simulink model "kinovaMicoSimscapeModel"  (R2021b)
(part 37 of 50)

Y1_20_3=(dq2*dqr1*cos(2*q2)*sin(2*q3))/256 - (3*dq4*dqr1*sin(2*q4)*cos(q5))/64 - (3*dq5*dqr1*sin(2*q4)*cos(q5))/64 - (3*dq5*dqr1*sin(2*q6)*cos(q5))/64 - (3*dq6*dqr1*sin(2*q6)*cos(q5))/64 - (3*dq4*dqr1*sin(2*q4))/256 - (dq2*dqr1*cos(2*q3)*sin(2*q2))/256 - (dq3*dqr1*cos(2*q2)*sin(2*q3))/256 + (dq3*dqr1*cos(2*q3)*sin(2*q2))/256 + (3*dq4*dqr1*cos(2*q4)*sin(2*q5))/64 + (15*dq4*dqr1*cos(2*q5)*sin(2*q4))/256 - (27*dq4*dqr1*cos(2*q6)*sin(2*q4))/256 - (3*dq4*dqr1*cos(2*q4)*sin(2*q6)*cos(q5))/16 - (3*dq4*dqr1*cos(2*q6)*sin(2*q4)*cos(q5))/64 - (3*dq5*dqr1*cos(2*q4)*sin(2*q6)*cos(q5))/64 - (3*dq5*dqr1*cos(2*q6)*sin(2*q4)*cos(q5))/64 - (3*dq6*dqr1*cos(2*q4)*sin(2*q6)*cos(q5))/64 - (3*dq6*dqr1*cos(2*q6)*sin(2*q4)*cos(q5))/16 - (3*dq2*dqr1*cos(2*q2)*cos(2*q4)*sin(2*q3))/256 + (3*dq2*dqr1*cos(2*q3)*cos(2*q4)*sin(2*q2))/256 + (27*dq2*dqr1*cos(2*q2)*cos(2*q5)*sin(2*q3))/256 - (27*dq2*dqr1*cos(2*q3)*cos(2*q5)*sin(2*q2))/256 + (3*dq3*dqr1*cos(2*q2)*cos(2*q4)*sin(2*q3))/256 - (3*dq3*dqr1*cos(2*q3)*cos(2*q4)*sin(2*q2))/256 + (9*dq2*dqr1*cos(2*q2)*cos(2*q6)*sin(2*q3))/256 - (9*dq2*dqr1*cos(2*q3)*cos(2*q6)*sin(2*q2))/256 - (27*dq3*dqr1*cos(2*q2)*cos(2*q5)*sin(2*q3))/256 + (27*dq3*dqr1*cos(2*q3)*cos(2*q5)*sin(2*q2))/256 + (3*dq4*dqr1*cos(2*q2)*cos(2*q3)*sin(2*q4))/256 - (9*dq3*dqr1*cos(2*q2)*cos(2*q6)*sin(2*q3))/256 + (9*dq3*dqr1*cos(2*q3)*cos(2*q6)*sin(2*q2))/256 - (5*dq4*dqr1*cos(2*q4)*cos(2*q6)*sin(2*q5))/64 - (25*dq4*dqr1*cos(2*q5)*cos(2*q6)*sin(2*q4))/256 + (3*dq4*dqr1*sin(2*q2)*sin(2*q3)*sin(2*q4))/256 + (5*dq4*dqr1*sin(2*q4)*sin(2*q5)*sin(2*q6))/64 + (15*dq2*dqr1*cos(2*q2)*cos(2*q4)*cos(2*q5)*sin(2*q3))/256 - (15*dq2*dqr1*cos(2*q3)*cos(2*q4)*cos(2*q5)*sin(2*q2))/256 - (27*dq2*dqr1*cos(2*q2)*cos(2*q4)*cos(2*q6)*sin(2*q3))/256 + (27*dq2*dqr1*cos(2*q3)*cos(2*q4)*cos(2*q6)*sin(2*q2))/256 - (15*dq3*dqr1*cos(2*q2)*cos(2*q4)*cos(2*q5)*sin(2*q3))/256 + (15*dq3*dqr1*cos(2*q3)*cos(2*q4)*cos(2*q5)*sin(2*q2))/256 - (45*dq2*dqr1*cos(2*q2)*cos(2*q5)*cos(2*q6)*sin(2*q3))/256 + (45*dq2*dqr1*cos(2*q3)*cos(2*q5)*cos(2*q6)*sin(2*q2))/256 + (27*dq3*dqr1*cos(2*q2)*cos(2*q4)*cos(2*q6)*sin(2*q3))/256 - (27*dq3*dqr1*cos(2*q3)*cos(2*q4)*cos(2*q6)*sin(2*q2))/256 - (3*dq4*dqr1*cos(2*q2)*cos(2*q3)*cos(2*q4)*sin(2*q5))/64 - (15*dq4*dqr1*cos(2*q2)*cos(2*q3)*cos(2*q5)*sin(2*q4))/256 + (45*dq3*dqr1*cos(2*q2)*cos(2*q5)*cos(2*q6)*sin(2*q3))/256 - (45*dq3*dqr1*cos(2*q3)*cos(2*q5)*cos(2*q6)*sin(2*q2))/256 + (27*dq4*dqr1*cos(2*q2)*cos(2*q3)*cos(2*q6)*sin(2*q4))/256 - (3*dq2*dqr1*cos(2*q2)*sin(2*q3)*sin(2*q4)*sin(2*q5))/64 + (3*dq2*dqr1*cos(2*q3)*sin(2*q2)*sin(2*q4)*sin(2*q5))/64 + (3*dq3*dqr1*cos(2*q2)*sin(2*q3)*sin(2*q4)*sin(2*q5))/64 - (3*dq3*dqr1*cos(2*q3)*sin(2*q2)*sin(2*q4)*sin(2*q5))/64 + (9*dq2*dqr1*cos(2*q2)*sin(2*q3)*sin(2*q5)*sin(2*q6))/64 - (9*dq2*dqr1*cos(2*q3)*sin(2*q2)*sin(2*q5)*sin(2*q6))/64 - (3*dq4*dqr1*cos(2*q4)*sin(2*q2)*sin(2*q3)*sin(2*q5))/64 - (15*dq4*dqr1*cos(2*q5)*sin(2*q2)*sin(2*q3)*sin(2*q4))/256 - (9*dq3*dqr1*cos(2*q2)*sin(2*q3)*sin(2*q5)*sin(2*q6))/64 + (9*dq3*dqr1*cos(2*q3)*sin(2*q2)*sin(2*q5)*sin(2*q6))/64 + (27*dq4*dqr1*cos(2*q6)*sin(2*q2)*sin(2*q3)*sin(2*q4))/256 + (3*dq5*dqr1*cos(2*q2)*cos(2*q3)*sin(2*q4)*cos(q5))/64 - (9*dq5*dqr1*cos(2*q2)*cos(2*q3)*sin(2*q6)*cos(q5))/64 - (9*dq6*dqr1*cos(2*q2)*cos(2*q3)*sin(2*q6)*cos(q5))/64 + (3*dq5*dqr1*sin(2*q2)*sin(2*q3)*sin(2*q4)*cos(q5))/64 - (9*dq5*dqr1*sin(2*q2)*sin(2*q3)*sin(2*q6)*cos(q5))/64 - (9*dq6*dqr1*sin(2*q2)*sin(2*q3)*sin(2*q6)*cos(q5))/64 - (25*dq2*dqr1*cos(2*q2)*cos(2*q4)*cos(2*q5)*cos(2*q6)*sin(2*q3))/256 + (25*dq2*dqr1*cos(2*q3)*cos(2*q4)*cos(2*q5)*cos(2*q6)*sin(2*q2))/256 + (25*dq3*dqr1*cos(2*q2)*cos(2*q4)*cos(2*q5)*cos(2*q6)*sin(2*q3))/256 - (25*dq3*dqr1*cos(2*q3)*cos(2*q4)*cos(2*q5)*cos(2*q6)*sin(2*q2))/256 + (dq4*dqr1*cos(2*q2)*cos(2*q3)*cos(2*q4)*cos(2*q5)*sin(2*q6))/16 + (5*dq4*dqr1*cos(2*q2)*cos(2*q3)*cos(2*q4)*cos(2*q6)*sin(2*q5))/64 + (25*dq4*dqr1*cos(2*q2)*cos(2*q3)*cos(2*q5)*cos(2*q6)*sin(2*q4))/256 + (5*dq2*dqr1*cos(2*q2)*cos(2*q4)*sin(2*q3)*sin(2*q5)*sin(2*q6))/64 + (dq2*dqr1*cos(2*q2)*cos(2*q5)*sin(2*q3)*sin(2*q4)*sin(2*q6))/16 + (5*dq2*dqr1*cos(2*q2)*cos(2*q6)*sin(2*q3)*sin(2*q4)*sin(2*q5))/64 - (5*dq2*dqr1*cos(2*q3)*cos(2*q4)*sin(2*q2)*sin(2*q5)*sin(2*q6))/64 - (dq2*dqr1*cos(2*q3)*cos(2*q5)*sin(2*q2)*sin(2*q4)*sin(2*q6))/16 - (5*dq2*dqr1*cos(2*q3)*cos(2*q6)*sin(2*q2)*sin(2*q4)*sin(2*q5))/64 - (5*dq3*dqr1*cos(2*q2)*cos(2*q4)*sin(2*q3)*sin(2*q5)*sin(2*q6))/64 - (dq3*dqr1*cos(2*q2)*cos(2*q5)*sin(2*q3)*sin(2*q4)*sin(2*q6))/16 - (5*dq3*dqr1*cos(2*q2)*cos(2*q6)*sin(2*q3)*sin(2*q4)*sin(2*q5))/64 + (5*dq3*dqr1*cos(2*q3)*cos(2*q4)*sin(2*q2)*sin(2*q5)*sin(2*q6))/64 + (dq3*dqr1*cos(2*q3)*cos(2*q5)*sin(2*q2)*sin(2*q4)*sin(2*q6))/16 + (5*dq3*dqr1*cos(2*q3)*cos(2*q6)*sin(2*q2)*sin(2*q4)*sin(2*q5))/64 - (5*dq4*dqr1*cos(2*q2)*cos(2*q3)*sin(2*q4)*sin(2*q5)*sin(2*q6))/64 + (dq4*dqr1*cos(2*q4)*cos(2*q5)*sin(2*q2)*sin(2*q3)*sin(2*q6))/16 + (5*dq4*dqr1*cos(2*q4)*cos(2*q6)*sin(2*q2)*sin(2*q3)*sin(2*q5))/64 + (25*dq4*dqr1*cos(2*q5)*cos(2*q6)*sin(2*q2)*sin(2*q3)*sin(2*q4))/256 - (5*dq4*dqr1*sin(2*q2)*sin(2*q3)*sin(2*q4)*sin(2*q5)*sin(2*q6))/64 + (3*dq4*dqr1*cos(2*q2)*cos(2*q3)*cos(2*q4)*sin(2*q6)*cos(q5))/16 + (3*dq5*dqr1*cos(2*q2)*cos(2*q3)*cos(2*q4)*sin(2*q6)*cos(q5))/64 + (3*dq5*dqr1*cos(2*q2)*cos(2*q3)*cos(2*q6)*sin(2*q4)*cos(q5))/64 + (3*dq6*dqr1*cos(2*q2)*cos(2*q3)*cos(2*q4)*sin(2*q6)*cos(q5))/64 + (3*dq6*dqr1*cos(2*q2)*cos(2*q3)*cos(2*q6)*sin(2*q4)*cos(q5))/16 + (3*dq5*dqr1*cos(2*q4)*sin(2*q2)*sin(2*q3)*sin(2*q6)*cos(q5))/64 + (3*dq5*dqr1*cos(2*q6)*sin(2*q2)*sin(2*q3)*sin(2*q4)*cos(q5))/64 + (3*dq6*dqr1*cos(2*q4)*sin(2*q2)*sin(2*q3)*sin(2*q6)*cos(q5))/64 + (3*dq6*dqr1*cos(2*q6)*sin(2*q2)*sin(2*q3)*sin(2*q4)*cos(q5))/16;
Y1_20_4=(15*dq5*dqr1*cos(2*q4)*sin(2*q5))/256 - (3*dq6*dqr1*sin(2*q6))/256 - (9*dq5*dqr1*sin(2*q5))/256 + (3*dq5*dqr1*cos(2*q5)*sin(2*q4))/64 + (3*dq5*dqr1*cos(2*q5)*sin(2*q6))/64 + (15*dq5*dqr1*cos(2*q6)*sin(2*q5))/256 - (27*dq6*dqr1*cos(2*q4)*sin(2*q6))/256 + (15*dq6*dqr1*cos(2*q5)*sin(2*q6))/256 + (3*dq6*dqr1*cos(2*q6)*sin(2*q5))/64 - (3*dq2*dqr2*sin(2*q4)*sin(q2)*sin(q3))/128 + (3*dq3*dqr2*sin(2*q4)*sin(q2)*sin(q3))/128 - (27*dq5*dqr1*cos(2*q2)*cos(2*q3)*sin(2*q5))/256 - (9*dq6*dqr1*cos(2*q2)*cos(2*q3)*sin(2*q6))/256 - (dq4*dqr1*cos(2*q4)*cos(2*q5)*sin(2*q6))/16 - (5*dq5*dqr1*cos(2*q4)*cos(2*q5)*sin(2*q6))/64 - (25*dq5*dqr1*cos(2*q4)*cos(2*q6)*sin(2*q5))/256 - (5*dq5*dqr1*cos(2*q5)*cos(2*q6)*sin(2*q4))/64 - (25*dq6*dqr1*cos(2*q4)*cos(2*q5)*sin(2*q6))/256 - (5*dq6*dqr1*cos(2*q4)*cos(2*q6)*sin(2*q5))/64 - (dq6*dqr1*cos(2*q5)*cos(2*q6)*sin(2*q4))/16 - (27*dq5*dqr1*sin(2*q2)*sin(2*q3)*sin(2*q5))/256 - (9*dq6*dqr1*sin(2*q2)*sin(2*q3)*sin(2*q6))/256 + (dq5*dqr1*sin(2*q4)*sin(2*q5)*sin(2*q6))/16 + (5*dq6*dqr1*sin(2*q4)*sin(2*q5)*sin(2*q6))/64 - (15*dq5*dqr1*cos(2*q2)*cos(2*q3)*cos(2*q4)*sin(2*q5))/256 - (3*dq5*dqr1*cos(2*q2)*cos(2*q3)*cos(2*q5)*sin(2*q4))/64 + (9*dq5*dqr1*cos(2*q2)*cos(2*q3)*cos(2*q5)*sin(2*q6))/64 + (45*dq5*dqr1*cos(2*q2)*cos(2*q3)*cos(2*q6)*sin(2*q5))/256 + (27*dq6*dqr1*cos(2*q2)*cos(2*q3)*cos(2*q4)*sin(2*q6))/256 + (45*dq6*dqr1*cos(2*q2)*cos(2*q3)*cos(2*q5)*sin(2*q6))/256 + (9*dq6*dqr1*cos(2*q2)*cos(2*q3)*cos(2*q6)*sin(2*q5))/64 - (3*dq2*dqr2*cos(2*q4)*sin(q2)*sin(q3)*sin(q5))/16 - (3*dq2*dqr2*sin(2*q4)*cos(q5)*sin(q2)*sin(q3))/32 + (3*dq3*dqr2*cos(2*q4)*sin(q2)*sin(q3)*sin(q5))/16 + (3*dq3*dqr2*sin(2*q4)*cos(q5)*sin(q2)*sin(q3))/32 - (15*dq5*dqr1*cos(2*q4)*sin(2*q2)*sin(2*q3)*sin(2*q5))/256 - (3*dq5*dqr1*cos(2*q5)*sin(2*q2)*sin(2*q3)*sin(2*q4))/64 + (9*dq5*dqr1*cos(2*q5)*sin(2*q2)*sin(2*q3)*sin(2*q6))/64 + (45*dq5*dqr1*cos(2*q6)*sin(2*q2)*sin(2*q3)*sin(2*q5))/256 + (27*dq6*dqr1*cos(2*q4)*sin(2*q2)*sin(2*q3)*sin(2*q6))/256 + (45*dq6*dqr1*cos(2*q5)*sin(2*q2)*sin(2*q3)*sin(2*q6))/256 + (9*dq6*dqr1*cos(2*q6)*sin(2*q2)*sin(2*q3)*sin(2*q5))/64 + (5*3^(1/2)*dq5*dqr2*sin(q2)*sin(q3)*sin(q4))/32 + (3^(1/2)*dq6*dqr2*sin(q2)*sin(q3)*sin(q4))/8 + (3*dq2*dqr2*cos(2*q4)*sin(2*q5)*sin(q2)*sin(q3))/32 + (15*dq2*dqr2*cos(2*q5)*sin(2*q4)*sin(q2)*sin(q3))/128 - (27*dq2*dqr2*cos(2*q6)*sin(2*q4)*sin(q2)*sin(q3))/128 - (15*dq3*dqr2*cos(2*q5)*sin(2*q4)*sin(q2)*sin(q3))/128 + (27*dq3*dqr2*cos(2*q6)*sin(2*q4)*sin(q2)*sin(q3))/128 - (3*3^(1/2)*dq5*dqr2*cos(q4)*sin(q2)*sin(q3)*sin(q5))/32 - (3^(1/2)*dq6*dqr2*cos(q4)*sin(q2)*sin(q3)*sin(q5))/4 - (3^(1/2)*dq6*dqr2*cos(q5)*sin(q2)*sin(q3)*sin(q4))/8 + (5*dq5*dqr1*cos(2*q2)*cos(2*q3)*cos(2*q4)*cos(2*q5)*sin(2*q6))/64 + (25*dq5*dqr1*cos(2*q2)*cos(2*q3)*cos(2*q4)*cos(2*q6)*sin(2*q5))/256 + (5*dq5*dqr1*cos(2*q2)*cos(2*q3)*cos(2*q5)*cos(2*q6)*sin(2*q4))/64 + (25*dq6*dqr1*cos(2*q2)*cos(2*q3)*cos(2*q4)*cos(2*q5)*sin(2*q6))/256 + (5*dq6*dqr1*cos(2*q2)*cos(2*q3)*cos(2*q4)*cos(2*q6)*sin(2*q5))/64 + (dq6*dqr1*cos(2*q2)*cos(2*q3)*cos(2*q5)*cos(2*q6)*sin(2*q4))/16 - (3*dq2*dqr2*cos(2*q4)*cos(2*q6)*sin(q2)*sin(q3)*sin(q5))/16 - (3*dq2*dqr2*cos(2*q4)*sin(2*q6)*cos(q5)*sin(q2)*sin(q3))/8 - (3*dq2*dqr2*cos(2*q6)*sin(2*q4)*cos(q5)*sin(q2)*sin(q3))/32 + (3*dq3*dqr2*cos(2*q4)*cos(2*q6)*sin(q2)*sin(q3)*sin(q5))/16 + (3*dq3*dqr2*cos(2*q4)*sin(2*q6)*cos(q5)*sin(q2)*sin(q3))/8 + (3*dq3*dqr2*cos(2*q6)*sin(2*q4)*cos(q5)*sin(q2)*sin(q3))/32 - (dq5*dqr1*cos(2*q2)*cos(2*q3)*sin(2*q4)*sin(2*q5)*sin(2*q6))/16 + (5*dq5*dqr1*cos(2*q4)*cos(2*q5)*sin(2*q2)*sin(2*q3)*sin(2*q6))/64 + (25*dq5*dqr1*cos(2*q4)*cos(2*q6)*sin(2*q2)*sin(2*q3)*sin(2*q5))/256 + (5*dq5*dqr1*cos(2*q5)*cos(2*q6)*sin(2*q2)*sin(2*q3)*sin(2*q4))/64 - (5*dq6*dqr1*cos(2*q2)*cos(2*q3)*sin(2*q4)*sin(2*q5)*sin(2*q6))/64 + (25*dq6*dqr1*cos(2*q4)*cos(2*q5)*sin(2*q2)*sin(2*q3)*sin(2*q6))/256 + (5*dq6*dqr1*cos(2*q4)*cos(2*q6)*sin(2*q2)*sin(2*q3)*sin(2*q5))/64 + (dq6*dqr1*cos(2*q5)*cos(2*q6)*sin(2*q2)*sin(2*q3)*sin(2*q4))/16 + (3*dq2*dqr2*sin(2*q4)*sin(2*q6)*sin(q2)*sin(q3)*sin(q5))/16 - (3*dq3*dqr2*sin(2*q4)*sin(2*q6)*sin(q2)*sin(q3)*sin(q5))/16 + (3*3^(1/2)*dq5*dqr2*cos(2*q5)*sin(q2)*sin(q3)*sin(q4))/32 + (3*3^(1/2)*dq5*dqr2*sin(2*q5)*cos(q4)*sin(q2)*sin(q3))/64 - (3*3^(1/2)*dq5*dqr2*cos(2*q6)*sin(q2)*sin(q3)*sin(q4))/32 + (9*3^(1/2)*dq6*dqr2*sin(2*q6)*cos(q4)*sin(q2)*sin(q3))/64 - (dq5*dqr1*sin(2*q2)*sin(2*q3)*sin(2*q4)*sin(2*q5)*sin(2*q6))/16 - (5*dq6*dqr1*sin(2*q2)*sin(2*q3)*sin(2*q4)*sin(2*q5)*sin(2*q6))/64 - (dq2*dqr2*cos(2*q4)*cos(2*q5)*sin(2*q6)*sin(q2)*sin(q3))/8 - (5*dq2*dqr2*cos(2*q4)*cos(2*q6)*sin(2*q5)*sin(q2)*sin(q3))/32 - (25*dq2*dqr2*cos(2*q5)*cos(2*q6)*sin(2*q4)*sin(q2)*sin(q3))/128 + (25*dq3*dqr2*cos(2*q5)*cos(2*q6)*sin(2*q4)*sin(q2)*sin(q3))/128 + (5*dq2*dqr2*sin(2*q4)*sin(2*q5)*sin(2*q6)*sin(q2)*sin(q3))/32 - (5*dq3*dqr2*sin(2*q4)*sin(2*q5)*sin(2*q6)*sin(q2)*sin(q3))/32 - (3*3^(1/2)*dq5*dqr2*cos(2*q6)*cos(q4)*sin(q2)*sin(q3)*sin(q5))/32 - (3*3^(1/2)*dq5*dqr2*sin(2*q6)*cos(q4)*cos(q5)*sin(q2)*sin(q3))/16 - (3^(1/2)*dq6*dqr2*cos(2*q6)*cos(q4)*sin(q2)*sin(q3)*sin(q5))/8 + (3^(1/2)*dq6*dqr2*cos(2*q6)*cos(q5)*sin(q2)*sin(q3)*sin(q4))/8 - (3^(1/2)*dq6*dqr2*sin(2*q6)*cos(q4)*cos(q5)*sin(q2)*sin(q3))/16 - (3^(1/2)*dq6*dqr2*sin(2*q6)*sin(q2)*sin(q3)*sin(q4)*sin(q5))/16 - (5*3^(1/2)*dq5*dqr2*cos(2*q5)*cos(2*q6)*sin(q2)*sin(q3)*sin(q4))/32 - (3^(1/2)*dq5*dqr2*cos(2*q5)*sin(2*q6)*cos(q4)*sin(q2)*sin(q3))/16 - (5*3^(1/2)*dq5*dqr2*cos(2*q6)*sin(2*q5)*cos(q4)*sin(q2)*sin(q3))/64 - (3^(1/2)*dq6*dqr2*cos(2*q5)*cos(2*q6)*sin(q2)*sin(q3)*sin(q4))/8 - (5*3^(1/2)*dq6*dqr2*cos(2*q5)*sin(2*q6)*cos(q4)*sin(q2)*sin(q3))/64 - (3^(1/2)*dq6*dqr2*cos(2*q6)*sin(2*q5)*cos(q4)*sin(q2)*sin(q3))/16 + (3^(1/2)*dq5*dqr2*sin(2*q5)*sin(2*q6)*sin(q2)*sin(q3)*sin(q4))/8 + (5*3^(1/2)*dq6*dqr2*sin(2*q5)*sin(2*q6)*sin(q2)*sin(q3)*sin(q4))/32;
Y1_20_5=(3*dq5*dqr2*cos(2*q6)*cos(q3)*sin(q2))/32 - (5*dq5*dqr2*cos(q3)*sin(q2))/32 - (dq6*dqr2*cos(q3)*sin(q2))/8 - (3*dq4*dqr2*cos(2*q4)*cos(q3)*sin(q2))/128 - (9*dq4*dqr2*cos(2*q5)*cos(q3)*sin(q2))/128 - (3*dq4*dqr2*cos(2*q6)*cos(q3)*sin(q2))/128 - (43*dq4*dqr2*cos(q3)*sin(q2))/128 - (3*dq4*dqr2*cos(q3)*cos(q5)*sin(q2))/32 - (3*dq5*dqr2*cos(q3)*cos(q5)*sin(q2))/32 - (3*dq6*dqr2*cos(q3)*cos(q5)*sin(q2))/8 - (3*dq4*dqr2*sin(2*q4)*cos(q2)*sin(q3)*sin(q5))/16 + (3*dq4*dqr2*sin(2*q4)*cos(q3)*sin(q2)*sin(q5))/16 + (3*dq5*dqr2*sin(2*q4)*cos(q3)*sin(q2)*sin(q5))/64 - (3*dq4*dqr2*sin(2*q6)*cos(q2)*sin(q3)*sin(q5))/16 + (3*dq4*dqr2*sin(2*q6)*cos(q3)*sin(q2)*sin(q5))/16 + (3*dq5*dqr2*sin(2*q6)*cos(q3)*sin(q2)*sin(q5))/16 + (3^(1/2)*dq2*dqr2*cos(q3)*cos(q4)*sin(q2))/64 - (3^(1/2)*dq3*dqr2*cos(q3)*cos(q4)*sin(q2))/64 + (15*dq4*dqr2*cos(2*q4)*cos(2*q5)*cos(q3)*sin(q2))/128 - (27*dq4*dqr2*cos(2*q4)*cos(2*q6)*cos(q3)*sin(q2))/128 + (3*dq5*dqr2*cos(2*q4)*cos(2*q5)*cos(q3)*sin(q2))/32 + (15*dq4*dqr2*cos(2*q5)*cos(2*q6)*cos(q3)*sin(q2))/128 - (3*dq3*dqr2*cos(2*q4)*sin(2*q5)*sin(q2)*sin(q3))/32 - (3*dq4*dqr2*sin(2*q4)*sin(2*q5)*cos(q3)*sin(q2))/32 - (15*dq5*dqr2*sin(2*q4)*sin(2*q5)*cos(q3)*sin(q2))/128 - (3*dq4*dqr2*sin(2*q5)*sin(2*q6)*cos(q3)*sin(q2))/32 + (27*dq6*dqr2*sin(2*q4)*sin(2*q6)*cos(q3)*sin(q2))/128 - (3*dq4*dqr2*cos(2*q4)*cos(q3)*cos(q5)*sin(q2))/32 - (3*dq5*dqr2*cos(2*q4)*cos(q3)*cos(q5)*sin(q2))/32 - (3*dq4*dqr2*cos(2*q6)*cos(q3)*cos(q5)*sin(q2))/32 - (3*dq5*dqr2*cos(2*q6)*cos(q3)*cos(q5)*sin(q2))/32 + (3^(1/2)*dq2*dqr2*cos(q2)*sin(q3)*sin(q4)*sin(q5))/16 - (3^(1/2)*dq2*dqr2*cos(q3)*sin(q2)*sin(q4)*sin(q5))/16 - (3^(1/2)*dq3*dqr2*cos(q2)*sin(q3)*sin(q4)*sin(q5))/16 + (3^(1/2)*dq3*dqr2*cos(q3)*sin(q2)*sin(q4)*sin(q5))/16 - (3*dq4*dqr2*cos(2*q4)*cos(2*q6)*cos(q3)*cos(q5)*sin(q2))/32 - (3*dq5*dqr2*cos(2*q4)*cos(2*q6)*cos(q3)*cos(q5)*sin(q2))/32 - (3*dq6*dqr2*cos(2*q4)*cos(2*q6)*cos(q3)*cos(q5)*sin(q2))/8 - (3*dq4*dqr2*cos(2*q4)*sin(2*q6)*cos(q2)*sin(q3)*sin(q5))/16 + (3*dq4*dqr2*cos(2*q4)*sin(2*q6)*cos(q3)*sin(q2)*sin(q5))/16 - (3*dq4*dqr2*cos(2*q6)*sin(2*q4)*cos(q2)*sin(q3)*sin(q5))/16 + (3*dq4*dqr2*cos(2*q6)*sin(2*q4)*cos(q3)*sin(q2)*sin(q5))/16 + (3*dq4*dqr2*sin(2*q4)*sin(2*q6)*cos(q3)*cos(q5)*sin(q2))/8 + (3*dq5*dqr2*cos(2*q4)*sin(2*q6)*cos(q3)*sin(q2)*sin(q5))/16 - (3*dq5*dqr2*cos(2*q6)*sin(2*q4)*cos(q2)*sin(q3)*sin(q5))/64 + (3*dq5*dqr2*cos(2*q6)*sin(2*q4)*cos(q3)*sin(q2)*sin(q5))/64 + (3*dq5*dqr2*sin(2*q4)*sin(2*q6)*cos(q3)*cos(q5)*sin(q2))/32 + (3*dq6*dqr2*cos(2*q4)*sin(2*q6)*cos(q3)*sin(q2)*sin(q5))/16 + (3*dq6*dqr2*cos(2*q6)*sin(2*q4)*cos(q3)*sin(q2)*sin(q5))/16 + (3*dq6*dqr2*sin(2*q4)*sin(2*q6)*cos(q3)*cos(q5)*sin(q2))/32 + (3*3^(1/2)*dq2*dqr2*cos(2*q5)*cos(q3)*cos(q4)*sin(q2))/64 + (9*3^(1/2)*dq2*dqr2*cos(2*q6)*cos(q3)*cos(q4)*sin(q2))/64 - (3*3^(1/2)*dq3*dqr2*cos(2*q5)*cos(q3)*cos(q4)*sin(q2))/64 - (9*3^(1/2)*dq3*dqr2*cos(2*q6)*cos(q3)*cos(q4)*sin(q2))/64 + (3*3^(1/2)*dq2*dqr2*sin(2*q5)*cos(q2)*sin(q3)*sin(q4))/32 - (3*3^(1/2)*dq2*dqr2*sin(2*q5)*cos(q3)*sin(q2)*sin(q4))/32 - (3*3^(1/2)*dq3*dqr2*sin(2*q5)*cos(q2)*sin(q3)*sin(q4))/32 + (3*3^(1/2)*dq3*dqr2*sin(2*q5)*cos(q3)*sin(q2)*sin(q4))/32 - (25*dq4*dqr2*cos(2*q4)*cos(2*q5)*cos(2*q6)*cos(q3)*sin(q2))/128 - (5*dq5*dqr2*cos(2*q4)*cos(2*q5)*cos(2*q6)*cos(q3)*sin(q2))/32 - (dq6*dqr2*cos(2*q4)*cos(2*q5)*cos(2*q6)*cos(q3)*sin(q2))/8 + (dq3*dqr2*cos(2*q4)*cos(2*q5)*sin(2*q6)*sin(q2)*sin(q3))/8 + (5*dq3*dqr2*cos(2*q4)*cos(2*q6)*sin(2*q5)*sin(q2)*sin(q3))/32 + (5*dq4*dqr2*cos(2*q4)*sin(2*q5)*sin(2*q6)*cos(q3)*sin(q2))/32 + (dq4*dqr2*cos(2*q5)*sin(2*q4)*sin(2*q6)*cos(q3)*sin(q2))/8 + (5*dq4*dqr2*cos(2*q6)*sin(2*q4)*sin(2*q5)*cos(q3)*sin(q2))/32 + (dq5*dqr2*cos(2*q4)*sin(2*q5)*sin(2*q6)*cos(q3)*sin(q2))/8 + (5*dq5*dqr2*cos(2*q5)*sin(2*q4)*sin(2*q6)*cos(q3)*sin(q2))/32 + (25*dq5*dqr2*cos(2*q6)*sin(2*q4)*sin(2*q5)*cos(q3)*sin(q2))/128 + (5*dq6*dqr2*cos(2*q4)*sin(2*q5)*sin(2*q6)*cos(q3)*sin(q2))/32 + (25*dq6*dqr2*cos(2*q5)*sin(2*q4)*sin(2*q6)*cos(q3)*sin(q2))/128 + (5*dq6*dqr2*cos(2*q6)*sin(2*q4)*sin(2*q5)*cos(q3)*sin(q2))/32 - (3^(1/2)*dq2*dqr2*cos(q3)*cos(q4)*cos(q5)*sin(q2))/16 + (3^(1/2)*dq3*dqr2*cos(q3)*cos(q4)*cos(q5)*sin(q2))/16 - (3^(1/2)*dq2*dqr2*cos(2*q6)*cos(q3)*cos(q4)*cos(q5)*sin(q2))/16 + (3^(1/2)*dq3*dqr2*cos(2*q6)*cos(q3)*cos(q4)*cos(q5)*sin(q2))/16 + (3^(1/2)*dq2*dqr2*cos(2*q6)*cos(q2)*sin(q3)*sin(q4)*sin(q5))/16 - (3^(1/2)*dq2*dqr2*cos(2*q6)*cos(q3)*sin(q2)*sin(q4)*sin(q5))/16 - (3^(1/2)*dq2*dqr2*sin(2*q6)*cos(q2)*cos(q4)*sin(q3)*sin(q5))/8 + (3^(1/2)*dq2*dqr2*sin(2*q6)*cos(q2)*cos(q5)*sin(q3)*sin(q4))/8 + (3^(1/2)*dq2*dqr2*sin(2*q6)*cos(q3)*cos(q4)*sin(q2)*sin(q5))/8 - (3^(1/2)*dq2*dqr2*sin(2*q6)*cos(q3)*cos(q5)*sin(q2)*sin(q4))/8 - (3^(1/2)*dq3*dqr2*cos(2*q6)*cos(q2)*sin(q3)*sin(q4)*sin(q5))/16 + (3^(1/2)*dq3*dqr2*cos(2*q6)*cos(q3)*sin(q2)*sin(q4)*sin(q5))/16 + (3^(1/2)*dq3*dqr2*sin(2*q6)*cos(q2)*cos(q4)*sin(q3)*sin(q5))/8 - (3^(1/2)*dq3*dqr2*sin(2*q6)*cos(q2)*cos(q5)*sin(q3)*sin(q4))/8 - (3^(1/2)*dq3*dqr2*sin(2*q6)*cos(q3)*cos(q4)*sin(q2)*sin(q5))/8 + (3^(1/2)*dq3*dqr2*sin(2*q6)*cos(q3)*cos(q5)*sin(q2)*sin(q4))/8 - (5*3^(1/2)*dq2*dqr2*cos(2*q5)*cos(2*q6)*cos(q3)*cos(q4)*sin(q2))/64 + (5*3^(1/2)*dq3*dqr2*cos(2*q5)*cos(2*q6)*cos(q3)*cos(q4)*sin(q2))/64 - (3^(1/2)*dq2*dqr2*cos(2*q5)*sin(2*q6)*cos(q2)*sin(q3)*sin(q4))/8 + (3^(1/2)*dq2*dqr2*cos(2*q5)*sin(2*q6)*cos(q3)*sin(q2)*sin(q4))/8 - (5*3^(1/2)*dq2*dqr2*cos(2*q6)*sin(2*q5)*cos(q2)*sin(q3)*sin(q4))/32 + (5*3^(1/2)*dq2*dqr2*cos(2*q6)*sin(2*q5)*cos(q3)*sin(q2)*sin(q4))/32 + (3^(1/2)*dq2*dqr2*sin(2*q5)*sin(2*q6)*cos(q3)*cos(q4)*sin(q2))/16 + (3^(1/2)*dq3*dqr2*cos(2*q5)*sin(2*q6)*cos(q2)*sin(q3)*sin(q4))/8 - (3^(1/2)*dq3*dqr2*cos(2*q5)*sin(2*q6)*cos(q3)*sin(q2)*sin(q4))/8 + (5*3^(1/2)*dq3*dqr2*cos(2*q6)*sin(2*q5)*cos(q2)*sin(q3)*sin(q4))/32 - (5*3^(1/2)*dq3*dqr2*cos(2*q6)*sin(2*q5)*cos(q3)*sin(q2)*sin(q4))/32 - (3^(1/2)*dq3*dqr2*sin(2*q5)*sin(2*q6)*cos(q3)*cos(q4)*sin(q2))/16;
Y1_20_6=(43*dq4*dqr2*cos(q2)*sin(q3))/128 + (5*dq5*dqr2*cos(q2)*sin(q3))/32 + (dq6*dqr2*cos(q2)*sin(q3))/8 + (3*dq4*dqr2*cos(2*q4)*cos(q2)*sin(q3))/128 + (9*dq4*dqr2*cos(2*q5)*cos(q2)*sin(q3))/128 + (3*dq4*dqr2*cos(2*q6)*cos(q2)*sin(q3))/128 - (3*dq5*dqr2*cos(2*q6)*cos(q2)*sin(q3))/32 + (3*dq4*dqr2*cos(q2)*cos(q5)*sin(q3))/32 + (3*dq5*dqr2*cos(q2)*cos(q5)*sin(q3))/32 + (3*dq6*dqr2*cos(q2)*cos(q5)*sin(q3))/8 - (3*dq5*dqr2*sin(2*q4)*cos(q2)*sin(q3)*sin(q5))/64 - (3*dq5*dqr2*sin(2*q6)*cos(q2)*sin(q3)*sin(q5))/16 - (3^(1/2)*dq2*dqr2*cos(q2)*cos(q4)*sin(q3))/64 + (3^(1/2)*dq3*dqr2*cos(q2)*cos(q4)*sin(q3))/64 + (5*3^(1/2)*dq5*dqr2*cos(q2)*cos(q3)*sin(q4))/32 + (3^(1/2)*dq6*dqr2*cos(q2)*cos(q3)*sin(q4))/8 - (15*dq4*dqr2*cos(2*q4)*cos(2*q5)*cos(q2)*sin(q3))/128 + (27*dq4*dqr2*cos(2*q4)*cos(2*q6)*cos(q2)*sin(q3))/128 - (3*dq5*dqr2*cos(2*q4)*cos(2*q5)*cos(q2)*sin(q3))/32 - (15*dq4*dqr2*cos(2*q5)*cos(2*q6)*cos(q2)*sin(q3))/128 + (3*dq4*dqr2*sin(2*q4)*sin(2*q5)*cos(q2)*sin(q3))/32 + (15*dq5*dqr2*sin(2*q4)*sin(2*q5)*cos(q2)*sin(q3))/128 + (3*dq4*dqr2*sin(2*q5)*sin(2*q6)*cos(q2)*sin(q3))/32 - (27*dq6*dqr2*sin(2*q4)*sin(2*q6)*cos(q2)*sin(q3))/128 - (3^(1/2)*dq1*dqr2*cos(2*q2)*cos(2*q3)*sin(q4))/64 - (3*dq2*dqr2*cos(2*q4)*cos(q2)*cos(q3)*sin(q5))/16 + (3*dq3*dqr2*cos(2*q4)*cos(q2)*cos(q3)*sin(q5))/16 + (3*dq4*dqr2*cos(2*q4)*cos(q2)*cos(q5)*sin(q3))/32 + (3*dq5*dqr2*cos(2*q4)*cos(q2)*cos(q5)*sin(q3))/32 + (3*dq4*dqr2*cos(2*q6)*cos(q2)*cos(q5)*sin(q3))/32 + (3*dq5*dqr2*cos(2*q6)*cos(q2)*cos(q5)*sin(q3))/32 - (3^(1/2)*dq1*dqr2*sin(2*q2)*sin(2*q3)*sin(q4))/64 - (3*3^(1/2)*dq1*dqr2*cos(2*q2)*cos(2*q3)*cos(2*q5)*sin(q4))/64 - (9*3^(1/2)*dq1*dqr2*cos(2*q2)*cos(2*q3)*cos(2*q6)*sin(q4))/64 - (3*dq2*dqr2*cos(2*q4)*cos(2*q6)*cos(q2)*cos(q3)*sin(q5))/16 + (3*dq3*dqr2*cos(2*q4)*cos(2*q6)*cos(q2)*cos(q3)*sin(q5))/16 + (3*dq4*dqr2*cos(2*q4)*cos(2*q6)*cos(q2)*cos(q5)*sin(q3))/32 + (3*dq5*dqr2*cos(2*q4)*cos(2*q6)*cos(q2)*cos(q5)*sin(q3))/32 + (3*dq6*dqr2*cos(2*q4)*cos(2*q6)*cos(q2)*cos(q5)*sin(q3))/8 - (3*3^(1/2)*dq1*dqr2*cos(2*q5)*sin(2*q2)*sin(2*q3)*sin(q4))/64 - (9*3^(1/2)*dq1*dqr2*cos(2*q6)*sin(2*q2)*sin(2*q3)*sin(q4))/64 + (3*dq2*dqr2*sin(2*q4)*sin(2*q6)*cos(q2)*cos(q3)*sin(q5))/16 - (3*dq3*dqr2*sin(2*q4)*sin(2*q6)*cos(q2)*cos(q3)*sin(q5))/16 - (3*dq4*dqr2*sin(2*q4)*sin(2*q6)*cos(q2)*cos(q5)*sin(q3))/8 - (3*dq5*dqr2*cos(2*q4)*sin(2*q6)*cos(q2)*sin(q3)*sin(q5))/16 - (3*dq5*dqr2*sin(2*q4)*sin(2*q6)*cos(q2)*cos(q5)*sin(q3))/32 - (3*dq6*dqr2*cos(2*q4)*sin(2*q6)*cos(q2)*sin(q3)*sin(q5))/16 - (3*dq6*dqr2*cos(2*q6)*sin(2*q4)*cos(q2)*sin(q3)*sin(q5))/16 - (3*dq6*dqr2*sin(2*q4)*sin(2*q6)*cos(q2)*cos(q5)*sin(q3))/32 - (3*3^(1/2)*dq2*dqr2*cos(2*q5)*cos(q2)*cos(q4)*sin(q3))/64 - (9*3^(1/2)*dq2*dqr2*cos(2*q6)*cos(q2)*cos(q4)*sin(q3))/64 + (3*3^(1/2)*dq3*dqr2*cos(2*q5)*cos(q2)*cos(q4)*sin(q3))/64 + (9*3^(1/2)*dq3*dqr2*cos(2*q6)*cos(q2)*cos(q4)*sin(q3))/64 + (3*3^(1/2)*dq5*dqr2*cos(2*q5)*cos(q2)*cos(q3)*sin(q4))/32 - (3*3^(1/2)*dq5*dqr2*cos(2*q6)*cos(q2)*cos(q3)*sin(q4))/32 + (25*dq4*dqr2*cos(2*q4)*cos(2*q5)*cos(2*q6)*cos(q2)*sin(q3))/128 + (5*dq5*dqr2*cos(2*q4)*cos(2*q5)*cos(2*q6)*cos(q2)*sin(q3))/32 + (dq6*dqr2*cos(2*q4)*cos(2*q5)*cos(2*q6)*cos(q2)*sin(q3))/8 - (5*dq4*dqr2*cos(2*q4)*sin(2*q5)*sin(2*q6)*cos(q2)*sin(q3))/32 - (dq4*dqr2*cos(2*q5)*sin(2*q4)*sin(2*q6)*cos(q2)*sin(q3))/8 - (5*dq4*dqr2*cos(2*q6)*sin(2*q4)*sin(2*q5)*cos(q2)*sin(q3))/32 - (dq5*dqr2*cos(2*q4)*sin(2*q5)*sin(2*q6)*cos(q2)*sin(q3))/8 - (5*dq5*dqr2*cos(2*q5)*sin(2*q4)*sin(2*q6)*cos(q2)*sin(q3))/32 - (25*dq5*dqr2*cos(2*q6)*sin(2*q4)*sin(2*q5)*cos(q2)*sin(q3))/128 - (5*dq6*dqr2*cos(2*q4)*sin(2*q5)*sin(2*q6)*cos(q2)*sin(q3))/32 - (25*dq6*dqr2*cos(2*q5)*sin(2*q4)*sin(2*q6)*cos(q2)*sin(q3))/128 - (5*dq6*dqr2*cos(2*q6)*sin(2*q4)*sin(2*q5)*cos(q2)*sin(q3))/32 - (3^(1/2)*dq1*dqr2*cos(2*q2)*cos(2*q3)*cos(q4)*sin(q5))/16 + (3^(1/2)*dq1*dqr2*cos(2*q2)*cos(2*q3)*cos(q5)*sin(q4))/16 - (3^(1/2)*dq1*dqr2*sin(2*q2)*sin(2*q3)*cos(q4)*sin(q5))/16 + (3^(1/2)*dq1*dqr2*sin(2*q2)*sin(2*q3)*cos(q5)*sin(q4))/16 + (3^(1/2)*dq2*dqr2*cos(q2)*cos(q4)*cos(q5)*sin(q3))/16 - (3^(1/2)*dq3*dqr2*cos(q2)*cos(q4)*cos(q5)*sin(q3))/16 - (3*3^(1/2)*dq5*dqr2*cos(q2)*cos(q3)*cos(q4)*sin(q5))/32 - (3^(1/2)*dq6*dqr2*cos(q2)*cos(q3)*cos(q4)*sin(q5))/4 - (3^(1/2)*dq6*dqr2*cos(q2)*cos(q3)*cos(q5)*sin(q4))/8 - (3^(1/2)*dq1*dqr2*sin(2*q2)*sin(2*q3)*sin(2*q6)*sin(q4)*sin(q5))/8 + (3^(1/2)*dq2*dqr2*cos(2*q6)*cos(q2)*cos(q4)*cos(q5)*sin(q3))/16 - (3^(1/2)*dq3*dqr2*cos(2*q6)*cos(q2)*cos(q4)*cos(q5)*sin(q3))/16 - (3*3^(1/2)*dq5*dqr2*cos(2*q6)*cos(q2)*cos(q3)*cos(q4)*sin(q5))/32 - (3^(1/2)*dq6*dqr2*cos(2*q6)*cos(q2)*cos(q3)*cos(q4)*sin(q5))/8 + (3^(1/2)*dq6*dqr2*cos(2*q6)*cos(q2)*cos(q3)*cos(q5)*sin(q4))/8 + (5*3^(1/2)*dq1*dqr2*cos(2*q2)*cos(2*q3)*cos(2*q5)*cos(2*q6)*sin(q4))/64 - (3^(1/2)*dq6*dqr2*sin(2*q6)*cos(q2)*cos(q3)*sin(q4)*sin(q5))/16 - (3^(1/2)*dq1*dqr2*cos(2*q2)*cos(2*q3)*sin(2*q5)*sin(2*q6)*sin(q4))/16 + (5*3^(1/2)*dq1*dqr2*cos(2*q5)*cos(2*q6)*sin(2*q2)*sin(2*q3)*sin(q4))/64 - (3^(1/2)*dq1*dqr2*sin(2*q2)*sin(2*q3)*sin(2*q5)*sin(2*q6)*sin(q4))/16 + (5*3^(1/2)*dq2*dqr2*cos(2*q5)*cos(2*q6)*cos(q2)*cos(q4)*sin(q3))/64 - (5*3^(1/2)*dq3*dqr2*cos(2*q5)*cos(2*q6)*cos(q2)*cos(q4)*sin(q3))/64 - (5*3^(1/2)*dq5*dqr2*cos(2*q5)*cos(2*q6)*cos(q2)*cos(q3)*sin(q4))/32 - (3^(1/2)*dq6*dqr2*cos(2*q5)*cos(2*q6)*cos(q2)*cos(q3)*sin(q4))/8 - (3^(1/2)*dq2*dqr2*sin(2*q5)*sin(2*q6)*cos(q2)*cos(q4)*sin(q3))/16 + (3^(1/2)*dq3*dqr2*sin(2*q5)*sin(2*q6)*cos(q2)*cos(q4)*sin(q3))/16 + (3^(1/2)*dq5*dqr2*sin(2*q5)*sin(2*q6)*cos(q2)*cos(q3)*sin(q4))/8 + (5*3^(1/2)*dq6*dqr2*sin(2*q5)*sin(2*q6)*cos(q2)*cos(q3)*sin(q4))/32 - (3^(1/2)*dq1*dqr2*cos(2*q2)*cos(2*q3)*cos(2*q6)*cos(q4)*sin(q5))/16 + (3^(1/2)*dq1*dqr2*cos(2*q2)*cos(2*q3)*cos(2*q6)*cos(q5)*sin(q4))/16 - (3^(1/2)*dq1*dqr2*cos(2*q2)*cos(2*q3)*sin(2*q6)*sin(q4)*sin(q5))/8 - (3^(1/2)*dq1*dqr2*cos(2*q6)*sin(2*q2)*sin(2*q3)*cos(q4)*sin(q5))/16 + (3^(1/2)*dq1*dqr2*cos(2*q6)*sin(2*q2)*sin(2*q3)*cos(q5)*sin(q4))/16;
Y1_20_7=(dq1*dqr2*cos(2*q2)*sin(2*q3))/256 - (dq1*dqr2*cos(2*q3)*sin(2*q2))/256 - (3*dq2*dqr2*sin(2*q4)*cos(q2)*cos(q3))/128 + (3*dq3*dqr2*sin(2*q4)*cos(q2)*cos(q3))/128 + (9*dq1*dqr2*cos(2*q2)*sin(2*q3)*cos(q5))/64 - (9*dq1*dqr2*cos(2*q3)*sin(2*q2)*cos(q5))/64 - (3*dq1*dqr2*cos(2*q2)*cos(2*q4)*sin(2*q3))/256 + (3*dq1*dqr2*cos(2*q3)*cos(2*q4)*sin(2*q2))/256 + (27*dq1*dqr2*cos(2*q2)*cos(2*q5)*sin(2*q3))/256 - (27*dq1*dqr2*cos(2*q3)*cos(2*q5)*sin(2*q2))/256 + (9*dq1*dqr2*cos(2*q2)*cos(2*q6)*sin(2*q3))/256 - (9*dq1*dqr2*cos(2*q3)*cos(2*q6)*sin(2*q2))/256 + (15*dq1*dqr2*cos(2*q2)*cos(2*q4)*cos(2*q5)*sin(2*q3))/256 - (15*dq1*dqr2*cos(2*q3)*cos(2*q4)*cos(2*q5)*sin(2*q2))/256 - (27*dq1*dqr2*cos(2*q2)*cos(2*q4)*cos(2*q6)*sin(2*q3))/256 + (27*dq1*dqr2*cos(2*q3)*cos(2*q4)*cos(2*q6)*sin(2*q2))/256 - (45*dq1*dqr2*cos(2*q2)*cos(2*q5)*cos(2*q6)*sin(2*q3))/256 + (45*dq1*dqr2*cos(2*q3)*cos(2*q5)*cos(2*q6)*sin(2*q2))/256 + (3*dq2*dqr3*cos(2*q4)*sin(q2)*sin(q3)*sin(q5))/16 - (3*dq1*dqr2*cos(2*q2)*sin(2*q3)*sin(2*q4)*sin(2*q5))/64 + (3*dq1*dqr2*cos(2*q3)*sin(2*q2)*sin(2*q4)*sin(2*q5))/64 + (9*dq1*dqr2*cos(2*q2)*sin(2*q3)*sin(2*q5)*sin(2*q6))/64 - (9*dq1*dqr2*cos(2*q3)*sin(2*q2)*sin(2*q5)*sin(2*q6))/64 - (5*3^(1/2)*dq5*dqr3*sin(q2)*sin(q3)*sin(q4))/32 - (3^(1/2)*dq6*dqr3*sin(q2)*sin(q3)*sin(q4))/8 + (3*dq2*dqr2*cos(2*q4)*sin(2*q5)*cos(q2)*cos(q3))/32 + (15*dq2*dqr2*cos(2*q5)*sin(2*q4)*cos(q2)*cos(q3))/128 - (27*dq2*dqr2*cos(2*q6)*sin(2*q4)*cos(q2)*cos(q3))/128 - (3*dq3*dqr2*cos(2*q4)*sin(2*q5)*cos(q2)*cos(q3))/32 - (15*dq3*dqr2*cos(2*q5)*sin(2*q4)*cos(q2)*cos(q3))/128 + (27*dq3*dqr2*cos(2*q6)*sin(2*q4)*cos(q2)*cos(q3))/128 - (3*dq1*dqr2*cos(2*q2)*cos(2*q4)*sin(2*q3)*cos(q5))/64 + (3*dq1*dqr2*cos(2*q3)*cos(2*q4)*sin(2*q2)*cos(q5))/64 + (9*dq1*dqr2*cos(2*q2)*cos(2*q6)*sin(2*q3)*cos(q5))/64 - (9*dq1*dqr2*cos(2*q3)*cos(2*q6)*sin(2*q2)*cos(q5))/64 + (3*dq1*dqr2*cos(2*q2)*sin(2*q3)*sin(2*q4)*sin(q5))/32 - (3*dq1*dqr2*cos(2*q3)*sin(2*q2)*sin(2*q4)*sin(q5))/32 - (9*dq1*dqr2*cos(2*q2)*sin(2*q3)*sin(2*q6)*sin(q5))/32 + (9*dq1*dqr2*cos(2*q3)*sin(2*q2)*sin(2*q6)*sin(q5))/32 - (3*dq2*dqr2*sin(2*q4)*cos(q2)*cos(q3)*cos(q5))/32 + (3*dq3*dqr2*sin(2*q4)*cos(q2)*cos(q3)*cos(q5))/32 - (3*3^(1/2)*dq1*dqr2*cos(2*q2)*cos(2*q3)*sin(2*q5)*cos(q4))/32 + (3*3^(1/2)*dq5*dqr3*cos(q4)*sin(q2)*sin(q3)*sin(q5))/32 + (3^(1/2)*dq6*dqr3*cos(q4)*sin(q2)*sin(q3)*sin(q5))/4 + (3^(1/2)*dq6*dqr3*cos(q5)*sin(q2)*sin(q3)*sin(q4))/8 - (3*dq2*dqr2*cos(2*q4)*sin(2*q6)*cos(q2)*cos(q3)*cos(q5))/8 - (3*dq2*dqr2*cos(2*q6)*sin(2*q4)*cos(q2)*cos(q3)*cos(q5))/32 + (3*dq3*dqr2*cos(2*q4)*sin(2*q6)*cos(q2)*cos(q3)*cos(q5))/8 + (3*dq3*dqr2*cos(2*q6)*sin(2*q4)*cos(q2)*cos(q3)*cos(q5))/32 - (3*3^(1/2)*dq1*dqr2*sin(2*q2)*sin(2*q3)*sin(2*q5)*cos(q4))/32 - (25*dq1*dqr2*cos(2*q2)*cos(2*q4)*cos(2*q5)*cos(2*q6)*sin(2*q3))/256 + (25*dq1*dqr2*cos(2*q3)*cos(2*q4)*cos(2*q5)*cos(2*q6)*sin(2*q2))/256 + (3*dq2*dqr3*cos(2*q4)*cos(2*q6)*sin(q2)*sin(q3)*sin(q5))/16 + (3*3^(1/2)*dq5*dqr2*sin(2*q5)*cos(q2)*cos(q3)*cos(q4))/64 + (9*3^(1/2)*dq6*dqr2*sin(2*q6)*cos(q2)*cos(q3)*cos(q4))/64 + (5*dq1*dqr2*cos(2*q2)*cos(2*q4)*sin(2*q3)*sin(2*q5)*sin(2*q6))/64 + (dq1*dqr2*cos(2*q2)*cos(2*q5)*sin(2*q3)*sin(2*q4)*sin(2*q6))/16 + (5*dq1*dqr2*cos(2*q2)*cos(2*q6)*sin(2*q3)*sin(2*q4)*sin(2*q5))/64 - (5*dq1*dqr2*cos(2*q3)*cos(2*q4)*sin(2*q2)*sin(2*q5)*sin(2*q6))/64 - (dq1*dqr2*cos(2*q3)*cos(2*q5)*sin(2*q2)*sin(2*q4)*sin(2*q6))/16 - (5*dq1*dqr2*cos(2*q3)*cos(2*q6)*sin(2*q2)*sin(2*q4)*sin(2*q5))/64 - (3*dq2*dqr3*sin(2*q4)*sin(2*q6)*sin(q2)*sin(q3)*sin(q5))/16 - (3*3^(1/2)*dq5*dqr3*cos(2*q5)*sin(q2)*sin(q3)*sin(q4))/32 + (3*3^(1/2)*dq5*dqr3*cos(2*q6)*sin(q2)*sin(q3)*sin(q4))/32 - (dq2*dqr2*cos(2*q4)*cos(2*q5)*sin(2*q6)*cos(q2)*cos(q3))/8 - (5*dq2*dqr2*cos(2*q4)*cos(2*q6)*sin(2*q5)*cos(q2)*cos(q3))/32 - (25*dq2*dqr2*cos(2*q5)*cos(2*q6)*sin(2*q4)*cos(q2)*cos(q3))/128 + (dq3*dqr2*cos(2*q4)*cos(2*q5)*sin(2*q6)*cos(q2)*cos(q3))/8 + (5*dq3*dqr2*cos(2*q4)*cos(2*q6)*sin(2*q5)*cos(q2)*cos(q3))/32 + (25*dq3*dqr2*cos(2*q5)*cos(2*q6)*sin(2*q4)*cos(q2)*cos(q3))/128 + (5*dq2*dqr2*sin(2*q4)*sin(2*q5)*sin(2*q6)*cos(q2)*cos(q3))/32 - (5*dq3*dqr2*sin(2*q4)*sin(2*q5)*sin(2*q6)*cos(q2)*cos(q3))/32 - (3*dq1*dqr2*cos(2*q2)*cos(2*q4)*cos(2*q6)*sin(2*q3)*cos(q5))/64 + (3*dq1*dqr2*cos(2*q3)*cos(2*q4)*cos(2*q6)*sin(2*q2)*cos(q5))/64 + (3*dq1*dqr2*cos(2*q2)*cos(2*q4)*sin(2*q3)*sin(2*q6)*sin(q5))/32 + (3*dq1*dqr2*cos(2*q2)*cos(2*q6)*sin(2*q3)*sin(2*q4)*sin(q5))/32 + (3*dq1*dqr2*cos(2*q2)*sin(2*q3)*sin(2*q4)*sin(2*q6)*cos(q5))/16 - (3*dq1*dqr2*cos(2*q3)*cos(2*q4)*sin(2*q2)*sin(2*q6)*sin(q5))/32 - (3*dq1*dqr2*cos(2*q3)*cos(2*q6)*sin(2*q2)*sin(2*q4)*sin(q5))/32 - (3*dq1*dqr2*cos(2*q3)*sin(2*q2)*sin(2*q4)*sin(2*q6)*cos(q5))/16 - (3*3^(1/2)*dq5*dqr2*sin(2*q6)*cos(q2)*cos(q3)*cos(q4)*cos(q5))/16 - (3^(1/2)*dq6*dqr2*sin(2*q6)*cos(q2)*cos(q3)*cos(q4)*cos(q5))/16 + (3^(1/2)*dq1*dqr2*cos(2*q2)*cos(2*q3)*cos(2*q5)*sin(2*q6)*cos(q4))/8 + (5*3^(1/2)*dq1*dqr2*cos(2*q2)*cos(2*q3)*cos(2*q6)*sin(2*q5)*cos(q4))/32 + (3*3^(1/2)*dq5*dqr3*cos(2*q6)*cos(q4)*sin(q2)*sin(q3)*sin(q5))/32 + (3^(1/2)*dq6*dqr3*cos(2*q6)*cos(q4)*sin(q2)*sin(q3)*sin(q5))/8 - (3^(1/2)*dq6*dqr3*cos(2*q6)*cos(q5)*sin(q2)*sin(q3)*sin(q4))/8 + (3^(1/2)*dq1*dqr2*cos(2*q5)*sin(2*q2)*sin(2*q3)*sin(2*q6)*cos(q4))/8 + (5*3^(1/2)*dq1*dqr2*cos(2*q6)*sin(2*q2)*sin(2*q3)*sin(2*q5)*cos(q4))/32 + (3^(1/2)*dq6*dqr3*sin(2*q6)*sin(q2)*sin(q3)*sin(q4)*sin(q5))/16 - (3^(1/2)*dq5*dqr2*cos(2*q5)*sin(2*q6)*cos(q2)*cos(q3)*cos(q4))/16 - (5*3^(1/2)*dq5*dqr2*cos(2*q6)*sin(2*q5)*cos(q2)*cos(q3)*cos(q4))/64 - (5*3^(1/2)*dq6*dqr2*cos(2*q5)*sin(2*q6)*cos(q2)*cos(q3)*cos(q4))/64 - (3^(1/2)*dq6*dqr2*cos(2*q6)*sin(2*q5)*cos(q2)*cos(q3)*cos(q4))/16 + (5*3^(1/2)*dq5*dqr3*cos(2*q5)*cos(2*q6)*sin(q2)*sin(q3)*sin(q4))/32 + (3^(1/2)*dq6*dqr3*cos(2*q5)*cos(2*q6)*sin(q2)*sin(q3)*sin(q4))/8 - (3^(1/2)*dq5*dqr3*sin(2*q5)*sin(2*q6)*sin(q2)*sin(q3)*sin(q4))/8 - (5*3^(1/2)*dq6*dqr3*sin(2*q5)*sin(2*q6)*sin(q2)*sin(q3)*sin(q4))/32 - (3^(1/2)*dq1*dqr2*cos(2*q2)*cos(2*q3)*sin(2*q6)*cos(q4)*cos(q5))/8 - (3^(1/2)*dq1*dqr2*sin(2*q2)*sin(2*q3)*sin(2*q6)*cos(q4)*cos(q5))/8;
Y1_20_8=(43*dq4*dqr3*cos(q3)*sin(q2))/128 + (3*dq4*dqr3*cos(2*q4)*cos(q3)*sin(q2))/128 + (9*dq4*dqr3*cos(2*q5)*cos(q3)*sin(q2))/128 + (3*dq4*dqr3*cos(2*q6)*cos(q3)*sin(q2))/128 + (3*dq2*dqr3*sin(2*q4)*sin(q2)*sin(q3))/128 - (3*dq3*dqr3*sin(2*q4)*sin(q2)*sin(q3))/128 + (3*dq4*dqr3*cos(q3)*cos(q5)*sin(q2))/32 + (3*dq5*dqr3*cos(q3)*cos(q5)*sin(q2))/32 + (3*dq6*dqr3*cos(q3)*cos(q5)*sin(q2))/8 + (3*dq2*dqr3*sin(2*q4)*cos(q5)*sin(q2)*sin(q3))/32 - (3*dq3*dqr3*cos(2*q4)*sin(q2)*sin(q3)*sin(q5))/16 - (3*dq3*dqr3*sin(2*q4)*cos(q5)*sin(q2)*sin(q3))/32 - (3*dq4*dqr3*sin(2*q4)*cos(q3)*sin(q2)*sin(q5))/16 - (3*dq5*dqr3*sin(2*q4)*cos(q3)*sin(q2)*sin(q5))/64 - (3*dq4*dqr3*sin(2*q6)*cos(q3)*sin(q2)*sin(q5))/16 - (3*dq5*dqr3*sin(2*q6)*cos(q3)*sin(q2)*sin(q5))/16 - (3^(1/2)*dq2*dqr3*cos(q3)*cos(q4)*sin(q2))/64 + (3^(1/2)*dq3*dqr3*cos(q3)*cos(q4)*sin(q2))/64 - (15*dq4*dqr3*cos(2*q4)*cos(2*q5)*cos(q3)*sin(q2))/128 + (27*dq4*dqr3*cos(2*q4)*cos(2*q6)*cos(q3)*sin(q2))/128 - (15*dq4*dqr3*cos(2*q5)*cos(2*q6)*cos(q3)*sin(q2))/128 - (3*dq2*dqr3*cos(2*q4)*sin(2*q5)*sin(q2)*sin(q3))/32 - (15*dq2*dqr3*cos(2*q5)*sin(2*q4)*sin(q2)*sin(q3))/128 + (27*dq2*dqr3*cos(2*q6)*sin(2*q4)*sin(q2)*sin(q3))/128 + (3*dq3*dqr3*cos(2*q4)*sin(2*q5)*sin(q2)*sin(q3))/32 + (15*dq3*dqr3*cos(2*q5)*sin(2*q4)*sin(q2)*sin(q3))/128 - (27*dq3*dqr3*cos(2*q6)*sin(2*q4)*sin(q2)*sin(q3))/128 + (3*dq4*dqr3*sin(2*q4)*sin(2*q5)*cos(q3)*sin(q2))/32 + (15*dq5*dqr3*sin(2*q4)*sin(2*q5)*cos(q3)*sin(q2))/128 + (3*dq4*dqr3*sin(2*q5)*sin(2*q6)*cos(q3)*sin(q2))/32 + (3*dq4*dqr3*cos(2*q4)*cos(q3)*cos(q5)*sin(q2))/32 + (3*dq5*dqr3*cos(2*q4)*cos(q3)*cos(q5)*sin(q2))/32 + (3*dq4*dqr3*cos(2*q6)*cos(q3)*cos(q5)*sin(q2))/32 + (3*dq5*dqr3*cos(2*q6)*cos(q3)*cos(q5)*sin(q2))/32 + (3^(1/2)*dq2*dqr3*cos(q3)*sin(q2)*sin(q4)*sin(q5))/16 - (3^(1/2)*dq3*dqr3*cos(q3)*sin(q2)*sin(q4)*sin(q5))/16 + (3*dq4*dqr3*cos(2*q4)*cos(2*q6)*cos(q3)*cos(q5)*sin(q2))/32 + (3*dq5*dqr3*cos(2*q4)*cos(2*q6)*cos(q3)*cos(q5)*sin(q2))/32 + (3*dq6*dqr3*cos(2*q4)*cos(2*q6)*cos(q3)*cos(q5)*sin(q2))/8 + (3*dq2*dqr3*cos(2*q4)*sin(2*q6)*cos(q5)*sin(q2)*sin(q3))/8 + (3*dq2*dqr3*cos(2*q6)*sin(2*q4)*cos(q5)*sin(q2)*sin(q3))/32 - (3*dq3*dqr3*cos(2*q4)*cos(2*q6)*sin(q2)*sin(q3)*sin(q5))/16 - (3*dq3*dqr3*cos(2*q4)*sin(2*q6)*cos(q5)*sin(q2)*sin(q3))/8 - (3*dq3*dqr3*cos(2*q6)*sin(2*q4)*cos(q5)*sin(q2)*sin(q3))/32 - (3*dq4*dqr3*cos(2*q4)*sin(2*q6)*cos(q3)*sin(q2)*sin(q5))/16 - (3*dq4*dqr3*cos(2*q6)*sin(2*q4)*cos(q3)*sin(q2)*sin(q5))/16 - (3*dq4*dqr3*sin(2*q4)*sin(2*q6)*cos(q3)*cos(q5)*sin(q2))/8 - (3*dq5*dqr3*cos(2*q4)*sin(2*q6)*cos(q3)*sin(q2)*sin(q5))/16 - (3*dq5*dqr3*cos(2*q6)*sin(2*q4)*cos(q3)*sin(q2)*sin(q5))/64 - (3*dq5*dqr3*sin(2*q4)*sin(2*q6)*cos(q3)*cos(q5)*sin(q2))/32 - (3*dq6*dqr3*cos(2*q4)*sin(2*q6)*cos(q3)*sin(q2)*sin(q5))/16 - (3*dq6*dqr3*cos(2*q6)*sin(2*q4)*cos(q3)*sin(q2)*sin(q5))/16 - (3*dq6*dqr3*sin(2*q4)*sin(2*q6)*cos(q3)*cos(q5)*sin(q2))/32 - (3*3^(1/2)*dq2*dqr3*cos(2*q5)*cos(q3)*cos(q4)*sin(q2))/64 - (9*3^(1/2)*dq2*dqr3*cos(2*q6)*cos(q3)*cos(q4)*sin(q2))/64 + (3*3^(1/2)*dq3*dqr3*cos(2*q5)*cos(q3)*cos(q4)*sin(q2))/64 + (9*3^(1/2)*dq3*dqr3*cos(2*q6)*cos(q3)*cos(q4)*sin(q2))/64 + (3*dq3*dqr3*sin(2*q4)*sin(2*q6)*sin(q2)*sin(q3)*sin(q5))/16 + (3*3^(1/2)*dq2*dqr3*sin(2*q5)*cos(q3)*sin(q2)*sin(q4))/32 - (3*3^(1/2)*dq3*dqr3*sin(2*q5)*cos(q3)*sin(q2)*sin(q4))/32 - (3*3^(1/2)*dq5*dqr3*sin(2*q5)*cos(q4)*sin(q2)*sin(q3))/64 - (9*3^(1/2)*dq6*dqr3*sin(2*q6)*cos(q4)*sin(q2)*sin(q3))/64 + (25*dq4*dqr3*cos(2*q4)*cos(2*q5)*cos(2*q6)*cos(q3)*sin(q2))/128 + (dq2*dqr3*cos(2*q4)*cos(2*q5)*sin(2*q6)*sin(q2)*sin(q3))/8 + (5*dq2*dqr3*cos(2*q4)*cos(2*q6)*sin(2*q5)*sin(q2)*sin(q3))/32 + (25*dq2*dqr3*cos(2*q5)*cos(2*q6)*sin(2*q4)*sin(q2)*sin(q3))/128 - (dq3*dqr3*cos(2*q4)*cos(2*q5)*sin(2*q6)*sin(q2)*sin(q3))/8 - (5*dq3*dqr3*cos(2*q4)*cos(2*q6)*sin(2*q5)*sin(q2)*sin(q3))/32 - (25*dq3*dqr3*cos(2*q5)*cos(2*q6)*sin(2*q4)*sin(q2)*sin(q3))/128 - (5*dq4*dqr3*cos(2*q4)*sin(2*q5)*sin(2*q6)*cos(q3)*sin(q2))/32 - (dq4*dqr3*cos(2*q5)*sin(2*q4)*sin(2*q6)*cos(q3)*sin(q2))/8 - (5*dq4*dqr3*cos(2*q6)*sin(2*q4)*sin(2*q5)*cos(q3)*sin(q2))/32 - (5*dq5*dqr3*cos(2*q5)*sin(2*q4)*sin(2*q6)*cos(q3)*sin(q2))/32 - (25*dq5*dqr3*cos(2*q6)*sin(2*q4)*sin(2*q5)*cos(q3)*sin(q2))/128 - (5*dq2*dqr3*sin(2*q4)*sin(2*q5)*sin(2*q6)*sin(q2)*sin(q3))/32 + (5*dq3*dqr3*sin(2*q4)*sin(2*q5)*sin(2*q6)*sin(q2)*sin(q3))/32 + (3^(1/2)*dq2*dqr3*cos(q3)*cos(q4)*cos(q5)*sin(q2))/16 - (3^(1/2)*dq3*dqr3*cos(q3)*cos(q4)*cos(q5)*sin(q2))/16 + (3^(1/2)*dq2*dqr3*cos(2*q6)*cos(q3)*cos(q4)*cos(q5)*sin(q2))/16 - (3^(1/2)*dq3*dqr3*cos(2*q6)*cos(q3)*cos(q4)*cos(q5)*sin(q2))/16 + (3^(1/2)*dq2*dqr3*cos(2*q6)*cos(q3)*sin(q2)*sin(q4)*sin(q5))/16 - (3^(1/2)*dq2*dqr3*sin(2*q6)*cos(q3)*cos(q4)*sin(q2)*sin(q5))/8 + (3^(1/2)*dq2*dqr3*sin(2*q6)*cos(q3)*cos(q5)*sin(q2)*sin(q4))/8 - (3^(1/2)*dq3*dqr3*cos(2*q6)*cos(q3)*sin(q2)*sin(q4)*sin(q5))/16 + (3^(1/2)*dq3*dqr3*sin(2*q6)*cos(q3)*cos(q4)*sin(q2)*sin(q5))/8 - (3^(1/2)*dq3*dqr3*sin(2*q6)*cos(q3)*cos(q5)*sin(q2)*sin(q4))/8 + (3*3^(1/2)*dq5*dqr3*sin(2*q6)*cos(q4)*cos(q5)*sin(q2)*sin(q3))/16 + (3^(1/2)*dq6*dqr3*sin(2*q6)*cos(q4)*cos(q5)*sin(q2)*sin(q3))/16 + (5*3^(1/2)*dq2*dqr3*cos(2*q5)*cos(2*q6)*cos(q3)*cos(q4)*sin(q2))/64 - (5*3^(1/2)*dq3*dqr3*cos(2*q5)*cos(2*q6)*cos(q3)*cos(q4)*sin(q2))/64 - (3^(1/2)*dq2*dqr3*cos(2*q5)*sin(2*q6)*cos(q3)*sin(q2)*sin(q4))/8 - (5*3^(1/2)*dq2*dqr3*cos(2*q6)*sin(2*q5)*cos(q3)*sin(q2)*sin(q4))/32 - (3^(1/2)*dq2*dqr3*sin(2*q5)*sin(2*q6)*cos(q3)*cos(q4)*sin(q2))/16 + (3^(1/2)*dq3*dqr3*cos(2*q5)*sin(2*q6)*cos(q3)*sin(q2)*sin(q4))/8 + (5*3^(1/2)*dq3*dqr3*cos(2*q6)*sin(2*q5)*cos(q3)*sin(q2)*sin(q4))/32 + (3^(1/2)*dq3*dqr3*sin(2*q5)*sin(2*q6)*cos(q3)*cos(q4)*sin(q2))/16 + (3^(1/2)*dq5*dqr3*cos(2*q5)*sin(2*q6)*cos(q4)*sin(q2)*sin(q3))/16 + (5*3^(1/2)*dq5*dqr3*cos(2*q6)*sin(2*q5)*cos(q4)*sin(q2)*sin(q3))/64 + (5*3^(1/2)*dq6*dqr3*cos(2*q5)*sin(2*q6)*cos(q4)*sin(q2)*sin(q3))/64 + (3^(1/2)*dq6*dqr3*cos(2*q6)*sin(2*q5)*cos(q4)*sin(q2)*sin(q3))/16;
Y1_20_9=(5*dq5*dqr3*cos(q3)*sin(q2))/32 - (5*dq5*dqr3*cos(q2)*sin(q3))/32 - (43*dq4*dqr3*cos(q2)*sin(q3))/128 - (dq6*dqr3*cos(q2)*sin(q3))/8 + (dq6*dqr3*cos(q3)*sin(q2))/8 - (3*dq4*dqr3*cos(2*q4)*cos(q2)*sin(q3))/128 - (9*dq4*dqr3*cos(2*q5)*cos(q2)*sin(q3))/128 - (3*dq4*dqr3*cos(2*q6)*cos(q2)*sin(q3))/128 + (3*dq5*dqr3*cos(2*q6)*cos(q2)*sin(q3))/32 - (3*dq5*dqr3*cos(2*q6)*cos(q3)*sin(q2))/32 - (3*dq4*dqr3*cos(q2)*cos(q5)*sin(q3))/32 - (3*dq5*dqr3*cos(q2)*cos(q5)*sin(q3))/32 - (3*dq6*dqr3*cos(q2)*cos(q5)*sin(q3))/8 + (3*dq4*dqr3*sin(2*q4)*cos(q2)*sin(q3)*sin(q5))/16 + (3*dq5*dqr3*sin(2*q4)*cos(q2)*sin(q3)*sin(q5))/64 + (3*dq4*dqr3*sin(2*q6)*cos(q2)*sin(q3)*sin(q5))/16 + (3*dq5*dqr3*sin(2*q6)*cos(q2)*sin(q3)*sin(q5))/16 + (3^(1/2)*dq2*dqr3*cos(q2)*cos(q4)*sin(q3))/64 - (3^(1/2)*dq3*dqr3*cos(q2)*cos(q4)*sin(q3))/64 - (5*3^(1/2)*dq5*dqr3*cos(q2)*cos(q3)*sin(q4))/32 + (15*dq4*dqr3*cos(2*q4)*cos(2*q5)*cos(q2)*sin(q3))/128 - (27*dq4*dqr3*cos(2*q4)*cos(2*q6)*cos(q2)*sin(q3))/128 + (3*dq5*dqr3*cos(2*q4)*cos(2*q5)*cos(q2)*sin(q3))/32 - (3*dq5*dqr3*cos(2*q4)*cos(2*q5)*cos(q3)*sin(q2))/32 + (15*dq4*dqr3*cos(2*q5)*cos(2*q6)*cos(q2)*sin(q3))/128 - (3*dq4*dqr3*sin(2*q4)*sin(2*q5)*cos(q2)*sin(q3))/32 - (15*dq5*dqr3*sin(2*q4)*sin(2*q5)*cos(q2)*sin(q3))/128 - (3*dq4*dqr3*sin(2*q5)*sin(2*q6)*cos(q2)*sin(q3))/32 + (27*dq6*dqr3*sin(2*q4)*sin(2*q6)*cos(q2)*sin(q3))/128 - (27*dq6*dqr3*sin(2*q4)*sin(2*q6)*cos(q3)*sin(q2))/128 - (3*dq4*dqr3*cos(2*q4)*cos(q2)*cos(q5)*sin(q3))/32 - (3*dq5*dqr3*cos(2*q4)*cos(q2)*cos(q5)*sin(q3))/32 - (3*dq4*dqr3*cos(2*q6)*cos(q2)*cos(q5)*sin(q3))/32 - (3*dq5*dqr3*cos(2*q6)*cos(q2)*cos(q5)*sin(q3))/32 - (3^(1/2)*dq2*dqr3*cos(q2)*sin(q3)*sin(q4)*sin(q5))/16 + (3^(1/2)*dq3*dqr3*cos(q2)*sin(q3)*sin(q4)*sin(q5))/16 - (3*dq4*dqr3*cos(2*q4)*cos(2*q6)*cos(q2)*cos(q5)*sin(q3))/32 - (3*dq5*dqr3*cos(2*q4)*cos(2*q6)*cos(q2)*cos(q5)*sin(q3))/32 - (3*dq6*dqr3*cos(2*q4)*cos(2*q6)*cos(q2)*cos(q5)*sin(q3))/8 + (3*dq4*dqr3*cos(2*q4)*sin(2*q6)*cos(q2)*sin(q3)*sin(q5))/16 + (3*dq4*dqr3*cos(2*q6)*sin(2*q4)*cos(q2)*sin(q3)*sin(q5))/16 + (3*dq4*dqr3*sin(2*q4)*sin(2*q6)*cos(q2)*cos(q5)*sin(q3))/8 + (3*dq5*dqr3*cos(2*q4)*sin(2*q6)*cos(q2)*sin(q3)*sin(q5))/16 + (3*dq5*dqr3*cos(2*q6)*sin(2*q4)*cos(q2)*sin(q3)*sin(q5))/64 + (3*dq5*dqr3*sin(2*q4)*sin(2*q6)*cos(q2)*cos(q5)*sin(q3))/32 + (3*dq6*dqr3*cos(2*q4)*sin(2*q6)*cos(q2)*sin(q3)*sin(q5))/16 + (3*dq6*dqr3*cos(2*q6)*sin(2*q4)*cos(q2)*sin(q3)*sin(q5))/16 + (3*dq6*dqr3*sin(2*q4)*sin(2*q6)*cos(q2)*cos(q5)*sin(q3))/32 + (3*3^(1/2)*dq2*dqr3*cos(2*q5)*cos(q2)*cos(q4)*sin(q3))/64 + (9*3^(1/2)*dq2*dqr3*cos(2*q6)*cos(q2)*cos(q4)*sin(q3))/64 - (3*3^(1/2)*dq3*dqr3*cos(2*q5)*cos(q2)*cos(q4)*sin(q3))/64 - (9*3^(1/2)*dq3*dqr3*cos(2*q6)*cos(q2)*cos(q4)*sin(q3))/64 - (3*3^(1/2)*dq5*dqr3*cos(2*q5)*cos(q2)*cos(q3)*sin(q4))/32 + (3*3^(1/2)*dq5*dqr3*cos(2*q6)*cos(q2)*cos(q3)*sin(q4))/32 - (3*3^(1/2)*dq2*dqr3*sin(2*q5)*cos(q2)*sin(q3)*sin(q4))/32 + (3*3^(1/2)*dq3*dqr3*sin(2*q5)*cos(q2)*sin(q3)*sin(q4))/32 - (25*dq4*dqr3*cos(2*q4)*cos(2*q5)*cos(2*q6)*cos(q2)*sin(q3))/128 - (5*dq5*dqr3*cos(2*q4)*cos(2*q5)*cos(2*q6)*cos(q2)*sin(q3))/32 + (5*dq5*dqr3*cos(2*q4)*cos(2*q5)*cos(2*q6)*cos(q3)*sin(q2))/32 - (dq6*dqr3*cos(2*q4)*cos(2*q5)*cos(2*q6)*cos(q2)*sin(q3))/8 + (dq6*dqr3*cos(2*q4)*cos(2*q5)*cos(2*q6)*cos(q3)*sin(q2))/8 + (5*dq4*dqr3*cos(2*q4)*sin(2*q5)*sin(2*q6)*cos(q2)*sin(q3))/32 + (dq4*dqr3*cos(2*q5)*sin(2*q4)*sin(2*q6)*cos(q2)*sin(q3))/8 + (5*dq4*dqr3*cos(2*q6)*sin(2*q4)*sin(2*q5)*cos(q2)*sin(q3))/32 + (dq5*dqr3*cos(2*q4)*sin(2*q5)*sin(2*q6)*cos(q2)*sin(q3))/8 - (dq5*dqr3*cos(2*q4)*sin(2*q5)*sin(2*q6)*cos(q3)*sin(q2))/8 + (5*dq5*dqr3*cos(2*q5)*sin(2*q4)*sin(2*q6)*cos(q2)*sin(q3))/32 + (25*dq5*dqr3*cos(2*q6)*sin(2*q4)*sin(2*q5)*cos(q2)*sin(q3))/128 + (5*dq6*dqr3*cos(2*q4)*sin(2*q5)*sin(2*q6)*cos(q2)*sin(q3))/32 - (5*dq6*dqr3*cos(2*q4)*sin(2*q5)*sin(2*q6)*cos(q3)*sin(q2))/32 + (25*dq6*dqr3*cos(2*q5)*sin(2*q4)*sin(2*q6)*cos(q2)*sin(q3))/128 - (25*dq6*dqr3*cos(2*q5)*sin(2*q4)*sin(2*q6)*cos(q3)*sin(q2))/128 + (5*dq6*dqr3*cos(2*q6)*sin(2*q4)*sin(2*q5)*cos(q2)*sin(q3))/32 - (5*dq6*dqr3*cos(2*q6)*sin(2*q4)*sin(2*q5)*cos(q3)*sin(q2))/32 - (3^(1/2)*dq2*dqr3*cos(q2)*cos(q4)*cos(q5)*sin(q3))/16 + (3^(1/2)*dq3*dqr3*cos(q2)*cos(q4)*cos(q5)*sin(q3))/16 + (3^(1/2)*dq6*dqr3*cos(q2)*cos(q3)*cos(q5)*sin(q4))/8 + (3^(1/2)*dq1*dqr3*sin(2*q2)*sin(2*q3)*sin(2*q6)*sin(q4)*sin(q5))/8 - (3^(1/2)*dq2*dqr3*cos(2*q6)*cos(q2)*cos(q4)*cos(q5)*sin(q3))/16 + (3^(1/2)*dq3*dqr3*cos(2*q6)*cos(q2)*cos(q4)*cos(q5)*sin(q3))/16 - (3^(1/2)*dq6*dqr3*cos(2*q6)*cos(q2)*cos(q3)*cos(q5)*sin(q4))/8 - (3^(1/2)*dq2*dqr3*cos(2*q6)*cos(q2)*sin(q3)*sin(q4)*sin(q5))/16 + (3^(1/2)*dq2*dqr3*sin(2*q6)*cos(q2)*cos(q4)*sin(q3)*sin(q5))/8 - (3^(1/2)*dq2*dqr3*sin(2*q6)*cos(q2)*cos(q5)*sin(q3)*sin(q4))/8 + (3^(1/2)*dq3*dqr3*cos(2*q6)*cos(q2)*sin(q3)*sin(q4)*sin(q5))/16 - (3^(1/2)*dq3*dqr3*sin(2*q6)*cos(q2)*cos(q4)*sin(q3)*sin(q5))/8 + (3^(1/2)*dq3*dqr3*sin(2*q6)*cos(q2)*cos(q5)*sin(q3)*sin(q4))/8 + (3^(1/2)*dq6*dqr3*sin(2*q6)*cos(q2)*cos(q3)*sin(q4)*sin(q5))/16 - (5*3^(1/2)*dq2*dqr3*cos(2*q5)*cos(2*q6)*cos(q2)*cos(q4)*sin(q3))/64 + (5*3^(1/2)*dq3*dqr3*cos(2*q5)*cos(2*q6)*cos(q2)*cos(q4)*sin(q3))/64 + (5*3^(1/2)*dq5*dqr3*cos(2*q5)*cos(2*q6)*cos(q2)*cos(q3)*sin(q4))/32 + (3^(1/2)*dq2*dqr3*cos(2*q5)*sin(2*q6)*cos(q2)*sin(q3)*sin(q4))/8 + (5*3^(1/2)*dq2*dqr3*cos(2*q6)*sin(2*q5)*cos(q2)*sin(q3)*sin(q4))/32 + (3^(1/2)*dq2*dqr3*sin(2*q5)*sin(2*q6)*cos(q2)*cos(q4)*sin(q3))/16 - (3^(1/2)*dq3*dqr3*cos(2*q5)*sin(2*q6)*cos(q2)*sin(q3)*sin(q4))/8 - (5*3^(1/2)*dq3*dqr3*cos(2*q6)*sin(2*q5)*cos(q2)*sin(q3)*sin(q4))/32 - (3^(1/2)*dq3*dqr3*sin(2*q5)*sin(2*q6)*cos(q2)*cos(q4)*sin(q3))/16 - (3^(1/2)*dq5*dqr3*sin(2*q5)*sin(2*q6)*cos(q2)*cos(q3)*sin(q4))/8 - (5*3^(1/2)*dq6*dqr3*sin(2*q5)*sin(2*q6)*cos(q2)*cos(q3)*sin(q4))/32 + (3^(1/2)*dq1*dqr3*cos(2*q2)*cos(2*q3)*sin(2*q6)*sin(q4)*sin(q5))/8;
Y1_20_10=(dq1*dqr3*cos(2*q3)*sin(2*q2))/256 + (3*dq2*dqr3*sin(2*q4)*cos(q2)*cos(q3))/128 - (3*dq3*dqr3*sin(2*q4)*cos(q2)*cos(q3))/128 - (9*dq1*dqr3*cos(2*q2)*sin(2*q3)*cos(q5))/64 + (9*dq1*dqr3*cos(2*q3)*sin(2*q2)*cos(q5))/64 - (3*dq1*dqr3*cos(2*q3)*cos(2*q4)*sin(2*q2))/256 + (27*dq1*dqr3*cos(2*q3)*cos(2*q5)*sin(2*q2))/256 + (9*dq1*dqr3*cos(2*q3)*cos(2*q6)*sin(2*q2))/256 + (15*dq1*dqr3*cos(2*q3)*cos(2*q4)*cos(2*q5)*sin(2*q2))/256 - (27*dq1*dqr3*cos(2*q3)*cos(2*q4)*cos(2*q6)*sin(2*q2))/256 - (45*dq1*dqr3*cos(2*q3)*cos(2*q5)*cos(2*q6)*sin(2*q2))/256 - (3^(1/2)*dq6*dqr3*cos(q2)*cos(q3)*sin(q4))/8 - (3*dq1*dqr3*cos(2*q3)*sin(2*q2)*sin(2*q4)*sin(2*q5))/64 + (9*dq1*dqr3*cos(2*q3)*sin(2*q2)*sin(2*q5)*sin(2*q6))/64 - (3*dq2*dqr3*cos(2*q4)*sin(2*q5)*cos(q2)*cos(q3))/32 - (15*dq2*dqr3*cos(2*q5)*sin(2*q4)*cos(q2)*cos(q3))/128 + (27*dq2*dqr3*cos(2*q6)*sin(2*q4)*cos(q2)*cos(q3))/128 + (3*dq3*dqr3*cos(2*q4)*sin(2*q5)*cos(q2)*cos(q3))/32 + (15*dq3*dqr3*cos(2*q5)*sin(2*q4)*cos(q2)*cos(q3))/128 - (27*dq3*dqr3*cos(2*q6)*sin(2*q4)*cos(q2)*cos(q3))/128 + (3*dq1*dqr3*cos(2*q2)*cos(2*q4)*sin(2*q3)*cos(q5))/64 - (3*dq1*dqr3*cos(2*q3)*cos(2*q4)*sin(2*q2)*cos(q5))/64 - (9*dq1*dqr3*cos(2*q2)*cos(2*q6)*sin(2*q3)*cos(q5))/64 + (9*dq1*dqr3*cos(2*q3)*cos(2*q6)*sin(2*q2)*cos(q5))/64 - (3*dq1*dqr3*cos(2*q2)*sin(2*q3)*sin(2*q4)*sin(q5))/32 + (3*dq1*dqr3*cos(2*q3)*sin(2*q2)*sin(2*q4)*sin(q5))/32 + (9*dq1*dqr3*cos(2*q2)*sin(2*q3)*sin(2*q6)*sin(q5))/32 - (9*dq1*dqr3*cos(2*q3)*sin(2*q2)*sin(2*q6)*sin(q5))/32 + (3^(1/2)*dq1*dqr3*cos(2*q2)*cos(2*q3)*sin(q4))/64 + (3*dq2*dqr3*cos(2*q4)*cos(q2)*cos(q3)*sin(q5))/16 + (3*dq2*dqr3*sin(2*q4)*cos(q2)*cos(q3)*cos(q5))/32 - (3*dq3*dqr3*cos(2*q4)*cos(q2)*cos(q3)*sin(q5))/16 - (3*dq3*dqr3*sin(2*q4)*cos(q2)*cos(q3)*cos(q5))/32 + (3^(1/2)*dq1*dqr3*sin(2*q2)*sin(2*q3)*sin(q4))/64 + (3*3^(1/2)*dq1*dqr3*cos(2*q2)*cos(2*q3)*cos(2*q5)*sin(q4))/64 + (3*3^(1/2)*dq1*dqr3*cos(2*q2)*cos(2*q3)*sin(2*q5)*cos(q4))/32 + (9*3^(1/2)*dq1*dqr3*cos(2*q2)*cos(2*q3)*cos(2*q6)*sin(q4))/64 + (3*dq2*dqr3*cos(2*q4)*cos(2*q6)*cos(q2)*cos(q3)*sin(q5))/16 + (3*dq2*dqr3*cos(2*q4)*sin(2*q6)*cos(q2)*cos(q3)*cos(q5))/8 + (3*dq2*dqr3*cos(2*q6)*sin(2*q4)*cos(q2)*cos(q3)*cos(q5))/32 - (3*dq3*dqr3*cos(2*q4)*cos(2*q6)*cos(q2)*cos(q3)*sin(q5))/16 - (3*dq3*dqr3*cos(2*q4)*sin(2*q6)*cos(q2)*cos(q3)*cos(q5))/8 - (3*dq3*dqr3*cos(2*q6)*sin(2*q4)*cos(q2)*cos(q3)*cos(q5))/32 + (3*3^(1/2)*dq1*dqr3*cos(2*q5)*sin(2*q2)*sin(2*q3)*sin(q4))/64 + (3*3^(1/2)*dq1*dqr3*sin(2*q2)*sin(2*q3)*sin(2*q5)*cos(q4))/32 + (9*3^(1/2)*dq1*dqr3*cos(2*q6)*sin(2*q2)*sin(2*q3)*sin(q4))/64 - (25*dq1*dqr3*cos(2*q3)*cos(2*q4)*cos(2*q5)*cos(2*q6)*sin(2*q2))/256 - (3*dq2*dqr3*sin(2*q4)*sin(2*q6)*cos(q2)*cos(q3)*sin(q5))/16 + (3*dq3*dqr3*sin(2*q4)*sin(2*q6)*cos(q2)*cos(q3)*sin(q5))/16 - (3*3^(1/2)*dq5*dqr3*sin(2*q5)*cos(q2)*cos(q3)*cos(q4))/64 - (9*3^(1/2)*dq6*dqr3*sin(2*q6)*cos(q2)*cos(q3)*cos(q4))/64 - (5*dq1*dqr3*cos(2*q2)*cos(2*q6)*sin(2*q3)*sin(2*q4)*sin(2*q5))/64 + (5*dq1*dqr3*cos(2*q3)*cos(2*q4)*sin(2*q2)*sin(2*q5)*sin(2*q6))/64 + (dq1*dqr3*cos(2*q3)*cos(2*q5)*sin(2*q2)*sin(2*q4)*sin(2*q6))/16 + (5*dq1*dqr3*cos(2*q3)*cos(2*q6)*sin(2*q2)*sin(2*q4)*sin(2*q5))/64 + (dq2*dqr3*cos(2*q4)*cos(2*q5)*sin(2*q6)*cos(q2)*cos(q3))/8 + (5*dq2*dqr3*cos(2*q4)*cos(2*q6)*sin(2*q5)*cos(q2)*cos(q3))/32 + (25*dq2*dqr3*cos(2*q5)*cos(2*q6)*sin(2*q4)*cos(q2)*cos(q3))/128 - (dq3*dqr3*cos(2*q4)*cos(2*q5)*sin(2*q6)*cos(q2)*cos(q3))/8 - (5*dq3*dqr3*cos(2*q4)*cos(2*q6)*sin(2*q5)*cos(q2)*cos(q3))/32 - (25*dq3*dqr3*cos(2*q5)*cos(2*q6)*sin(2*q4)*cos(q2)*cos(q3))/128 - (5*dq2*dqr3*sin(2*q4)*sin(2*q5)*sin(2*q6)*cos(q2)*cos(q3))/32 + (5*dq3*dqr3*sin(2*q4)*sin(2*q5)*sin(2*q6)*cos(q2)*cos(q3))/32 + (3^(1/2)*dq1*dqr3*cos(2*q2)*cos(2*q3)*cos(q4)*sin(q5))/16 - (3^(1/2)*dq1*dqr3*cos(2*q2)*cos(2*q3)*cos(q5)*sin(q4))/16 + (3^(1/2)*dq1*dqr3*sin(2*q2)*sin(2*q3)*cos(q4)*sin(q5))/16 - (3^(1/2)*dq1*dqr3*sin(2*q2)*sin(2*q3)*cos(q5)*sin(q4))/16 + (3*dq1*dqr3*cos(2*q2)*cos(2*q4)*cos(2*q6)*sin(2*q3)*cos(q5))/64 - (3*dq1*dqr3*cos(2*q3)*cos(2*q4)*cos(2*q6)*sin(2*q2)*cos(q5))/64 + (3*3^(1/2)*dq5*dqr3*cos(q2)*cos(q3)*cos(q4)*sin(q5))/32 + (3^(1/2)*dq6*dqr3*cos(q2)*cos(q3)*cos(q4)*sin(q5))/4 - (3*dq1*dqr3*cos(2*q2)*cos(2*q4)*sin(2*q3)*sin(2*q6)*sin(q5))/32 - (3*dq1*dqr3*cos(2*q2)*cos(2*q6)*sin(2*q3)*sin(2*q4)*sin(q5))/32 - (3*dq1*dqr3*cos(2*q2)*sin(2*q3)*sin(2*q4)*sin(2*q6)*cos(q5))/16 + (3*dq1*dqr3*cos(2*q3)*cos(2*q4)*sin(2*q2)*sin(2*q6)*sin(q5))/32 + (3*dq1*dqr3*cos(2*q3)*cos(2*q6)*sin(2*q2)*sin(2*q4)*sin(q5))/32 + (3*dq1*dqr3*cos(2*q3)*sin(2*q2)*sin(2*q4)*sin(2*q6)*cos(q5))/16 + (3*3^(1/2)*dq5*dqr3*cos(2*q6)*cos(q2)*cos(q3)*cos(q4)*sin(q5))/32 + (3*3^(1/2)*dq5*dqr3*sin(2*q6)*cos(q2)*cos(q3)*cos(q4)*cos(q5))/16 + (3^(1/2)*dq6*dqr3*cos(2*q6)*cos(q2)*cos(q3)*cos(q4)*sin(q5))/8 + (3^(1/2)*dq6*dqr3*sin(2*q6)*cos(q2)*cos(q3)*cos(q4)*cos(q5))/16 - (5*3^(1/2)*dq1*dqr3*cos(2*q2)*cos(2*q3)*cos(2*q5)*cos(2*q6)*sin(q4))/64 - (3^(1/2)*dq1*dqr3*cos(2*q2)*cos(2*q3)*cos(2*q5)*sin(2*q6)*cos(q4))/8 - (5*3^(1/2)*dq1*dqr3*cos(2*q2)*cos(2*q3)*cos(2*q6)*sin(2*q5)*cos(q4))/32 + (3^(1/2)*dq1*dqr3*cos(2*q2)*cos(2*q3)*sin(2*q5)*sin(2*q6)*sin(q4))/16 - (5*3^(1/2)*dq1*dqr3*cos(2*q5)*cos(2*q6)*sin(2*q2)*sin(2*q3)*sin(q4))/64 - (3^(1/2)*dq1*dqr3*cos(2*q5)*sin(2*q2)*sin(2*q3)*sin(2*q6)*cos(q4))/8 - (5*3^(1/2)*dq1*dqr3*cos(2*q6)*sin(2*q2)*sin(2*q3)*sin(2*q5)*cos(q4))/32 + (3^(1/2)*dq1*dqr3*sin(2*q2)*sin(2*q3)*sin(2*q5)*sin(2*q6)*sin(q4))/16 + (3^(1/2)*dq5*dqr3*cos(2*q5)*sin(2*q6)*cos(q2)*cos(q3)*cos(q4))/16 + (5*3^(1/2)*dq5*dqr3*cos(2*q6)*sin(2*q5)*cos(q2)*cos(q3)*cos(q4))/64 + (3^(1/2)*dq6*dqr3*cos(2*q5)*cos(2*q6)*cos(q2)*cos(q3)*sin(q4))/8 + (5*3^(1/2)*dq6*dqr3*cos(2*q5)*sin(2*q6)*cos(q2)*cos(q3)*cos(q4))/64 + (3^(1/2)*dq6*dqr3*cos(2*q6)*sin(2*q5)*cos(q2)*cos(q3)*cos(q4))/16 + (3^(1/2)*dq1*dqr3*cos(2*q2)*cos(2*q3)*cos(2*q6)*cos(q4)*sin(q5))/16 - (3^(1/2)*dq1*dqr3*cos(2*q2)*cos(2*q3)*cos(2*q6)*cos(q5)*sin(q4))/16 + (3^(1/2)*dq1*dqr3*cos(2*q2)*cos(2*q3)*sin(2*q6)*cos(q4)*cos(q5))/8 + (3^(1/2)*dq1*dqr3*cos(2*q6)*sin(2*q2)*sin(2*q3)*cos(q4)*sin(q5))/16 - (3^(1/2)*dq1*dqr3*cos(2*q6)*sin(2*q2)*sin(2*q3)*cos(q5)*sin(q4))/16 + (3^(1/2)*dq1*dqr3*sin(2*q2)*sin(2*q3)*sin(2*q6)*cos(q4)*cos(q5))/8;
Y1_20_11=(3*dq3*dqr4*cos(q3)*cos(q5)*sin(q2))/32 - (43*dq2*dqr4*cos(q3)*sin(q2))/128 - (3*dq2*dqr4*cos(2*q4)*cos(q3)*sin(q2))/128 - (9*dq2*dqr4*cos(2*q5)*cos(q3)*sin(q2))/128 - (3*dq2*dqr4*cos(2*q6)*cos(q3)*sin(q2))/128 - (9*dq5*dqr4*sin(2*q5)*sin(q2)*sin(q3))/64 - (3*dq6*dqr4*sin(2*q6)*sin(q2)*sin(q3))/64 - (3*dq2*dqr4*cos(q3)*cos(q5)*sin(q2))/32 - (dq1*dqr3*cos(2*q2)*sin(2*q3))/256 + (3*dq1*dqr3*cos(2*q2)*cos(2*q4)*sin(2*q3))/256 - (27*dq1*dqr3*cos(2*q2)*cos(2*q5)*sin(2*q3))/256 - (9*dq1*dqr3*cos(2*q2)*cos(2*q6)*sin(2*q3))/256 - (3*dq5*dqr4*sin(q2)*sin(q3)*sin(q5))/32 - (15*dq1*dqr3*cos(2*q2)*cos(2*q4)*cos(2*q5)*sin(2*q3))/256 + (27*dq1*dqr3*cos(2*q2)*cos(2*q4)*cos(2*q6)*sin(2*q3))/256 + (45*dq1*dqr3*cos(2*q2)*cos(2*q5)*cos(2*q6)*sin(2*q3))/256 + (3*dq2*dqr4*sin(2*q4)*cos(q3)*sin(q2)*sin(q5))/16 - (3*dq3*dqr4*sin(2*q4)*cos(q3)*sin(q2)*sin(q5))/16 + (3*dq2*dqr4*sin(2*q6)*cos(q3)*sin(q2)*sin(q5))/16 - (3*dq3*dqr4*sin(2*q6)*cos(q3)*sin(q2)*sin(q5))/16 - (3*dq5*dqr4*cos(2*q6)*sin(q2)*sin(q3)*sin(q5))/32 - (3*dq5*dqr4*sin(2*q6)*cos(q5)*sin(q2)*sin(q3))/16 - (3*dq6*dqr4*cos(2*q6)*sin(q2)*sin(q3)*sin(q5))/8 - (3*dq6*dqr4*sin(2*q6)*cos(q5)*sin(q2)*sin(q3))/16 - (3^(1/2)*dq4*dqr4*cos(q3)*cos(q4)*sin(q2))/64 + (5*3^(1/2)*dq5*dqr4*cos(q3)*cos(q4)*sin(q2))/32 + (3^(1/2)*dq6*dqr4*cos(q3)*cos(q4)*sin(q2))/8 + (3*dq1*dqr3*cos(2*q2)*sin(2*q3)*sin(2*q4)*sin(2*q5))/64 - (9*dq1*dqr3*cos(2*q2)*sin(2*q3)*sin(2*q5)*sin(2*q6))/64 + (15*dq2*dqr4*cos(2*q4)*cos(2*q5)*cos(q3)*sin(q2))/128 - (27*dq2*dqr4*cos(2*q4)*cos(2*q6)*cos(q3)*sin(q2))/128 + (15*dq2*dqr4*cos(2*q5)*cos(2*q6)*cos(q3)*sin(q2))/128 - (3*dq2*dqr4*sin(2*q4)*sin(2*q5)*cos(q3)*sin(q2))/32 + (3*dq3*dqr4*sin(2*q4)*sin(2*q5)*cos(q3)*sin(q2))/32 - (3*dq2*dqr4*sin(2*q5)*sin(2*q6)*cos(q3)*sin(q2))/32 + (3*dq3*dqr4*sin(2*q5)*sin(2*q6)*cos(q3)*sin(q2))/32 + (3*dq5*dqr4*cos(2*q5)*sin(2*q6)*sin(q2)*sin(q3))/16 + (15*dq5*dqr4*cos(2*q6)*sin(2*q5)*sin(q2)*sin(q3))/64 + (15*dq6*dqr4*cos(2*q5)*sin(2*q6)*sin(q2)*sin(q3))/64 + (3*dq6*dqr4*cos(2*q6)*sin(2*q5)*sin(q2)*sin(q3))/16 - (3*dq2*dqr4*cos(2*q4)*cos(q3)*cos(q5)*sin(q2))/32 + (3*dq3*dqr4*cos(2*q4)*cos(q3)*cos(q5)*sin(q2))/32 - (3*dq2*dqr4*cos(2*q6)*cos(q3)*cos(q5)*sin(q2))/32 + (3*dq3*dqr4*cos(2*q6)*cos(q3)*cos(q5)*sin(q2))/32 + (3^(1/2)*dq4*dqr4*cos(q3)*sin(q2)*sin(q4)*sin(q5))/16 + (3^(1/2)*dq5*dqr4*cos(q3)*sin(q2)*sin(q4)*sin(q5))/32 + (3^(1/2)*dq6*dqr4*cos(q3)*sin(q2)*sin(q4)*sin(q5))/4 - (3*dq2*dqr4*cos(2*q4)*cos(2*q6)*cos(q3)*cos(q5)*sin(q2))/32 + (3*dq3*dqr4*cos(2*q4)*cos(2*q6)*cos(q3)*cos(q5)*sin(q2))/32 + (25*dq1*dqr3*cos(2*q2)*cos(2*q4)*cos(2*q5)*cos(2*q6)*sin(2*q3))/256 + (3*dq2*dqr4*cos(2*q4)*sin(2*q6)*cos(q3)*sin(q2)*sin(q5))/16 + (3*dq2*dqr4*cos(2*q6)*sin(2*q4)*cos(q3)*sin(q2)*sin(q5))/16 + (3*dq2*dqr4*sin(2*q4)*sin(2*q6)*cos(q3)*cos(q5)*sin(q2))/8 - (3*dq3*dqr4*cos(2*q4)*sin(2*q6)*cos(q3)*sin(q2)*sin(q5))/16 - (3*dq3*dqr4*cos(2*q6)*sin(2*q4)*cos(q3)*sin(q2)*sin(q5))/16 - (3*dq3*dqr4*sin(2*q4)*sin(2*q6)*cos(q3)*cos(q5)*sin(q2))/8 - (3*3^(1/2)*dq4*dqr4*cos(2*q5)*cos(q3)*cos(q4)*sin(q2))/64 - (9*3^(1/2)*dq4*dqr4*cos(2*q6)*cos(q3)*cos(q4)*sin(q2))/64 - (3*3^(1/2)*dq5*dqr4*cos(2*q5)*cos(q3)*cos(q4)*sin(q2))/32 - (3*3^(1/2)*dq5*dqr4*cos(2*q6)*cos(q3)*cos(q4)*sin(q2))/32 - (5*dq1*dqr3*cos(2*q2)*cos(2*q4)*sin(2*q3)*sin(2*q5)*sin(2*q6))/64 - (dq1*dqr3*cos(2*q2)*cos(2*q5)*sin(2*q3)*sin(2*q4)*sin(2*q6))/16 + (3*3^(1/2)*dq4*dqr4*sin(2*q5)*cos(q3)*sin(q2)*sin(q4))/32 + (3*3^(1/2)*dq5*dqr4*sin(2*q5)*cos(q3)*sin(q2)*sin(q4))/64 + (9*3^(1/2)*dq6*dqr4*sin(2*q6)*cos(q3)*sin(q2)*sin(q4))/64 - (25*dq2*dqr4*cos(2*q4)*cos(2*q5)*cos(2*q6)*cos(q3)*sin(q2))/128 + (25*dq3*dqr4*cos(2*q4)*cos(2*q5)*cos(2*q6)*cos(q3)*sin(q2))/128 + (5*dq2*dqr4*cos(2*q4)*sin(2*q5)*sin(2*q6)*cos(q3)*sin(q2))/32 + (dq2*dqr4*cos(2*q5)*sin(2*q4)*sin(2*q6)*cos(q3)*sin(q2))/8 + (5*dq2*dqr4*cos(2*q6)*sin(2*q4)*sin(2*q5)*cos(q3)*sin(q2))/32 - (5*dq3*dqr4*cos(2*q4)*sin(2*q5)*sin(2*q6)*cos(q3)*sin(q2))/32 - (dq3*dqr4*cos(2*q5)*sin(2*q4)*sin(2*q6)*cos(q3)*sin(q2))/8 - (5*dq3*dqr4*cos(2*q6)*sin(2*q4)*sin(2*q5)*cos(q3)*sin(q2))/32 + (3^(1/2)*dq4*dqr4*cos(q3)*cos(q4)*cos(q5)*sin(q2))/16 - (3^(1/2)*dq5*dqr4*cos(q3)*cos(q4)*cos(q5)*sin(q2))/16 - (3^(1/2)*dq6*dqr4*cos(q3)*cos(q4)*cos(q5)*sin(q2))/8 + (3^(1/2)*dq4*dqr4*cos(2*q6)*cos(q3)*cos(q4)*cos(q5)*sin(q2))/16 - (3^(1/2)*dq5*dqr4*cos(2*q6)*cos(q3)*cos(q4)*cos(q5)*sin(q2))/16 - (3^(1/2)*dq6*dqr4*cos(2*q6)*cos(q3)*cos(q4)*cos(q5)*sin(q2))/8 + (3^(1/2)*dq4*dqr4*cos(2*q6)*cos(q3)*sin(q2)*sin(q4)*sin(q5))/16 - (3^(1/2)*dq4*dqr4*sin(2*q6)*cos(q3)*cos(q4)*sin(q2)*sin(q5))/8 + (3^(1/2)*dq4*dqr4*sin(2*q6)*cos(q3)*cos(q5)*sin(q2)*sin(q4))/8 + (3^(1/2)*dq5*dqr4*cos(2*q6)*cos(q3)*sin(q2)*sin(q4)*sin(q5))/32 + (3^(1/2)*dq5*dqr4*sin(2*q6)*cos(q3)*cos(q4)*sin(q2)*sin(q5))/8 + (3^(1/2)*dq5*dqr4*sin(2*q6)*cos(q3)*cos(q5)*sin(q2)*sin(q4))/16 - (3^(1/2)*dq6*dqr4*cos(2*q6)*cos(q3)*sin(q2)*sin(q4)*sin(q5))/8 + (3^(1/2)*dq6*dqr4*sin(2*q6)*cos(q3)*cos(q4)*sin(q2)*sin(q5))/16 - (3^(1/2)*dq6*dqr4*sin(2*q6)*cos(q3)*cos(q5)*sin(q2)*sin(q4))/16 + (5*3^(1/2)*dq4*dqr4*cos(2*q5)*cos(2*q6)*cos(q3)*cos(q4)*sin(q2))/64 + (5*3^(1/2)*dq5*dqr4*cos(2*q5)*cos(2*q6)*cos(q3)*cos(q4)*sin(q2))/32 + (3^(1/2)*dq6*dqr4*cos(2*q5)*cos(2*q6)*cos(q3)*cos(q4)*sin(q2))/8 - (3^(1/2)*dq4*dqr4*cos(2*q5)*sin(2*q6)*cos(q3)*sin(q2)*sin(q4))/8 - (5*3^(1/2)*dq4*dqr4*cos(2*q6)*sin(2*q5)*cos(q3)*sin(q2)*sin(q4))/32 - (3^(1/2)*dq4*dqr4*sin(2*q5)*sin(2*q6)*cos(q3)*cos(q4)*sin(q2))/16 - (3^(1/2)*dq5*dqr4*cos(2*q5)*sin(2*q6)*cos(q3)*sin(q2)*sin(q4))/16 - (5*3^(1/2)*dq5*dqr4*cos(2*q6)*sin(2*q5)*cos(q3)*sin(q2)*sin(q4))/64 - (3^(1/2)*dq5*dqr4*sin(2*q5)*sin(2*q6)*cos(q3)*cos(q4)*sin(q2))/8 - (5*3^(1/2)*dq6*dqr4*cos(2*q5)*sin(2*q6)*cos(q3)*sin(q2)*sin(q4))/64 - (3^(1/2)*dq6*dqr4*cos(2*q6)*sin(2*q5)*cos(q3)*sin(q2)*sin(q4))/16 - (5*3^(1/2)*dq6*dqr4*sin(2*q5)*sin(2*q6)*cos(q3)*cos(q4)*sin(q2))/32;
Y1_20_12=(43*dq2*dqr4*cos(q2)*sin(q3))/128 - (43*dq3*dqr4*cos(q2)*sin(q3))/128 + (43*dq3*dqr4*cos(q3)*sin(q2))/128 + (3*dq2*dqr4*cos(2*q4)*cos(q2)*sin(q3))/128 + (9*dq2*dqr4*cos(2*q5)*cos(q2)*sin(q3))/128 - (3*dq3*dqr4*cos(2*q4)*cos(q2)*sin(q3))/128 + (3*dq3*dqr4*cos(2*q4)*cos(q3)*sin(q2))/128 + (3*dq2*dqr4*cos(2*q6)*cos(q2)*sin(q3))/128 - (9*dq3*dqr4*cos(2*q5)*cos(q2)*sin(q3))/128 + (9*dq3*dqr4*cos(2*q5)*cos(q3)*sin(q2))/128 - (3*dq3*dqr4*cos(2*q6)*cos(q2)*sin(q3))/128 + (3*dq3*dqr4*cos(2*q6)*cos(q3)*sin(q2))/128 + (3*dq2*dqr4*cos(q2)*cos(q5)*sin(q3))/32 - (3*dq3*dqr4*cos(q2)*cos(q5)*sin(q3))/32 - (3*dq2*dqr4*sin(2*q4)*cos(q2)*sin(q3)*sin(q5))/16 + (3*dq3*dqr4*sin(2*q4)*cos(q2)*sin(q3)*sin(q5))/16 - (3*dq2*dqr4*sin(2*q6)*cos(q2)*sin(q3)*sin(q5))/16 + (3*dq3*dqr4*sin(2*q6)*cos(q2)*sin(q3)*sin(q5))/16 + (3^(1/2)*dq4*dqr4*cos(q2)*cos(q4)*sin(q3))/64 - (5*3^(1/2)*dq5*dqr4*cos(q2)*cos(q4)*sin(q3))/32 - (3^(1/2)*dq6*dqr4*cos(q2)*cos(q4)*sin(q3))/8 - (15*dq2*dqr4*cos(2*q4)*cos(2*q5)*cos(q2)*sin(q3))/128 + (27*dq2*dqr4*cos(2*q4)*cos(2*q6)*cos(q2)*sin(q3))/128 + (15*dq3*dqr4*cos(2*q4)*cos(2*q5)*cos(q2)*sin(q3))/128 - (15*dq3*dqr4*cos(2*q4)*cos(2*q5)*cos(q3)*sin(q2))/128 - (15*dq2*dqr4*cos(2*q5)*cos(2*q6)*cos(q2)*sin(q3))/128 - (27*dq3*dqr4*cos(2*q4)*cos(2*q6)*cos(q2)*sin(q3))/128 + (27*dq3*dqr4*cos(2*q4)*cos(2*q6)*cos(q3)*sin(q2))/128 + (15*dq3*dqr4*cos(2*q5)*cos(2*q6)*cos(q2)*sin(q3))/128 - (15*dq3*dqr4*cos(2*q5)*cos(2*q6)*cos(q3)*sin(q2))/128 + (3*dq2*dqr4*sin(2*q4)*sin(2*q5)*cos(q2)*sin(q3))/32 - (3*dq3*dqr4*sin(2*q4)*sin(2*q5)*cos(q2)*sin(q3))/32 + (3*dq2*dqr4*sin(2*q5)*sin(2*q6)*cos(q2)*sin(q3))/32 - (3*dq3*dqr4*sin(2*q5)*sin(2*q6)*cos(q2)*sin(q3))/32 + (3*dq2*dqr4*cos(2*q4)*cos(q2)*cos(q5)*sin(q3))/32 - (3*dq3*dqr4*cos(2*q4)*cos(q2)*cos(q5)*sin(q3))/32 + (3*dq2*dqr4*cos(2*q6)*cos(q2)*cos(q5)*sin(q3))/32 - (3*dq3*dqr4*cos(2*q6)*cos(q2)*cos(q5)*sin(q3))/32 - (3^(1/2)*dq4*dqr4*cos(q2)*sin(q3)*sin(q4)*sin(q5))/16 - (3^(1/2)*dq5*dqr4*cos(q2)*sin(q3)*sin(q4)*sin(q5))/32 - (3^(1/2)*dq6*dqr4*cos(q2)*sin(q3)*sin(q4)*sin(q5))/4 + (3*dq2*dqr4*cos(2*q4)*cos(2*q6)*cos(q2)*cos(q5)*sin(q3))/32 - (3*dq3*dqr4*cos(2*q4)*cos(2*q6)*cos(q2)*cos(q5)*sin(q3))/32 + (3*3^(1/2)*dq1*dqr4*cos(2*q3)*sin(2*q2)*sin(2*q5)*sin(q4))/64 - (3*dq2*dqr4*cos(2*q4)*sin(2*q6)*cos(q2)*sin(q3)*sin(q5))/16 - (3*dq2*dqr4*cos(2*q6)*sin(2*q4)*cos(q2)*sin(q3)*sin(q5))/16 - (3*dq2*dqr4*sin(2*q4)*sin(2*q6)*cos(q2)*cos(q5)*sin(q3))/8 + (3*dq3*dqr4*cos(2*q4)*sin(2*q6)*cos(q2)*sin(q3)*sin(q5))/16 + (3*dq3*dqr4*cos(2*q6)*sin(2*q4)*cos(q2)*sin(q3)*sin(q5))/16 + (3*dq3*dqr4*sin(2*q4)*sin(2*q6)*cos(q2)*cos(q5)*sin(q3))/8 + (3*3^(1/2)*dq4*dqr4*cos(2*q5)*cos(q2)*cos(q4)*sin(q3))/64 + (9*3^(1/2)*dq4*dqr4*cos(2*q6)*cos(q2)*cos(q4)*sin(q3))/64 + (3*3^(1/2)*dq5*dqr4*cos(2*q5)*cos(q2)*cos(q4)*sin(q3))/32 + (3*3^(1/2)*dq5*dqr4*cos(2*q6)*cos(q2)*cos(q4)*sin(q3))/32 - (3*3^(1/2)*dq4*dqr4*sin(2*q5)*cos(q2)*sin(q3)*sin(q4))/32 - (3*3^(1/2)*dq5*dqr4*sin(2*q5)*cos(q2)*sin(q3)*sin(q4))/64 - (9*3^(1/2)*dq6*dqr4*sin(2*q6)*cos(q2)*sin(q3)*sin(q4))/64 + (25*dq2*dqr4*cos(2*q4)*cos(2*q5)*cos(2*q6)*cos(q2)*sin(q3))/128 - (25*dq3*dqr4*cos(2*q4)*cos(2*q5)*cos(2*q6)*cos(q2)*sin(q3))/128 - (5*dq2*dqr4*cos(2*q4)*sin(2*q5)*sin(2*q6)*cos(q2)*sin(q3))/32 - (dq2*dqr4*cos(2*q5)*sin(2*q4)*sin(2*q6)*cos(q2)*sin(q3))/8 - (5*dq2*dqr4*cos(2*q6)*sin(2*q4)*sin(2*q5)*cos(q2)*sin(q3))/32 + (5*dq3*dqr4*cos(2*q4)*sin(2*q5)*sin(2*q6)*cos(q2)*sin(q3))/32 + (dq3*dqr4*cos(2*q5)*sin(2*q4)*sin(2*q6)*cos(q2)*sin(q3))/8 + (5*dq3*dqr4*cos(2*q6)*sin(2*q4)*sin(2*q5)*cos(q2)*sin(q3))/32 - (3^(1/2)*dq1*dqr4*cos(2*q2)*sin(2*q3)*sin(q4)*sin(q5))/32 + (3^(1/2)*dq1*dqr4*cos(2*q3)*sin(2*q2)*sin(q4)*sin(q5))/32 - (3^(1/2)*dq4*dqr4*cos(q2)*cos(q4)*cos(q5)*sin(q3))/16 + (3^(1/2)*dq5*dqr4*cos(q2)*cos(q4)*cos(q5)*sin(q3))/16 + (3^(1/2)*dq6*dqr4*cos(q2)*cos(q4)*cos(q5)*sin(q3))/8 - (3^(1/2)*dq4*dqr4*cos(2*q6)*cos(q2)*cos(q4)*cos(q5)*sin(q3))/16 + (3^(1/2)*dq5*dqr4*cos(2*q6)*cos(q2)*cos(q4)*cos(q5)*sin(q3))/16 + (3^(1/2)*dq6*dqr4*cos(2*q6)*cos(q2)*cos(q4)*cos(q5)*sin(q3))/8 - (3^(1/2)*dq4*dqr4*cos(2*q6)*cos(q2)*sin(q3)*sin(q4)*sin(q5))/16 + (3^(1/2)*dq4*dqr4*sin(2*q6)*cos(q2)*cos(q4)*sin(q3)*sin(q5))/8 - (3^(1/2)*dq4*dqr4*sin(2*q6)*cos(q2)*cos(q5)*sin(q3)*sin(q4))/8 - (3^(1/2)*dq5*dqr4*cos(2*q6)*cos(q2)*sin(q3)*sin(q4)*sin(q5))/32 - (3^(1/2)*dq5*dqr4*sin(2*q6)*cos(q2)*cos(q4)*sin(q3)*sin(q5))/8 - (3^(1/2)*dq5*dqr4*sin(2*q6)*cos(q2)*cos(q5)*sin(q3)*sin(q4))/16 + (3^(1/2)*dq6*dqr4*cos(2*q6)*cos(q2)*sin(q3)*sin(q4)*sin(q5))/8 - (3^(1/2)*dq6*dqr4*sin(2*q6)*cos(q2)*cos(q4)*sin(q3)*sin(q5))/16 + (3^(1/2)*dq6*dqr4*sin(2*q6)*cos(q2)*cos(q5)*sin(q3)*sin(q4))/16 - (3^(1/2)*dq1*dqr4*cos(2*q3)*cos(2*q5)*sin(2*q2)*sin(2*q6)*sin(q4))/16 - (5*3^(1/2)*dq1*dqr4*cos(2*q3)*cos(2*q6)*sin(2*q2)*sin(2*q5)*sin(q4))/64 - (5*3^(1/2)*dq4*dqr4*cos(2*q5)*cos(2*q6)*cos(q2)*cos(q4)*sin(q3))/64 - (5*3^(1/2)*dq5*dqr4*cos(2*q5)*cos(2*q6)*cos(q2)*cos(q4)*sin(q3))/32 - (3^(1/2)*dq6*dqr4*cos(2*q5)*cos(2*q6)*cos(q2)*cos(q4)*sin(q3))/8 + (3^(1/2)*dq4*dqr4*cos(2*q5)*sin(2*q6)*cos(q2)*sin(q3)*sin(q4))/8 + (5*3^(1/2)*dq4*dqr4*cos(2*q6)*sin(2*q5)*cos(q2)*sin(q3)*sin(q4))/32 + (3^(1/2)*dq4*dqr4*sin(2*q5)*sin(2*q6)*cos(q2)*cos(q4)*sin(q3))/16 + (3^(1/2)*dq5*dqr4*cos(2*q5)*sin(2*q6)*cos(q2)*sin(q3)*sin(q4))/16 + (5*3^(1/2)*dq5*dqr4*cos(2*q6)*sin(2*q5)*cos(q2)*sin(q3)*sin(q4))/64 + (3^(1/2)*dq5*dqr4*sin(2*q5)*sin(2*q6)*cos(q2)*cos(q4)*sin(q3))/8 + (5*3^(1/2)*dq6*dqr4*cos(2*q5)*sin(2*q6)*cos(q2)*sin(q3)*sin(q4))/64 + (3^(1/2)*dq6*dqr4*cos(2*q6)*sin(2*q5)*cos(q2)*sin(q3)*sin(q4))/16 + (5*3^(1/2)*dq6*dqr4*sin(2*q5)*sin(2*q6)*cos(q2)*cos(q4)*sin(q3))/32 - (3^(1/2)*dq1*dqr4*cos(2*q2)*cos(2*q6)*sin(2*q3)*sin(q4)*sin(q5))/32 - (3^(1/2)*dq1*dqr4*cos(2*q2)*sin(2*q3)*sin(2*q6)*cos(q5)*sin(q4))/16 + (3^(1/2)*dq1*dqr4*cos(2*q3)*cos(2*q6)*sin(2*q2)*sin(q4)*sin(q5))/32 + (3^(1/2)*dq1*dqr4*cos(2*q3)*sin(2*q2)*sin(2*q6)*cos(q5)*sin(q4))/16;
Y1_20_13=(3*dq1*dqr4*cos(2*q4)*sin(2*q5))/64 - (3*dq1*dqr4*cos(2*q4)*sin(q5))/32 - (3*dq1*dqr4*sin(2*q4)*cos(q5))/64 - (3*dq1*dqr4*sin(2*q4))/256 + (15*dq1*dqr4*cos(2*q5)*sin(2*q4))/256 - (27*dq1*dqr4*cos(2*q6)*sin(2*q4))/256 - (9*dq5*dqr4*sin(2*q5)*cos(q2)*cos(q3))/64 - (3*dq6*dqr4*sin(2*q6)*cos(q2)*cos(q3))/64 - (3*dq1*dqr4*cos(2*q4)*cos(2*q6)*sin(q5))/32 - (3*dq1*dqr4*cos(2*q4)*sin(2*q6)*cos(q5))/16 - (3*dq1*dqr4*cos(2*q6)*sin(2*q4)*cos(q5))/64 + (3*dq1*dqr4*sin(2*q4)*sin(2*q6)*sin(q5))/32 - (3*dq5*dqr4*cos(q2)*cos(q3)*sin(q5))/32 + (3*dq1*dqr4*cos(2*q2)*cos(2*q3)*sin(2*q4))/256 - (dq1*dqr4*cos(2*q4)*cos(2*q5)*sin(2*q6))/16 - (5*dq1*dqr4*cos(2*q4)*cos(2*q6)*sin(2*q5))/64 - (25*dq1*dqr4*cos(2*q5)*cos(2*q6)*sin(2*q4))/256 - (3*dq4*dqr5*sin(q2)*sin(q3)*sin(q5))/32 - (3*dq5*dqr5*sin(q2)*sin(q3)*sin(q5))/16 - (3*dq6*dqr5*sin(q2)*sin(q3)*sin(q5))/8 + (3*dq1*dqr4*sin(2*q2)*sin(2*q3)*sin(2*q4))/256 + (5*dq1*dqr4*sin(2*q4)*sin(2*q5)*sin(2*q6))/64 - (3*dq1*dqr4*cos(2*q2)*cos(2*q3)*cos(2*q4)*sin(2*q5))/64 - (15*dq1*dqr4*cos(2*q2)*cos(2*q3)*cos(2*q5)*sin(2*q4))/256 + (27*dq1*dqr4*cos(2*q2)*cos(2*q3)*cos(2*q6)*sin(2*q4))/256 - (3*dq4*dqr5*cos(2*q6)*sin(q2)*sin(q3)*sin(q5))/32 - (3*dq5*dqr5*cos(2*q6)*sin(q2)*sin(q3)*sin(q5))/16 - (3*dq6*dqr5*cos(2*q6)*sin(q2)*sin(q3)*sin(q5))/8 - (3*dq1*dqr4*cos(2*q4)*sin(2*q2)*sin(2*q3)*sin(2*q5))/64 - (15*dq1*dqr4*cos(2*q5)*sin(2*q2)*sin(2*q3)*sin(2*q4))/256 + (27*dq1*dqr4*cos(2*q6)*sin(2*q2)*sin(2*q3)*sin(2*q4))/256 + (5*3^(1/2)*dq2*dqr5*sin(q2)*sin(q3)*sin(q4))/32 - (5*3^(1/2)*dq3*dqr5*sin(q2)*sin(q3)*sin(q4))/32 + (3*dq5*dqr4*cos(2*q5)*sin(2*q6)*cos(q2)*cos(q3))/16 + (15*dq5*dqr4*cos(2*q6)*sin(2*q5)*cos(q2)*cos(q3))/64 + (15*dq6*dqr4*cos(2*q5)*sin(2*q6)*cos(q2)*cos(q3))/64 + (3*dq6*dqr4*cos(2*q6)*sin(2*q5)*cos(q2)*cos(q3))/16 + (3*dq1*dqr4*cos(2*q2)*cos(2*q3)*cos(2*q4)*sin(q5))/32 + (3*dq1*dqr4*cos(2*q2)*cos(2*q3)*sin(2*q4)*cos(q5))/64 + (3*dq1*dqr4*cos(2*q4)*sin(2*q2)*sin(2*q3)*sin(q5))/32 + (3*dq1*dqr4*sin(2*q2)*sin(2*q3)*sin(2*q4)*cos(q5))/64 + (3^(1/2)*dq1*dqr4*cos(2*q2)*sin(2*q3)*cos(q4))/128 - (3^(1/2)*dq1*dqr4*cos(2*q3)*sin(2*q2)*cos(q4))/128 - (3*dq5*dqr4*cos(2*q6)*cos(q2)*cos(q3)*sin(q5))/32 - (3*dq5*dqr4*sin(2*q6)*cos(q2)*cos(q3)*cos(q5))/16 - (3*dq6*dqr4*cos(2*q6)*cos(q2)*cos(q3)*sin(q5))/8 - (3*dq6*dqr4*sin(2*q6)*cos(q2)*cos(q3)*cos(q5))/16 + (3*3^(1/2)*dq1*dqr4*cos(2*q2)*cos(2*q5)*sin(2*q3)*cos(q4))/128 - (3*3^(1/2)*dq1*dqr4*cos(2*q3)*cos(2*q5)*sin(2*q2)*cos(q4))/128 + (9*3^(1/2)*dq1*dqr4*cos(2*q2)*cos(2*q6)*sin(2*q3)*cos(q4))/128 - (9*3^(1/2)*dq1*dqr4*cos(2*q3)*cos(2*q6)*sin(2*q2)*cos(q4))/128 - (3*3^(1/2)*dq2*dqr5*cos(q4)*sin(q2)*sin(q3)*sin(q5))/32 + (3*3^(1/2)*dq3*dqr5*cos(q4)*sin(q2)*sin(q3)*sin(q5))/32 - (3*dq1*dqr4*sin(2*q2)*sin(2*q3)*sin(2*q4)*sin(2*q6)*sin(q5))/32 - (3*3^(1/2)*dq1*dqr4*cos(2*q2)*sin(2*q3)*sin(2*q5)*sin(q4))/64 + (dq1*dqr4*cos(2*q2)*cos(2*q3)*cos(2*q4)*cos(2*q5)*sin(2*q6))/16 + (5*dq1*dqr4*cos(2*q2)*cos(2*q3)*cos(2*q4)*cos(2*q6)*sin(2*q5))/64 + (25*dq1*dqr4*cos(2*q2)*cos(2*q3)*cos(2*q5)*cos(2*q6)*sin(2*q4))/256 - (5*dq1*dqr4*cos(2*q2)*cos(2*q3)*sin(2*q4)*sin(2*q5)*sin(2*q6))/64 + (dq1*dqr4*cos(2*q4)*cos(2*q5)*sin(2*q2)*sin(2*q3)*sin(2*q6))/16 + (5*dq1*dqr4*cos(2*q4)*cos(2*q6)*sin(2*q2)*sin(2*q3)*sin(2*q5))/64 + (25*dq1*dqr4*cos(2*q5)*cos(2*q6)*sin(2*q2)*sin(2*q3)*sin(2*q4))/256 + (3*3^(1/2)*dq2*dqr5*cos(2*q5)*sin(q2)*sin(q3)*sin(q4))/32 + (3*3^(1/2)*dq2*dqr5*sin(2*q5)*cos(q4)*sin(q2)*sin(q3))/64 - (3*3^(1/2)*dq2*dqr5*cos(2*q6)*sin(q2)*sin(q3)*sin(q4))/32 - (3*3^(1/2)*dq3*dqr5*cos(2*q5)*sin(q2)*sin(q3)*sin(q4))/32 - (3*3^(1/2)*dq3*dqr5*sin(2*q5)*cos(q4)*sin(q2)*sin(q3))/64 + (3*3^(1/2)*dq3*dqr5*cos(2*q6)*sin(q2)*sin(q3)*sin(q4))/32 - (5*dq1*dqr4*sin(2*q2)*sin(2*q3)*sin(2*q4)*sin(2*q5)*sin(2*q6))/64 - (3^(1/2)*dq1*dqr4*cos(2*q2)*sin(2*q3)*cos(q4)*cos(q5))/32 + (3^(1/2)*dq1*dqr4*cos(2*q3)*sin(2*q2)*cos(q4)*cos(q5))/32 + (3*dq1*dqr4*cos(2*q2)*cos(2*q3)*cos(2*q4)*cos(2*q6)*sin(q5))/32 + (3*dq1*dqr4*cos(2*q2)*cos(2*q3)*cos(2*q4)*sin(2*q6)*cos(q5))/16 + (3*dq1*dqr4*cos(2*q2)*cos(2*q3)*cos(2*q6)*sin(2*q4)*cos(q5))/64 - (3*dq1*dqr4*cos(2*q2)*cos(2*q3)*sin(2*q4)*sin(2*q6)*sin(q5))/32 + (3*dq1*dqr4*cos(2*q4)*cos(2*q6)*sin(2*q2)*sin(2*q3)*sin(q5))/32 + (3*dq1*dqr4*cos(2*q4)*sin(2*q2)*sin(2*q3)*sin(2*q6)*cos(q5))/16 + (3*dq1*dqr4*cos(2*q6)*sin(2*q2)*sin(2*q3)*sin(2*q4)*cos(q5))/64 - (5*3^(1/2)*dq1*dqr4*cos(2*q2)*cos(2*q5)*cos(2*q6)*sin(2*q3)*cos(q4))/128 + (5*3^(1/2)*dq1*dqr4*cos(2*q3)*cos(2*q5)*cos(2*q6)*sin(2*q2)*cos(q4))/128 - (3*3^(1/2)*dq2*dqr5*cos(2*q6)*cos(q4)*sin(q2)*sin(q3)*sin(q5))/32 - (3*3^(1/2)*dq2*dqr5*sin(2*q6)*cos(q4)*cos(q5)*sin(q2)*sin(q3))/16 + (3*3^(1/2)*dq3*dqr5*cos(2*q6)*cos(q4)*sin(q2)*sin(q3)*sin(q5))/32 + (3*3^(1/2)*dq3*dqr5*sin(2*q6)*cos(q4)*cos(q5)*sin(q2)*sin(q3))/16 + (3^(1/2)*dq1*dqr4*cos(2*q2)*cos(2*q5)*sin(2*q3)*sin(2*q6)*sin(q4))/16 + (5*3^(1/2)*dq1*dqr4*cos(2*q2)*cos(2*q6)*sin(2*q3)*sin(2*q5)*sin(q4))/64 + (3^(1/2)*dq1*dqr4*cos(2*q2)*sin(2*q3)*sin(2*q5)*sin(2*q6)*cos(q4))/32 - (3^(1/2)*dq1*dqr4*cos(2*q3)*sin(2*q2)*sin(2*q5)*sin(2*q6)*cos(q4))/32 - (5*3^(1/2)*dq2*dqr5*cos(2*q5)*cos(2*q6)*sin(q2)*sin(q3)*sin(q4))/32 - (3^(1/2)*dq2*dqr5*cos(2*q5)*sin(2*q6)*cos(q4)*sin(q2)*sin(q3))/16 - (5*3^(1/2)*dq2*dqr5*cos(2*q6)*sin(2*q5)*cos(q4)*sin(q2)*sin(q3))/64 + (5*3^(1/2)*dq3*dqr5*cos(2*q5)*cos(2*q6)*sin(q2)*sin(q3)*sin(q4))/32 + (3^(1/2)*dq3*dqr5*cos(2*q5)*sin(2*q6)*cos(q4)*sin(q2)*sin(q3))/16 + (5*3^(1/2)*dq3*dqr5*cos(2*q6)*sin(2*q5)*cos(q4)*sin(q2)*sin(q3))/64 + (3^(1/2)*dq2*dqr5*sin(2*q5)*sin(2*q6)*sin(q2)*sin(q3)*sin(q4))/8 - (3^(1/2)*dq3*dqr5*sin(2*q5)*sin(2*q6)*sin(q2)*sin(q3)*sin(q4))/8 - (3^(1/2)*dq1*dqr4*cos(2*q2)*cos(2*q6)*sin(2*q3)*cos(q4)*cos(q5))/32 + (3^(1/2)*dq1*dqr4*cos(2*q3)*cos(2*q6)*sin(2*q2)*cos(q4)*cos(q5))/32 + (3^(1/2)*dq1*dqr4*cos(2*q2)*sin(2*q3)*sin(2*q6)*cos(q4)*sin(q5))/16 - (3^(1/2)*dq1*dqr4*cos(2*q3)*sin(2*q2)*sin(2*q6)*cos(q4)*sin(q5))/16;
Y1_20_14=(5*dq3*dqr5*cos(q3)*sin(q2))/32 - (5*dq2*dqr5*cos(q3)*sin(q2))/32 + (3*dq2*dqr5*cos(2*q6)*cos(q3)*sin(q2))/32 - (3*dq3*dqr5*cos(2*q6)*cos(q3)*sin(q2))/32 - (9*dq4*dqr5*sin(2*q5)*sin(q2)*sin(q3))/64 + (3*dq6*dqr5*sin(2*q6)*sin(q2)*sin(q3))/16 - (3*dq2*dqr5*cos(q3)*cos(q5)*sin(q2))/32 + (3*dq3*dqr5*cos(q3)*cos(q5)*sin(q2))/32 - (3*dq2*dqr5*sin(2*q4)*cos(q2)*sin(q3)*sin(q5))/64 + (3*dq2*dqr5*sin(2*q4)*cos(q3)*sin(q2)*sin(q5))/64 + (3*dq3*dqr5*sin(2*q4)*cos(q2)*sin(q3)*sin(q5))/64 - (3*dq3*dqr5*sin(2*q4)*cos(q3)*sin(q2)*sin(q5))/64 - (3*dq2*dqr5*sin(2*q6)*cos(q2)*sin(q3)*sin(q5))/16 + (3*dq2*dqr5*sin(2*q6)*cos(q3)*sin(q2)*sin(q5))/16 + (3*dq3*dqr5*sin(2*q6)*cos(q2)*sin(q3)*sin(q5))/16 - (3*dq3*dqr5*sin(2*q6)*cos(q3)*sin(q2)*sin(q5))/16 - (3*dq4*dqr5*sin(2*q6)*cos(q5)*sin(q2)*sin(q3))/16 - (3*dq5*dqr5*sin(2*q6)*cos(q5)*sin(q2)*sin(q3))/8 - (3*dq6*dqr5*sin(2*q6)*cos(q5)*sin(q2)*sin(q3))/16 + (5*3^(1/2)*dq4*dqr5*cos(q3)*cos(q4)*sin(q2))/32 + (3*dq2*dqr5*cos(2*q4)*cos(2*q5)*cos(q3)*sin(q2))/32 - (3*dq3*dqr5*cos(2*q4)*cos(2*q5)*cos(q3)*sin(q2))/32 - (15*dq2*dqr5*sin(2*q4)*sin(2*q5)*cos(q3)*sin(q2))/128 + (15*dq3*dqr5*sin(2*q4)*sin(2*q5)*cos(q3)*sin(q2))/128 + (3*dq4*dqr5*cos(2*q5)*sin(2*q6)*sin(q2)*sin(q3))/16 + (15*dq4*dqr5*cos(2*q6)*sin(2*q5)*sin(q2)*sin(q3))/64 - (3*dq2*dqr5*cos(2*q4)*cos(q3)*cos(q5)*sin(q2))/32 + (3*dq3*dqr5*cos(2*q4)*cos(q3)*cos(q5)*sin(q2))/32 - (3*dq2*dqr5*cos(2*q6)*cos(q3)*cos(q5)*sin(q2))/32 + (3*dq3*dqr5*cos(2*q6)*cos(q3)*cos(q5)*sin(q2))/32 - (3^(1/2)*dq4*dqr5*cos(q2)*sin(q3)*sin(q4)*sin(q5))/32 + (3^(1/2)*dq4*dqr5*cos(q3)*sin(q2)*sin(q4)*sin(q5))/32 - (3^(1/2)*dq5*dqr5*cos(q2)*sin(q3)*sin(q4)*sin(q5))/16 + (3^(1/2)*dq5*dqr5*cos(q3)*sin(q2)*sin(q4)*sin(q5))/16 - (3^(1/2)*dq6*dqr5*cos(q2)*sin(q3)*sin(q4)*sin(q5))/8 + (3^(1/2)*dq6*dqr5*cos(q3)*sin(q2)*sin(q4)*sin(q5))/8 - (3*dq2*dqr5*cos(2*q4)*cos(2*q6)*cos(q3)*cos(q5)*sin(q2))/32 + (3*dq3*dqr5*cos(2*q4)*cos(2*q6)*cos(q3)*cos(q5)*sin(q2))/32 - (3*dq2*dqr5*cos(2*q4)*sin(2*q6)*cos(q2)*sin(q3)*sin(q5))/16 + (3*dq2*dqr5*cos(2*q4)*sin(2*q6)*cos(q3)*sin(q2)*sin(q5))/16 - (3*dq2*dqr5*cos(2*q6)*sin(2*q4)*cos(q2)*sin(q3)*sin(q5))/64 + (3*dq2*dqr5*cos(2*q6)*sin(2*q4)*cos(q3)*sin(q2)*sin(q5))/64 + (3*dq2*dqr5*sin(2*q4)*sin(2*q6)*cos(q3)*cos(q5)*sin(q2))/32 + (3*dq3*dqr5*cos(2*q4)*sin(2*q6)*cos(q2)*sin(q3)*sin(q5))/16 - (3*dq3*dqr5*cos(2*q4)*sin(2*q6)*cos(q3)*sin(q2)*sin(q5))/16 + (3*dq3*dqr5*cos(2*q6)*sin(2*q4)*cos(q2)*sin(q3)*sin(q5))/64 - (3*dq3*dqr5*cos(2*q6)*sin(2*q4)*cos(q3)*sin(q2)*sin(q5))/64 - (3*dq3*dqr5*sin(2*q4)*sin(2*q6)*cos(q3)*cos(q5)*sin(q2))/32 - (3*3^(1/2)*dq4*dqr5*cos(2*q5)*cos(q3)*cos(q4)*sin(q2))/32 - (3*3^(1/2)*dq4*dqr5*cos(2*q6)*cos(q3)*cos(q4)*sin(q2))/32 - (3*3^(1/2)*dq4*dqr5*sin(2*q5)*cos(q2)*sin(q3)*sin(q4))/64 + (3*3^(1/2)*dq4*dqr5*sin(2*q5)*cos(q3)*sin(q2)*sin(q4))/64 - (3*3^(1/2)*dq6*dqr5*sin(2*q6)*cos(q2)*sin(q3)*sin(q4))/16 + (3*3^(1/2)*dq6*dqr5*sin(2*q6)*cos(q3)*sin(q2)*sin(q4))/16 - (5*dq2*dqr5*cos(2*q4)*cos(2*q5)*cos(2*q6)*cos(q3)*sin(q2))/32 + (5*dq3*dqr5*cos(2*q4)*cos(2*q5)*cos(2*q6)*cos(q3)*sin(q2))/32 + (dq2*dqr5*cos(2*q4)*sin(2*q5)*sin(2*q6)*cos(q3)*sin(q2))/8 + (5*dq2*dqr5*cos(2*q5)*sin(2*q4)*sin(2*q6)*cos(q3)*sin(q2))/32 + (25*dq2*dqr5*cos(2*q6)*sin(2*q4)*sin(2*q5)*cos(q3)*sin(q2))/128 - (dq3*dqr5*cos(2*q4)*sin(2*q5)*sin(2*q6)*cos(q3)*sin(q2))/8 - (5*dq3*dqr5*cos(2*q5)*sin(2*q4)*sin(2*q6)*cos(q3)*sin(q2))/32 - (25*dq3*dqr5*cos(2*q6)*sin(2*q4)*sin(2*q5)*cos(q3)*sin(q2))/128 + (3^(1/2)*dq4*dqr5*cos(q2)*cos(q4)*cos(q5)*sin(q3))/16 - (3^(1/2)*dq4*dqr5*cos(q3)*cos(q4)*cos(q5)*sin(q2))/16 + (3^(1/2)*dq5*dqr5*cos(q2)*cos(q4)*cos(q5)*sin(q3))/8 - (3^(1/2)*dq5*dqr5*cos(q3)*cos(q4)*cos(q5)*sin(q2))/8 + (3^(1/2)*dq6*dqr5*cos(q2)*cos(q4)*cos(q5)*sin(q3))/4 - (3^(1/2)*dq6*dqr5*cos(q3)*cos(q4)*cos(q5)*sin(q2))/4 + (3^(1/2)*dq4*dqr5*cos(2*q6)*cos(q2)*cos(q4)*cos(q5)*sin(q3))/16 - (3^(1/2)*dq4*dqr5*cos(2*q6)*cos(q3)*cos(q4)*cos(q5)*sin(q2))/16 + (3^(1/2)*dq5*dqr5*cos(2*q6)*cos(q2)*cos(q4)*cos(q5)*sin(q3))/8 - (3^(1/2)*dq5*dqr5*cos(2*q6)*cos(q3)*cos(q4)*cos(q5)*sin(q2))/8 + (3^(1/2)*dq6*dqr5*cos(2*q6)*cos(q2)*cos(q4)*cos(q5)*sin(q3))/4 - (3^(1/2)*dq6*dqr5*cos(2*q6)*cos(q3)*cos(q4)*cos(q5)*sin(q2))/4 - (3^(1/2)*dq4*dqr5*cos(2*q6)*cos(q2)*sin(q3)*sin(q4)*sin(q5))/32 + (3^(1/2)*dq4*dqr5*cos(2*q6)*cos(q3)*sin(q2)*sin(q4)*sin(q5))/32 - (3^(1/2)*dq4*dqr5*sin(2*q6)*cos(q2)*cos(q4)*sin(q3)*sin(q5))/8 - (3^(1/2)*dq4*dqr5*sin(2*q6)*cos(q2)*cos(q5)*sin(q3)*sin(q4))/16 + (3^(1/2)*dq4*dqr5*sin(2*q6)*cos(q3)*cos(q4)*sin(q2)*sin(q5))/8 + (3^(1/2)*dq4*dqr5*sin(2*q6)*cos(q3)*cos(q5)*sin(q2)*sin(q4))/16 - (3^(1/2)*dq5*dqr5*cos(2*q6)*cos(q2)*sin(q3)*sin(q4)*sin(q5))/16 + (3^(1/2)*dq5*dqr5*cos(2*q6)*cos(q3)*sin(q2)*sin(q4)*sin(q5))/16 - (3^(1/2)*dq5*dqr5*sin(2*q6)*cos(q2)*cos(q4)*sin(q3)*sin(q5))/4 - (3^(1/2)*dq5*dqr5*sin(2*q6)*cos(q2)*cos(q5)*sin(q3)*sin(q4))/8 + (3^(1/2)*dq5*dqr5*sin(2*q6)*cos(q3)*cos(q4)*sin(q2)*sin(q5))/4 + (3^(1/2)*dq5*dqr5*sin(2*q6)*cos(q3)*cos(q5)*sin(q2)*sin(q4))/8 - (3^(1/2)*dq6*dqr5*cos(2*q6)*cos(q2)*sin(q3)*sin(q4)*sin(q5))/8 + (3^(1/2)*dq6*dqr5*cos(2*q6)*cos(q3)*sin(q2)*sin(q4)*sin(q5))/8 - (3^(1/2)*dq6*dqr5*sin(2*q6)*cos(q2)*cos(q4)*sin(q3)*sin(q5))/8 - (3^(1/2)*dq6*dqr5*sin(2*q6)*cos(q2)*cos(q5)*sin(q3)*sin(q4))/16 + (3^(1/2)*dq6*dqr5*sin(2*q6)*cos(q3)*cos(q4)*sin(q2)*sin(q5))/8 + (3^(1/2)*dq6*dqr5*sin(2*q6)*cos(q3)*cos(q5)*sin(q2)*sin(q4))/16 - (5*3^(1/2)*dq4*dqr5*cos(2*q5)*cos(2*q6)*cos(q2)*cos(q4)*sin(q3))/32 + (5*3^(1/2)*dq4*dqr5*cos(2*q5)*cos(2*q6)*cos(q3)*cos(q4)*sin(q2))/32 + (3^(1/2)*dq4*dqr5*cos(2*q5)*sin(2*q6)*cos(q2)*sin(q3)*sin(q4))/16 - (3^(1/2)*dq4*dqr5*cos(2*q5)*sin(2*q6)*cos(q3)*sin(q2)*sin(q4))/16 + (5*3^(1/2)*dq4*dqr5*cos(2*q6)*sin(2*q5)*cos(q2)*sin(q3)*sin(q4))/64 - (5*3^(1/2)*dq4*dqr5*cos(2*q6)*sin(2*q5)*cos(q3)*sin(q2)*sin(q4))/64 + (3^(1/2)*dq4*dqr5*sin(2*q5)*sin(2*q6)*cos(q2)*cos(q4)*sin(q3))/8 - (3^(1/2)*dq4*dqr5*sin(2*q5)*sin(2*q6)*cos(q3)*cos(q4)*sin(q2))/8;
Y1_20_15=(5*dq2*dqr5*cos(q2)*sin(q3))/32 - (3*dq1*dqr5*cos(2*q4)*sin(q5))/128 - (3*dq1*dqr5*cos(2*q6)*sin(q5))/128 - (3*dq1*dqr5*sin(q5))/128 - (5*dq3*dqr5*cos(q2)*sin(q3))/32 - (3*dq2*dqr5*cos(2*q6)*cos(q2)*sin(q3))/32 + (3*dq3*dqr5*cos(2*q6)*cos(q2)*sin(q3))/32 - (9*dq4*dqr5*sin(2*q5)*cos(q2)*cos(q3))/64 + (3*dq6*dqr5*sin(2*q6)*cos(q2)*cos(q3))/16 - (9*dq1*dqr5*cos(2*q2)*cos(2*q3)*sin(q5))/128 - (3*dq1*dqr5*cos(2*q4)*cos(2*q6)*sin(q5))/128 - (9*dq1*dqr5*sin(2*q2)*sin(2*q3)*sin(q5))/128 + (3*dq1*dqr5*sin(2*q4)*sin(2*q6)*sin(q5))/32 + (3*dq2*dqr5*cos(q2)*cos(q5)*sin(q3))/32 - (3*dq3*dqr5*cos(q2)*cos(q5)*sin(q3))/32 - (3*dq4*dqr5*cos(q2)*cos(q3)*sin(q5))/32 - (3*dq5*dqr5*cos(q2)*cos(q3)*sin(q5))/16 - (3*dq6*dqr5*cos(q2)*cos(q3)*sin(q5))/8 + (5*3^(1/2)*dq2*dqr5*cos(q2)*cos(q3)*sin(q4))/32 - (5*3^(1/2)*dq3*dqr5*cos(q2)*cos(q3)*sin(q4))/32 - (5*3^(1/2)*dq4*dqr5*cos(q2)*cos(q4)*sin(q3))/32 - (3*dq2*dqr5*cos(2*q4)*cos(2*q5)*cos(q2)*sin(q3))/32 + (3*dq3*dqr5*cos(2*q4)*cos(2*q5)*cos(q2)*sin(q3))/32 + (3*dq4*dqr5*cos(2*q5)*sin(2*q6)*cos(q2)*cos(q3))/16 + (15*dq4*dqr5*cos(2*q6)*sin(2*q5)*cos(q2)*cos(q3))/64 + (15*dq2*dqr5*sin(2*q4)*sin(2*q5)*cos(q2)*sin(q3))/128 - (15*dq3*dqr5*sin(2*q4)*sin(2*q5)*cos(q2)*sin(q3))/128 + (3*dq1*dqr5*cos(2*q2)*cos(2*q3)*cos(2*q4)*sin(q5))/128 - (9*dq1*dqr5*cos(2*q2)*cos(2*q3)*cos(2*q6)*sin(q5))/128 + (3*dq1*dqr5*cos(2*q4)*sin(2*q2)*sin(2*q3)*sin(q5))/128 - (9*dq1*dqr5*cos(2*q6)*sin(2*q2)*sin(2*q3)*sin(q5))/128 + (3*dq2*dqr5*cos(2*q4)*cos(q2)*cos(q5)*sin(q3))/32 - (3*dq3*dqr5*cos(2*q4)*cos(q2)*cos(q5)*sin(q3))/32 + (3*dq2*dqr5*cos(2*q6)*cos(q2)*cos(q5)*sin(q3))/32 - (3*dq3*dqr5*cos(2*q6)*cos(q2)*cos(q5)*sin(q3))/32 - (3*dq4*dqr5*cos(2*q6)*cos(q2)*cos(q3)*sin(q5))/32 - (3*dq4*dqr5*sin(2*q6)*cos(q2)*cos(q3)*cos(q5))/16 - (3*dq5*dqr5*cos(2*q6)*cos(q2)*cos(q3)*sin(q5))/16 - (3*dq5*dqr5*sin(2*q6)*cos(q2)*cos(q3)*cos(q5))/8 - (3*dq6*dqr5*cos(2*q6)*cos(q2)*cos(q3)*sin(q5))/8 - (3*dq6*dqr5*sin(2*q6)*cos(q2)*cos(q3)*cos(q5))/16 - (3*3^(1/2)*dq1*dqr5*cos(2*q3)*cos(2*q5)*sin(2*q2)*cos(q4))/32 - (3*dq1*dqr5*sin(2*q2)*sin(2*q3)*sin(2*q4)*sin(2*q6)*sin(q5))/32 + (3*dq2*dqr5*cos(2*q4)*cos(2*q6)*cos(q2)*cos(q5)*sin(q3))/32 - (3*dq3*dqr5*cos(2*q4)*cos(2*q6)*cos(q2)*cos(q5)*sin(q3))/32 - (3*3^(1/2)*dq1*dqr5*cos(2*q2)*sin(2*q3)*sin(2*q5)*sin(q4))/64 + (3*3^(1/2)*dq1*dqr5*cos(2*q3)*sin(2*q2)*sin(2*q5)*sin(q4))/64 - (3*dq2*dqr5*sin(2*q4)*sin(2*q6)*cos(q2)*cos(q5)*sin(q3))/32 + (3*dq3*dqr5*sin(2*q4)*sin(2*q6)*cos(q2)*cos(q5)*sin(q3))/32 + (3*3^(1/2)*dq2*dqr5*cos(2*q5)*cos(q2)*cos(q3)*sin(q4))/32 + (3*3^(1/2)*dq2*dqr5*sin(2*q5)*cos(q2)*cos(q3)*cos(q4))/64 - (3*3^(1/2)*dq2*dqr5*cos(2*q6)*cos(q2)*cos(q3)*sin(q4))/32 - (3*3^(1/2)*dq3*dqr5*cos(2*q5)*cos(q2)*cos(q3)*sin(q4))/32 - (3*3^(1/2)*dq3*dqr5*sin(2*q5)*cos(q2)*cos(q3)*cos(q4))/64 + (3*3^(1/2)*dq3*dqr5*cos(2*q6)*cos(q2)*cos(q3)*sin(q4))/32 + (3*3^(1/2)*dq4*dqr5*cos(2*q5)*cos(q2)*cos(q4)*sin(q3))/32 + (3*3^(1/2)*dq4*dqr5*cos(2*q6)*cos(q2)*cos(q4)*sin(q3))/32 + (5*dq2*dqr5*cos(2*q4)*cos(2*q5)*cos(2*q6)*cos(q2)*sin(q3))/32 - (5*dq3*dqr5*cos(2*q4)*cos(2*q5)*cos(2*q6)*cos(q2)*sin(q3))/32 - (dq2*dqr5*cos(2*q4)*sin(2*q5)*sin(2*q6)*cos(q2)*sin(q3))/8 - (5*dq2*dqr5*cos(2*q5)*sin(2*q4)*sin(2*q6)*cos(q2)*sin(q3))/32 - (25*dq2*dqr5*cos(2*q6)*sin(2*q4)*sin(2*q5)*cos(q2)*sin(q3))/128 + (dq3*dqr5*cos(2*q4)*sin(2*q5)*sin(2*q6)*cos(q2)*sin(q3))/8 + (5*dq3*dqr5*cos(2*q5)*sin(2*q4)*sin(2*q6)*cos(q2)*sin(q3))/32 + (25*dq3*dqr5*cos(2*q6)*sin(2*q4)*sin(2*q5)*cos(q2)*sin(q3))/128 + (3^(1/2)*dq1*dqr5*cos(2*q2)*sin(2*q3)*cos(q4)*cos(q5))/32 - (3^(1/2)*dq1*dqr5*cos(2*q3)*sin(2*q2)*cos(q4)*cos(q5))/32 + (3^(1/2)*dq1*dqr5*cos(2*q2)*sin(2*q3)*sin(q4)*sin(q5))/32 - (3^(1/2)*dq1*dqr5*cos(2*q3)*sin(2*q2)*sin(q4)*sin(q5))/32 + (3*dq1*dqr5*cos(2*q2)*cos(2*q3)*cos(2*q4)*cos(2*q6)*sin(q5))/128 - (3*3^(1/2)*dq2*dqr5*cos(q2)*cos(q3)*cos(q4)*sin(q5))/32 + (3*3^(1/2)*dq3*dqr5*cos(q2)*cos(q3)*cos(q4)*sin(q5))/32 - (3*dq1*dqr5*cos(2*q2)*cos(2*q3)*sin(2*q4)*sin(2*q6)*sin(q5))/32 + (3*dq1*dqr5*cos(2*q4)*cos(2*q6)*sin(2*q2)*sin(2*q3)*sin(q5))/128 - (3*3^(1/2)*dq2*dqr5*cos(2*q6)*cos(q2)*cos(q3)*cos(q4)*sin(q5))/32 - (3*3^(1/2)*dq2*dqr5*sin(2*q6)*cos(q2)*cos(q3)*cos(q4)*cos(q5))/16 + (3*3^(1/2)*dq3*dqr5*cos(2*q6)*cos(q2)*cos(q3)*cos(q4)*sin(q5))/32 + (3*3^(1/2)*dq3*dqr5*sin(2*q6)*cos(q2)*cos(q3)*cos(q4)*cos(q5))/16 + (5*3^(1/2)*dq1*dqr5*cos(2*q3)*cos(2*q5)*cos(2*q6)*sin(2*q2)*cos(q4))/32 + (3^(1/2)*dq1*dqr5*cos(2*q2)*cos(2*q5)*sin(2*q3)*sin(2*q6)*sin(q4))/16 + (5*3^(1/2)*dq1*dqr5*cos(2*q2)*cos(2*q6)*sin(2*q3)*sin(2*q5)*sin(q4))/64 - (3^(1/2)*dq1*dqr5*cos(2*q3)*cos(2*q5)*sin(2*q2)*sin(2*q6)*sin(q4))/16 - (5*3^(1/2)*dq1*dqr5*cos(2*q3)*cos(2*q6)*sin(2*q2)*sin(2*q5)*sin(q4))/64 - (3^(1/2)*dq1*dqr5*cos(2*q3)*sin(2*q2)*sin(2*q5)*sin(2*q6)*cos(q4))/8 - (5*3^(1/2)*dq2*dqr5*cos(2*q5)*cos(2*q6)*cos(q2)*cos(q3)*sin(q4))/32 - (3^(1/2)*dq2*dqr5*cos(2*q5)*sin(2*q6)*cos(q2)*cos(q3)*cos(q4))/16 - (5*3^(1/2)*dq2*dqr5*cos(2*q6)*sin(2*q5)*cos(q2)*cos(q3)*cos(q4))/64 + (5*3^(1/2)*dq3*dqr5*cos(2*q5)*cos(2*q6)*cos(q2)*cos(q3)*sin(q4))/32 + (3^(1/2)*dq3*dqr5*cos(2*q5)*sin(2*q6)*cos(q2)*cos(q3)*cos(q4))/16 + (5*3^(1/2)*dq3*dqr5*cos(2*q6)*sin(2*q5)*cos(q2)*cos(q3)*cos(q4))/64 + (3^(1/2)*dq2*dqr5*sin(2*q5)*sin(2*q6)*cos(q2)*cos(q3)*sin(q4))/8 - (3^(1/2)*dq3*dqr5*sin(2*q5)*sin(2*q6)*cos(q2)*cos(q3)*sin(q4))/8 + (3^(1/2)*dq1*dqr5*cos(2*q2)*cos(2*q6)*sin(2*q3)*cos(q4)*cos(q5))/32 - (3^(1/2)*dq1*dqr5*cos(2*q3)*cos(2*q6)*sin(2*q2)*cos(q4)*cos(q5))/32 + (3^(1/2)*dq1*dqr5*cos(2*q2)*cos(2*q6)*sin(2*q3)*sin(q4)*sin(q5))/32 - (3^(1/2)*dq1*dqr5*cos(2*q2)*sin(2*q3)*sin(2*q6)*cos(q4)*sin(q5))/16 + (3^(1/2)*dq1*dqr5*cos(2*q2)*sin(2*q3)*sin(2*q6)*cos(q5)*sin(q4))/16 - (3^(1/2)*dq1*dqr5*cos(2*q3)*cos(2*q6)*sin(2*q2)*sin(q4)*sin(q5))/32 + (3^(1/2)*dq1*dqr5*cos(2*q3)*sin(2*q2)*sin(2*q6)*cos(q4)*sin(q5))/16 - (3^(1/2)*dq1*dqr5*cos(2*q3)*sin(2*q2)*sin(2*q6)*cos(q5)*sin(q4))/16;
Y1_20_16=(15*dq1*dqr5*cos(2*q4)*sin(2*q5))/256 - (3*dq1*dqr5*sin(2*q4)*cos(q5))/64 - (3*dq1*dqr5*sin(2*q6)*cos(q5))/64 - (9*dq1*dqr5*sin(2*q5))/256 + (3*dq1*dqr5*cos(2*q5)*sin(2*q4))/64 + (3*dq1*dqr5*cos(2*q5)*sin(2*q6))/64 + (15*dq1*dqr5*cos(2*q6)*sin(2*q5))/256 - (3*dq4*dqr6*sin(2*q6)*sin(q2)*sin(q3))/64 + (3*dq5*dqr6*sin(2*q6)*sin(q2)*sin(q3))/16 - (3*dq1*dqr5*cos(2*q4)*sin(2*q6)*cos(q5))/64 - (3*dq1*dqr5*cos(2*q6)*sin(2*q4)*cos(q5))/64 - (27*dq1*dqr5*cos(2*q2)*cos(2*q3)*sin(2*q5))/256 - (5*dq1*dqr5*cos(2*q4)*cos(2*q5)*sin(2*q6))/64 - (25*dq1*dqr5*cos(2*q4)*cos(2*q6)*sin(2*q5))/256 - (5*dq1*dqr5*cos(2*q5)*cos(2*q6)*sin(2*q4))/64 - (3*dq5*dqr6*sin(q2)*sin(q3)*sin(q5))/8 - (27*dq1*dqr5*sin(2*q2)*sin(2*q3)*sin(2*q5))/256 + (dq1*dqr5*sin(2*q4)*sin(2*q5)*sin(2*q6))/16 - (15*dq1*dqr5*cos(2*q2)*cos(2*q3)*cos(2*q4)*sin(2*q5))/256 - (3*dq1*dqr5*cos(2*q2)*cos(2*q3)*cos(2*q5)*sin(2*q4))/64 + (9*dq1*dqr5*cos(2*q2)*cos(2*q3)*cos(2*q5)*sin(2*q6))/64 + (45*dq1*dqr5*cos(2*q2)*cos(2*q3)*cos(2*q6)*sin(2*q5))/256 - (3*dq4*dqr6*cos(2*q6)*sin(q2)*sin(q3)*sin(q5))/8 - (3*dq4*dqr6*sin(2*q6)*cos(q5)*sin(q2)*sin(q3))/16 - (3*dq5*dqr6*cos(2*q6)*sin(q2)*sin(q3)*sin(q5))/8 - (3*dq5*dqr6*sin(2*q6)*cos(q5)*sin(q2)*sin(q3))/16 + (3^(1/2)*dq4*dqr6*cos(q3)*cos(q4)*sin(q2))/8 - (15*dq1*dqr5*cos(2*q4)*sin(2*q2)*sin(2*q3)*sin(2*q5))/256 - (3*dq1*dqr5*cos(2*q5)*sin(2*q2)*sin(2*q3)*sin(2*q4))/64 + (9*dq1*dqr5*cos(2*q5)*sin(2*q2)*sin(2*q3)*sin(2*q6))/64 + (45*dq1*dqr5*cos(2*q6)*sin(2*q2)*sin(2*q3)*sin(2*q5))/256 + (3^(1/2)*dq2*dqr6*sin(q2)*sin(q3)*sin(q4))/8 - (3^(1/2)*dq3*dqr6*sin(q2)*sin(q3)*sin(q4))/8 + (15*dq4*dqr6*cos(2*q5)*sin(2*q6)*sin(q2)*sin(q3))/64 + (3*dq4*dqr6*cos(2*q6)*sin(2*q5)*sin(q2)*sin(q3))/16 + (3*dq1*dqr5*cos(2*q2)*cos(2*q3)*sin(2*q4)*cos(q5))/64 - (9*dq1*dqr5*cos(2*q2)*cos(2*q3)*sin(2*q6)*cos(q5))/64 + (3*dq1*dqr5*sin(2*q2)*sin(2*q3)*sin(2*q4)*cos(q5))/64 - (9*dq1*dqr5*sin(2*q2)*sin(2*q3)*sin(2*q6)*cos(q5))/64 + (3*3^(1/2)*dq1*dqr5*cos(2*q2)*cos(2*q5)*sin(2*q3)*cos(q4))/32 - (3^(1/2)*dq2*dqr6*cos(q4)*sin(q2)*sin(q3)*sin(q5))/4 - (3^(1/2)*dq2*dqr6*cos(q5)*sin(q2)*sin(q3)*sin(q4))/8 + (3^(1/2)*dq3*dqr6*cos(q4)*sin(q2)*sin(q3)*sin(q5))/4 + (3^(1/2)*dq3*dqr6*cos(q5)*sin(q2)*sin(q3)*sin(q4))/8 + (3^(1/2)*dq4*dqr6*cos(q3)*sin(q2)*sin(q4)*sin(q5))/4 + (3^(1/2)*dq5*dqr6*cos(q3)*sin(q2)*sin(q4)*sin(q5))/8 - (3*dq2*dqr6*cos(2*q4)*cos(2*q6)*cos(q3)*cos(q5)*sin(q2))/8 + (5*dq1*dqr5*cos(2*q2)*cos(2*q3)*cos(2*q4)*cos(2*q5)*sin(2*q6))/64 + (25*dq1*dqr5*cos(2*q2)*cos(2*q3)*cos(2*q4)*cos(2*q6)*sin(2*q5))/256 + (5*dq1*dqr5*cos(2*q2)*cos(2*q3)*cos(2*q5)*cos(2*q6)*sin(2*q4))/64 + (3*dq2*dqr6*cos(2*q4)*sin(2*q6)*cos(q3)*sin(q2)*sin(q5))/16 + (3*dq2*dqr6*cos(2*q6)*sin(2*q4)*cos(q3)*sin(q2)*sin(q5))/16 + (3*dq2*dqr6*sin(2*q4)*sin(2*q6)*cos(q3)*cos(q5)*sin(q2))/32 - (3*dq3*dqr6*cos(2*q4)*sin(2*q6)*cos(q3)*sin(q2)*sin(q5))/16 - (3*dq3*dqr6*cos(2*q6)*sin(2*q4)*cos(q3)*sin(q2)*sin(q5))/16 - (dq1*dqr5*cos(2*q2)*cos(2*q3)*sin(2*q4)*sin(2*q5)*sin(2*q6))/16 + (5*dq1*dqr5*cos(2*q4)*cos(2*q5)*sin(2*q2)*sin(2*q3)*sin(2*q6))/64 + (25*dq1*dqr5*cos(2*q4)*cos(2*q6)*sin(2*q2)*sin(2*q3)*sin(2*q5))/256 + (5*dq1*dqr5*cos(2*q5)*cos(2*q6)*sin(2*q2)*sin(2*q3)*sin(2*q4))/64 + (9*3^(1/2)*dq2*dqr6*sin(2*q6)*cos(q4)*sin(q2)*sin(q3))/64 - (9*3^(1/2)*dq3*dqr6*sin(2*q6)*cos(q4)*sin(q2)*sin(q3))/64 + (9*3^(1/2)*dq4*dqr6*sin(2*q6)*cos(q3)*sin(q2)*sin(q4))/64 + (3*3^(1/2)*dq5*dqr6*sin(2*q6)*cos(q3)*sin(q2)*sin(q4))/16 - (dq1*dqr5*sin(2*q2)*sin(2*q3)*sin(2*q4)*sin(2*q5)*sin(2*q6))/16 + (3*dq1*dqr5*cos(2*q2)*cos(2*q3)*cos(2*q4)*sin(2*q6)*cos(q5))/64 + (3*dq1*dqr5*cos(2*q2)*cos(2*q3)*cos(2*q6)*sin(2*q4)*cos(q5))/64 - (3^(1/2)*dq4*dqr6*cos(q3)*cos(q4)*cos(q5)*sin(q2))/8 - (3^(1/2)*dq5*dqr6*cos(q3)*cos(q4)*cos(q5)*sin(q2))/4 + (3*dq1*dqr5*cos(2*q4)*sin(2*q2)*sin(2*q3)*sin(2*q6)*cos(q5))/64 + (3*dq1*dqr5*cos(2*q6)*sin(2*q2)*sin(2*q3)*sin(2*q4)*cos(q5))/64 - (3^(1/2)*dq4*dqr6*cos(2*q6)*cos(q3)*cos(q4)*cos(q5)*sin(q2))/8 - (3^(1/2)*dq5*dqr6*cos(2*q6)*cos(q3)*cos(q4)*cos(q5)*sin(q2))/4 - (5*3^(1/2)*dq1*dqr5*cos(2*q2)*cos(2*q5)*cos(2*q6)*sin(2*q3)*cos(q4))/32 - (3^(1/2)*dq2*dqr6*cos(2*q6)*cos(q4)*sin(q2)*sin(q3)*sin(q5))/8 + (3^(1/2)*dq2*dqr6*cos(2*q6)*cos(q5)*sin(q2)*sin(q3)*sin(q4))/8 - (3^(1/2)*dq2*dqr6*sin(2*q6)*cos(q4)*cos(q5)*sin(q2)*sin(q3))/16 + (3^(1/2)*dq3*dqr6*cos(2*q6)*cos(q4)*sin(q2)*sin(q3)*sin(q5))/8 - (3^(1/2)*dq3*dqr6*cos(2*q6)*cos(q5)*sin(q2)*sin(q3)*sin(q4))/8 + (3^(1/2)*dq3*dqr6*sin(2*q6)*cos(q4)*cos(q5)*sin(q2)*sin(q3))/16 - (3^(1/2)*dq4*dqr6*cos(2*q6)*cos(q3)*sin(q2)*sin(q4)*sin(q5))/8 + (3^(1/2)*dq4*dqr6*sin(2*q6)*cos(q3)*cos(q4)*sin(q2)*sin(q5))/16 - (3^(1/2)*dq4*dqr6*sin(2*q6)*cos(q3)*cos(q5)*sin(q2)*sin(q4))/16 + (3^(1/2)*dq5*dqr6*cos(2*q6)*cos(q3)*sin(q2)*sin(q4)*sin(q5))/8 + (3^(1/2)*dq5*dqr6*sin(2*q6)*cos(q3)*cos(q4)*sin(q2)*sin(q5))/8 + (3^(1/2)*dq5*dqr6*sin(2*q6)*cos(q3)*cos(q5)*sin(q2)*sin(q4))/16 + (3^(1/2)*dq1*dqr5*cos(2*q2)*sin(2*q3)*sin(2*q5)*sin(2*q6)*cos(q4))/8 - (3^(1/2)*dq2*dqr6*sin(2*q6)*sin(q2)*sin(q3)*sin(q4)*sin(q5))/16 + (3^(1/2)*dq3*dqr6*sin(2*q6)*sin(q2)*sin(q3)*sin(q4)*sin(q5))/16 + (3^(1/2)*dq4*dqr6*cos(2*q5)*cos(2*q6)*cos(q3)*cos(q4)*sin(q2))/8 - (3^(1/2)*dq2*dqr6*cos(2*q5)*cos(2*q6)*sin(q2)*sin(q3)*sin(q4))/8 - (5*3^(1/2)*dq2*dqr6*cos(2*q5)*sin(2*q6)*cos(q4)*sin(q2)*sin(q3))/64 - (3^(1/2)*dq2*dqr6*cos(2*q6)*sin(2*q5)*cos(q4)*sin(q2)*sin(q3))/16 + (3^(1/2)*dq3*dqr6*cos(2*q5)*cos(2*q6)*sin(q2)*sin(q3)*sin(q4))/8 + (5*3^(1/2)*dq3*dqr6*cos(2*q5)*sin(2*q6)*cos(q4)*sin(q2)*sin(q3))/64 + (3^(1/2)*dq3*dqr6*cos(2*q6)*sin(2*q5)*cos(q4)*sin(q2)*sin(q3))/16 - (5*3^(1/2)*dq4*dqr6*cos(2*q5)*sin(2*q6)*cos(q3)*sin(q2)*sin(q4))/64 - (3^(1/2)*dq4*dqr6*cos(2*q6)*sin(2*q5)*cos(q3)*sin(q2)*sin(q4))/16 - (5*3^(1/2)*dq4*dqr6*sin(2*q5)*sin(2*q6)*cos(q3)*cos(q4)*sin(q2))/32 + (5*3^(1/2)*dq2*dqr6*sin(2*q5)*sin(2*q6)*sin(q2)*sin(q3)*sin(q4))/32 - (5*3^(1/2)*dq3*dqr6*sin(2*q5)*sin(2*q6)*sin(q2)*sin(q3)*sin(q4))/32;
Y1_20_17=(dq2*dqr6*cos(q2)*sin(q3))/8 - (3*dq1*dqr6*cos(2*q6)*sin(q5))/32 - (dq2*dqr6*cos(q3)*sin(q2))/8 - (dq3*dqr6*cos(q2)*sin(q3))/8 + (dq3*dqr6*cos(q3)*sin(q2))/8 - (3*dq1*dqr6*cos(2*q4)*cos(2*q6)*sin(q5))/32 + (3*dq1*dqr6*sin(2*q4)*sin(2*q6)*sin(q5))/32 + (3*dq2*dqr6*cos(q2)*cos(q5)*sin(q3))/8 - (3*dq2*dqr6*cos(q3)*cos(q5)*sin(q2))/8 - (3*dq3*dqr6*cos(q2)*cos(q5)*sin(q3))/8 + (3*dq3*dqr6*cos(q3)*cos(q5)*sin(q2))/8 - (3*dq5*dqr6*cos(q2)*cos(q3)*sin(q5))/8 + (3^(1/2)*dq2*dqr6*cos(q2)*cos(q3)*sin(q4))/8 - (3^(1/2)*dq3*dqr6*cos(q2)*cos(q3)*sin(q4))/8 - (3^(1/2)*dq4*dqr6*cos(q2)*cos(q4)*sin(q3))/8 - (27*dq2*dqr6*sin(2*q4)*sin(2*q6)*cos(q2)*sin(q3))/128 + (27*dq2*dqr6*sin(2*q4)*sin(2*q6)*cos(q3)*sin(q2))/128 + (27*dq3*dqr6*sin(2*q4)*sin(2*q6)*cos(q2)*sin(q3))/128 - (27*dq3*dqr6*sin(2*q4)*sin(2*q6)*cos(q3)*sin(q2))/128 - (9*dq1*dqr6*cos(2*q2)*cos(2*q3)*cos(2*q6)*sin(q5))/32 - (9*dq1*dqr6*cos(2*q6)*sin(2*q2)*sin(2*q3)*sin(q5))/32 - (3*dq4*dqr6*cos(2*q6)*cos(q2)*cos(q3)*sin(q5))/8 - (3*dq5*dqr6*cos(2*q6)*cos(q2)*cos(q3)*sin(q5))/8 - (3^(1/2)*dq4*dqr6*cos(q2)*sin(q3)*sin(q4)*sin(q5))/4 - (3^(1/2)*dq5*dqr6*cos(q2)*sin(q3)*sin(q4)*sin(q5))/8 - (3*dq1*dqr6*sin(2*q2)*sin(2*q3)*sin(2*q4)*sin(2*q6)*sin(q5))/32 + (3*dq2*dqr6*cos(2*q4)*cos(2*q6)*cos(q2)*cos(q5)*sin(q3))/8 - (3*dq3*dqr6*cos(2*q4)*cos(2*q6)*cos(q2)*cos(q5)*sin(q3))/8 + (3*dq3*dqr6*cos(2*q4)*cos(2*q6)*cos(q3)*cos(q5)*sin(q2))/8 - (9*3^(1/2)*dq1*dqr6*cos(2*q2)*sin(2*q3)*sin(2*q6)*sin(q4))/64 + (9*3^(1/2)*dq1*dqr6*cos(2*q3)*sin(2*q2)*sin(2*q6)*sin(q4))/64 - (3*dq2*dqr6*cos(2*q4)*sin(2*q6)*cos(q2)*sin(q3)*sin(q5))/16 - (3*dq2*dqr6*cos(2*q6)*sin(2*q4)*cos(q2)*sin(q3)*sin(q5))/16 - (3*dq2*dqr6*sin(2*q4)*sin(2*q6)*cos(q2)*cos(q5)*sin(q3))/32 + (3*dq3*dqr6*cos(2*q4)*sin(2*q6)*cos(q2)*sin(q3)*sin(q5))/16 + (3*dq3*dqr6*cos(2*q6)*sin(2*q4)*cos(q2)*sin(q3)*sin(q5))/16 + (3*dq3*dqr6*sin(2*q4)*sin(2*q6)*cos(q2)*cos(q5)*sin(q3))/32 - (3*dq3*dqr6*sin(2*q4)*sin(2*q6)*cos(q3)*cos(q5)*sin(q2))/32 - (9*3^(1/2)*dq4*dqr6*sin(2*q6)*cos(q2)*sin(q3)*sin(q4))/64 - (3*3^(1/2)*dq5*dqr6*sin(2*q6)*cos(q2)*sin(q3)*sin(q4))/16 + (dq2*dqr6*cos(2*q4)*cos(2*q5)*cos(2*q6)*cos(q2)*sin(q3))/8 - (dq2*dqr6*cos(2*q4)*cos(2*q5)*cos(2*q6)*cos(q3)*sin(q2))/8 - (dq3*dqr6*cos(2*q4)*cos(2*q5)*cos(2*q6)*cos(q2)*sin(q3))/8 + (dq3*dqr6*cos(2*q4)*cos(2*q5)*cos(2*q6)*cos(q3)*sin(q2))/8 - (5*dq2*dqr6*cos(2*q4)*sin(2*q5)*sin(2*q6)*cos(q2)*sin(q3))/32 + (5*dq2*dqr6*cos(2*q4)*sin(2*q5)*sin(2*q6)*cos(q3)*sin(q2))/32 - (25*dq2*dqr6*cos(2*q5)*sin(2*q4)*sin(2*q6)*cos(q2)*sin(q3))/128 + (25*dq2*dqr6*cos(2*q5)*sin(2*q4)*sin(2*q6)*cos(q3)*sin(q2))/128 - (5*dq2*dqr6*cos(2*q6)*sin(2*q4)*sin(2*q5)*cos(q2)*sin(q3))/32 + (5*dq2*dqr6*cos(2*q6)*sin(2*q4)*sin(2*q5)*cos(q3)*sin(q2))/32 + (5*dq3*dqr6*cos(2*q4)*sin(2*q5)*sin(2*q6)*cos(q2)*sin(q3))/32 - (5*dq3*dqr6*cos(2*q4)*sin(2*q5)*sin(2*q6)*cos(q3)*sin(q2))/32 + (25*dq3*dqr6*cos(2*q5)*sin(2*q4)*sin(2*q6)*cos(q2)*sin(q3))/128 - (25*dq3*dqr6*cos(2*q5)*sin(2*q4)*sin(2*q6)*cos(q3)*sin(q2))/128 + (5*dq3*dqr6*cos(2*q6)*sin(2*q4)*sin(2*q5)*cos(q2)*sin(q3))/32 - (5*dq3*dqr6*cos(2*q6)*sin(2*q4)*sin(2*q5)*cos(q3)*sin(q2))/32 + (3*dq1*dqr6*cos(2*q2)*cos(2*q3)*cos(2*q4)*cos(2*q6)*sin(q5))/32 - (3^(1/2)*dq2*dqr6*cos(q2)*cos(q3)*cos(q4)*sin(q5))/4 - (3^(1/2)*dq2*dqr6*cos(q2)*cos(q3)*cos(q5)*sin(q4))/8 + (3^(1/2)*dq3*dqr6*cos(q2)*cos(q3)*cos(q4)*sin(q5))/4 + (3^(1/2)*dq3*dqr6*cos(q2)*cos(q3)*cos(q5)*sin(q4))/8 + (3^(1/2)*dq4*dqr6*cos(q2)*cos(q4)*cos(q5)*sin(q3))/8 + (3^(1/2)*dq5*dqr6*cos(q2)*cos(q4)*cos(q5)*sin(q3))/4 - (3*dq1*dqr6*cos(2*q2)*cos(2*q3)*sin(2*q4)*sin(2*q6)*sin(q5))/32 + (3*dq1*dqr6*cos(2*q4)*cos(2*q6)*sin(2*q2)*sin(2*q3)*sin(q5))/32 - (3^(1/2)*dq2*dqr6*cos(2*q6)*cos(q2)*cos(q3)*cos(q4)*sin(q5))/8 + (3^(1/2)*dq2*dqr6*cos(2*q6)*cos(q2)*cos(q3)*cos(q5)*sin(q4))/8 - (3^(1/2)*dq2*dqr6*sin(2*q6)*cos(q2)*cos(q3)*cos(q4)*cos(q5))/16 + (3^(1/2)*dq3*dqr6*cos(2*q6)*cos(q2)*cos(q3)*cos(q4)*sin(q5))/8 - (3^(1/2)*dq3*dqr6*cos(2*q6)*cos(q2)*cos(q3)*cos(q5)*sin(q4))/8 + (3^(1/2)*dq3*dqr6*sin(2*q6)*cos(q2)*cos(q3)*cos(q4)*cos(q5))/16 + (3^(1/2)*dq4*dqr6*cos(2*q6)*cos(q2)*cos(q4)*cos(q5)*sin(q3))/8 + (3^(1/2)*dq5*dqr6*cos(2*q6)*cos(q2)*cos(q4)*cos(q5)*sin(q3))/4 - (3^(1/2)*dq2*dqr6*sin(2*q6)*cos(q2)*cos(q3)*sin(q4)*sin(q5))/16 + (3^(1/2)*dq3*dqr6*sin(2*q6)*cos(q2)*cos(q3)*sin(q4)*sin(q5))/16 + (3^(1/2)*dq4*dqr6*cos(2*q6)*cos(q2)*sin(q3)*sin(q4)*sin(q5))/8 - (3^(1/2)*dq4*dqr6*sin(2*q6)*cos(q2)*cos(q4)*sin(q3)*sin(q5))/16 + (3^(1/2)*dq4*dqr6*sin(2*q6)*cos(q2)*cos(q5)*sin(q3)*sin(q4))/16 - (3^(1/2)*dq5*dqr6*cos(2*q6)*cos(q2)*sin(q3)*sin(q4)*sin(q5))/8 - (3^(1/2)*dq5*dqr6*sin(2*q6)*cos(q2)*cos(q4)*sin(q3)*sin(q5))/8 - (3^(1/2)*dq5*dqr6*sin(2*q6)*cos(q2)*cos(q5)*sin(q3)*sin(q4))/16 + (5*3^(1/2)*dq1*dqr6*cos(2*q2)*cos(2*q5)*sin(2*q3)*sin(2*q6)*sin(q4))/64 + (3^(1/2)*dq1*dqr6*cos(2*q2)*cos(2*q6)*sin(2*q3)*sin(2*q5)*sin(q4))/16 - (5*3^(1/2)*dq1*dqr6*cos(2*q3)*cos(2*q5)*sin(2*q2)*sin(2*q6)*sin(q4))/64 - (3^(1/2)*dq1*dqr6*cos(2*q3)*cos(2*q6)*sin(2*q2)*sin(2*q5)*sin(q4))/16 - (3^(1/2)*dq2*dqr6*cos(2*q5)*cos(2*q6)*cos(q2)*cos(q3)*sin(q4))/8 - (3^(1/2)*dq2*dqr6*cos(2*q6)*sin(2*q5)*cos(q2)*cos(q3)*cos(q4))/16 + (3^(1/2)*dq3*dqr6*cos(2*q5)*cos(2*q6)*cos(q2)*cos(q3)*sin(q4))/8 - (3^(1/2)*dq4*dqr6*cos(2*q5)*cos(2*q6)*cos(q2)*cos(q4)*sin(q3))/8 + (5*3^(1/2)*dq2*dqr6*sin(2*q5)*sin(2*q6)*cos(q2)*cos(q3)*sin(q4))/32 - (5*3^(1/2)*dq3*dqr6*sin(2*q5)*sin(2*q6)*cos(q2)*cos(q3)*sin(q4))/32 + (5*3^(1/2)*dq4*dqr6*cos(2*q5)*sin(2*q6)*cos(q2)*sin(q3)*sin(q4))/64 + (3^(1/2)*dq4*dqr6*cos(2*q6)*sin(2*q5)*cos(q2)*sin(q3)*sin(q4))/16 + (5*3^(1/2)*dq4*dqr6*sin(2*q5)*sin(2*q6)*cos(q2)*cos(q4)*sin(q3))/32 + (3^(1/2)*dq1*dqr6*cos(2*q2)*cos(2*q6)*sin(2*q3)*sin(q4)*sin(q5))/8 - (3^(1/2)*dq1*dqr6*cos(2*q2)*sin(2*q3)*sin(2*q6)*cos(q4)*sin(q5))/16 + (3^(1/2)*dq1*dqr6*cos(2*q2)*sin(2*q3)*sin(2*q6)*cos(q5)*sin(q4))/16 - (3^(1/2)*dq1*dqr6*cos(2*q3)*cos(2*q6)*sin(2*q2)*sin(q4)*sin(q5))/8 + (3^(1/2)*dq1*dqr6*cos(2*q3)*sin(2*q2)*sin(2*q6)*cos(q4)*sin(q5))/16 - (3^(1/2)*dq1*dqr6*cos(2*q3)*sin(2*q2)*sin(2*q6)*cos(q5)*sin(q4))/16;
Y1_20_18=(43*ddqr4*sin(q2)*sin(q3))/64 - (3*dq1*dqr6*sin(2*q6))/256 + (5*ddqr5*sin(q2)*sin(q3))/16 + (ddqr6*sin(q2)*sin(q3))/4 - (3*dq1*dqr6*sin(2*q6)*cos(q5))/64 + (3*ddqr4*cos(q5)*sin(q2)*sin(q3))/16 + (3*ddqr5*cos(q5)*sin(q2)*sin(q3))/16 + (3*ddqr6*cos(q5)*sin(q2)*sin(q3))/4 - (27*dq1*dqr6*cos(2*q4)*sin(2*q6))/256 + (15*dq1*dqr6*cos(2*q5)*sin(2*q6))/256 + (3*dq1*dqr6*cos(2*q6)*sin(2*q5))/64 + (9*ddqr4*cos(2*q5)*sin(q2)*sin(q3))/64 + (3*ddqr4*cos(2*q6)*sin(q2)*sin(q3))/64 - (3*ddqr5*cos(2*q6)*sin(q2)*sin(q3))/16 + (3*ddqr4*sin(2*q5)*sin(2*q6)*sin(q2)*sin(q3))/16 - (3*dq4*dqr6*sin(2*q6)*cos(q2)*cos(q3))/64 + (3*dq5*dqr6*sin(2*q6)*cos(q2)*cos(q3))/16 - (3*dq1*dqr6*cos(2*q4)*sin(2*q6)*cos(q5))/64 - (3*dq1*dqr6*cos(2*q6)*sin(2*q4)*cos(q5))/16 + (3*ddqr4*cos(2*q6)*cos(q5)*sin(q2)*sin(q3))/16 + (3*ddqr5*cos(2*q6)*cos(q5)*sin(q2)*sin(q3))/16 - (3*ddqr4*sin(2*q6)*sin(q2)*sin(q3)*sin(q5))/8 - (3*ddqr5*sin(2*q6)*sin(q2)*sin(q3)*sin(q5))/8 - (3^(1/2)*ddqr2*cos(q4)*sin(q2)*sin(q3))/64 + (3^(1/2)*ddqr3*cos(q4)*sin(q2)*sin(q3))/64 - (9*dq1*dqr6*cos(2*q2)*cos(2*q3)*sin(2*q6))/256 - (25*dq1*dqr6*cos(2*q4)*cos(2*q5)*sin(2*q6))/256 - (5*dq1*dqr6*cos(2*q4)*cos(2*q6)*sin(2*q5))/64 - (dq1*dqr6*cos(2*q5)*cos(2*q6)*sin(2*q4))/16 - (9*dq1*dqr6*sin(2*q2)*sin(2*q3)*sin(2*q6))/256 + (5*dq1*dqr6*sin(2*q4)*sin(2*q5)*sin(2*q6))/64 - (15*ddqr4*cos(2*q5)*cos(2*q6)*sin(q2)*sin(q3))/64 + (27*dq1*dqr6*cos(2*q2)*cos(2*q3)*cos(2*q4)*sin(2*q6))/256 + (45*dq1*dqr6*cos(2*q2)*cos(2*q3)*cos(2*q5)*sin(2*q6))/256 + (9*dq1*dqr6*cos(2*q2)*cos(2*q3)*cos(2*q6)*sin(2*q5))/64 + (3*3^(1/2)*ddqr2*sin(2*q5)*sin(q2)*sin(q3)*sin(q4))/32 - (3*3^(1/2)*ddqr3*sin(2*q5)*sin(q2)*sin(q3)*sin(q4))/32 + (27*dq1*dqr6*cos(2*q4)*sin(2*q2)*sin(2*q3)*sin(2*q6))/256 + (45*dq1*dqr6*cos(2*q5)*sin(2*q2)*sin(2*q3)*sin(2*q6))/256 + (9*dq1*dqr6*cos(2*q6)*sin(2*q2)*sin(2*q3)*sin(2*q5))/64 + (15*dq4*dqr6*cos(2*q5)*sin(2*q6)*cos(q2)*cos(q3))/64 + (3*dq4*dqr6*cos(2*q6)*sin(2*q5)*cos(q2)*cos(q3))/16 + (3^(1/2)*ddqr2*cos(q4)*cos(q5)*sin(q2)*sin(q3))/16 - (3^(1/2)*ddqr3*cos(q4)*cos(q5)*sin(q2)*sin(q3))/16 + (3^(1/2)*ddqr4*cos(q3)*cos(q5)*sin(q2)*sin(q4))/16 - (9*dq1*dqr6*cos(2*q2)*cos(2*q3)*sin(2*q6)*cos(q5))/64 + (3^(1/2)*ddqr2*sin(q2)*sin(q3)*sin(q4)*sin(q5))/16 - (3^(1/2)*ddqr3*sin(q2)*sin(q3)*sin(q4)*sin(q5))/16 - (9*dq1*dqr6*sin(2*q2)*sin(2*q3)*sin(2*q6)*cos(q5))/64 - (3*dq4*dqr6*sin(2*q6)*cos(q2)*cos(q3)*cos(q5))/16 - (3*dq5*dqr6*sin(2*q6)*cos(q2)*cos(q3)*cos(q5))/16 - (3*3^(1/2)*ddqr2*cos(2*q5)*cos(q4)*sin(q2)*sin(q3))/64 - (9*3^(1/2)*ddqr2*cos(2*q6)*cos(q4)*sin(q2)*sin(q3))/64 + (3*3^(1/2)*ddqr3*cos(2*q5)*cos(q4)*sin(q2)*sin(q3))/64 + (9*3^(1/2)*ddqr3*cos(2*q6)*cos(q4)*sin(q2)*sin(q3))/64 - (3*3^(1/2)*ddqr4*cos(2*q5)*cos(q3)*sin(q2)*sin(q4))/64 + (5*3^(1/2)*ddqr2*cos(2*q5)*cos(2*q6)*cos(q4)*sin(q2)*sin(q3))/64 - (5*3^(1/2)*ddqr3*cos(2*q5)*cos(2*q6)*cos(q4)*sin(q2)*sin(q3))/64 + (5*3^(1/2)*ddqr4*cos(2*q5)*cos(2*q6)*cos(q3)*sin(q2)*sin(q4))/64 + (25*dq1*dqr6*cos(2*q2)*cos(2*q3)*cos(2*q4)*cos(2*q5)*sin(2*q6))/256 + (5*dq1*dqr6*cos(2*q2)*cos(2*q3)*cos(2*q4)*cos(2*q6)*sin(2*q5))/64 + (dq1*dqr6*cos(2*q2)*cos(2*q3)*cos(2*q5)*cos(2*q6)*sin(2*q4))/16 - (3^(1/2)*ddqr2*cos(2*q5)*sin(2*q6)*sin(q2)*sin(q3)*sin(q4))/8 - (5*3^(1/2)*ddqr2*cos(2*q6)*sin(2*q5)*sin(q2)*sin(q3)*sin(q4))/32 - (3^(1/2)*ddqr2*sin(2*q5)*sin(2*q6)*cos(q4)*sin(q2)*sin(q3))/16 + (3^(1/2)*ddqr3*cos(2*q5)*sin(2*q6)*sin(q2)*sin(q3)*sin(q4))/8 + (5*3^(1/2)*ddqr3*cos(2*q6)*sin(2*q5)*sin(q2)*sin(q3)*sin(q4))/32 + (3^(1/2)*ddqr3*sin(2*q5)*sin(2*q6)*cos(q4)*sin(q2)*sin(q3))/16 - (3^(1/2)*ddqr4*sin(2*q5)*sin(2*q6)*cos(q3)*sin(q2)*sin(q4))/16 + (9*3^(1/2)*dq2*dqr6*sin(2*q6)*cos(q2)*cos(q3)*cos(q4))/64 - (9*3^(1/2)*dq3*dqr6*sin(2*q6)*cos(q2)*cos(q3)*cos(q4))/64 - (5*dq1*dqr6*cos(2*q2)*cos(2*q3)*sin(2*q4)*sin(2*q5)*sin(2*q6))/64 + (25*dq1*dqr6*cos(2*q4)*cos(2*q5)*sin(2*q2)*sin(2*q3)*sin(2*q6))/256 + (5*dq1*dqr6*cos(2*q4)*cos(2*q6)*sin(2*q2)*sin(2*q3)*sin(2*q5))/64 + (dq1*dqr6*cos(2*q5)*cos(2*q6)*sin(2*q2)*sin(2*q3)*sin(2*q4))/16 - (5*dq1*dqr6*sin(2*q2)*sin(2*q3)*sin(2*q4)*sin(2*q5)*sin(2*q6))/64 + (3^(1/2)*ddqr2*cos(2*q6)*cos(q4)*cos(q5)*sin(q2)*sin(q3))/16 - (3^(1/2)*ddqr3*cos(2*q6)*cos(q4)*cos(q5)*sin(q2)*sin(q3))/16 + (3^(1/2)*ddqr4*cos(2*q6)*cos(q3)*cos(q5)*sin(q2)*sin(q4))/16 + (3*dq1*dqr6*cos(2*q2)*cos(2*q3)*cos(2*q4)*sin(2*q6)*cos(q5))/64 + (3*dq1*dqr6*cos(2*q2)*cos(2*q3)*cos(2*q6)*sin(2*q4)*cos(q5))/16 + (3^(1/2)*ddqr2*cos(2*q6)*sin(q2)*sin(q3)*sin(q4)*sin(q5))/16 - (3^(1/2)*ddqr2*sin(2*q6)*cos(q4)*sin(q2)*sin(q3)*sin(q5))/8 + (3^(1/2)*ddqr2*sin(2*q6)*cos(q5)*sin(q2)*sin(q3)*sin(q4))/8 - (3^(1/2)*ddqr3*cos(2*q6)*sin(q2)*sin(q3)*sin(q4)*sin(q5))/16 + (3^(1/2)*ddqr3*sin(2*q6)*cos(q4)*sin(q2)*sin(q3)*sin(q5))/8 - (3^(1/2)*ddqr3*sin(2*q6)*cos(q5)*sin(q2)*sin(q3)*sin(q4))/8 - (3^(1/2)*ddqr4*sin(2*q6)*cos(q3)*sin(q2)*sin(q4)*sin(q5))/8 + (3^(1/2)*ddqr5*sin(2*q6)*cos(q3)*sin(q2)*sin(q4)*sin(q5))/8 + (3*dq1*dqr6*cos(2*q4)*sin(2*q2)*sin(2*q3)*sin(2*q6)*cos(q5))/64 + (3*dq1*dqr6*cos(2*q6)*sin(2*q2)*sin(2*q3)*sin(2*q4)*cos(q5))/16 - (3^(1/2)*dq1*dqr6*cos(2*q2)*cos(2*q5)*cos(2*q6)*sin(2*q3)*cos(q4))/8 + (3^(1/2)*dq1*dqr6*cos(2*q3)*cos(2*q5)*cos(2*q6)*sin(2*q2)*cos(q4))/8 + (5*3^(1/2)*dq1*dqr6*cos(2*q2)*sin(2*q3)*sin(2*q5)*sin(2*q6)*cos(q4))/32 - (5*3^(1/2)*dq1*dqr6*cos(2*q3)*sin(2*q2)*sin(2*q5)*sin(2*q6)*cos(q4))/32 - (5*3^(1/2)*dq2*dqr6*cos(2*q5)*sin(2*q6)*cos(q2)*cos(q3)*cos(q4))/64 + (5*3^(1/2)*dq3*dqr6*cos(2*q5)*sin(2*q6)*cos(q2)*cos(q3)*cos(q4))/64 + (3^(1/2)*dq3*dqr6*cos(2*q6)*sin(2*q5)*cos(q2)*cos(q3)*cos(q4))/16 + (3^(1/2)*dq1*dqr6*cos(2*q2)*cos(2*q6)*sin(2*q3)*cos(q4)*cos(q5))/8 - (3^(1/2)*dq1*dqr6*cos(2*q3)*cos(2*q6)*sin(2*q2)*cos(q4)*cos(q5))/8;
Y1_20_19=(3*ddqr2*sin(2*q4)*cos(q2)*sin(q3))/128 - (3*ddqr2*sin(2*q4)*cos(q3)*sin(q2))/128 - (3*ddqr3*sin(2*q4)*cos(q2)*sin(q3))/128 + (3*ddqr3*sin(2*q4)*cos(q3)*sin(q2))/128 + (3*ddqr2*cos(2*q4)*cos(q2)*sin(q3)*sin(q5))/16 - (3*ddqr2*cos(2*q4)*cos(q3)*sin(q2)*sin(q5))/16 + (3*ddqr2*sin(2*q4)*cos(q2)*cos(q5)*sin(q3))/32 - (3*ddqr2*sin(2*q4)*cos(q3)*cos(q5)*sin(q2))/32 - (3*ddqr3*cos(2*q4)*cos(q2)*sin(q3)*sin(q5))/16 + (3*ddqr3*cos(2*q4)*cos(q3)*sin(q2)*sin(q5))/16 - (3*ddqr3*sin(2*q4)*cos(q2)*cos(q5)*sin(q3))/32 + (3*ddqr3*sin(2*q4)*cos(q3)*cos(q5)*sin(q2))/32 + (3^(1/2)*ddqr4*cos(q2)*sin(q3)*sin(q4))/64 - (3^(1/2)*ddqr4*cos(q3)*sin(q2)*sin(q4))/64 - (5*3^(1/2)*ddqr5*cos(q2)*sin(q3)*sin(q4))/16 + (5*3^(1/2)*ddqr5*cos(q3)*sin(q2)*sin(q4))/16 - (3^(1/2)*ddqr6*cos(q2)*sin(q3)*sin(q4))/4 + (3^(1/2)*ddqr6*cos(q3)*sin(q2)*sin(q4))/4 - (3*ddqr2*cos(2*q4)*sin(2*q5)*cos(q2)*sin(q3))/32 + (3*ddqr2*cos(2*q4)*sin(2*q5)*cos(q3)*sin(q2))/32 - (15*ddqr2*cos(2*q5)*sin(2*q4)*cos(q2)*sin(q3))/128 + (15*ddqr2*cos(2*q5)*sin(2*q4)*cos(q3)*sin(q2))/128 + (27*ddqr2*cos(2*q6)*sin(2*q4)*cos(q2)*sin(q3))/128 - (27*ddqr2*cos(2*q6)*sin(2*q4)*cos(q3)*sin(q2))/128 + (3*ddqr3*cos(2*q4)*sin(2*q5)*cos(q2)*sin(q3))/32 - (3*ddqr3*cos(2*q4)*sin(2*q5)*cos(q3)*sin(q2))/32 + (15*ddqr3*cos(2*q5)*sin(2*q4)*cos(q2)*sin(q3))/128 - (15*ddqr3*cos(2*q5)*sin(2*q4)*cos(q3)*sin(q2))/128 - (27*ddqr3*cos(2*q6)*sin(2*q4)*cos(q2)*sin(q3))/128 + (27*ddqr3*cos(2*q6)*sin(2*q4)*cos(q3)*sin(q2))/128 + (ddqr2*cos(2*q4)*cos(2*q5)*sin(2*q6)*cos(q2)*sin(q3))/8 - (ddqr2*cos(2*q4)*cos(2*q5)*sin(2*q6)*cos(q3)*sin(q2))/8 + (5*ddqr2*cos(2*q4)*cos(2*q6)*sin(2*q5)*cos(q2)*sin(q3))/32 - (5*ddqr2*cos(2*q4)*cos(2*q6)*sin(2*q5)*cos(q3)*sin(q2))/32 + (25*ddqr2*cos(2*q5)*cos(2*q6)*sin(2*q4)*cos(q2)*sin(q3))/128 - (25*ddqr2*cos(2*q5)*cos(2*q6)*sin(2*q4)*cos(q3)*sin(q2))/128 - (ddqr3*cos(2*q4)*cos(2*q5)*sin(2*q6)*cos(q2)*sin(q3))/8 + (ddqr3*cos(2*q4)*cos(2*q5)*sin(2*q6)*cos(q3)*sin(q2))/8 - (5*ddqr3*cos(2*q4)*cos(2*q6)*sin(2*q5)*cos(q2)*sin(q3))/32 + (5*ddqr3*cos(2*q4)*cos(2*q6)*sin(2*q5)*cos(q3)*sin(q2))/32 - (25*ddqr3*cos(2*q5)*cos(2*q6)*sin(2*q4)*cos(q2)*sin(q3))/128 + (25*ddqr3*cos(2*q5)*cos(2*q6)*sin(2*q4)*cos(q3)*sin(q2))/128 - (5*ddqr2*sin(2*q4)*sin(2*q5)*sin(2*q6)*cos(q2)*sin(q3))/32 + (5*ddqr2*sin(2*q4)*sin(2*q5)*sin(2*q6)*cos(q3)*sin(q2))/32 + (5*ddqr3*sin(2*q4)*sin(2*q5)*sin(2*q6)*cos(q2)*sin(q3))/32 - (5*ddqr3*sin(2*q4)*sin(2*q5)*sin(2*q6)*cos(q3)*sin(q2))/32 + (3^(1/2)*ddqr4*cos(q2)*cos(q4)*sin(q3)*sin(q5))/16 - (3^(1/2)*ddqr4*cos(q2)*cos(q5)*sin(q3)*sin(q4))/16 - (3^(1/2)*ddqr4*cos(q3)*cos(q4)*sin(q2)*sin(q5))/16 + (3^(1/2)*ddqr5*cos(q2)*cos(q4)*sin(q3)*sin(q5))/8 + (3^(1/2)*ddqr5*cos(q2)*cos(q5)*sin(q3)*sin(q4))/16 - (3^(1/2)*ddqr5*cos(q3)*cos(q4)*sin(q2)*sin(q5))/8 - (3^(1/2)*ddqr5*cos(q3)*cos(q5)*sin(q2)*sin(q4))/16 + (3^(1/2)*ddqr6*cos(q2)*cos(q4)*sin(q3)*sin(q5))/2 + (3^(1/2)*ddqr6*cos(q2)*cos(q5)*sin(q3)*sin(q4))/4 - (3^(1/2)*ddqr6*cos(q3)*cos(q4)*sin(q2)*sin(q5))/2 - (3^(1/2)*ddqr6*cos(q3)*cos(q5)*sin(q2)*sin(q4))/4 + (3*ddqr2*cos(2*q4)*cos(2*q6)*cos(q2)*sin(q3)*sin(q5))/16 - (3*ddqr2*cos(2*q4)*cos(2*q6)*cos(q3)*sin(q2)*sin(q5))/16 + (3*ddqr2*cos(2*q4)*sin(2*q6)*cos(q2)*cos(q5)*sin(q3))/8 - (3*ddqr2*cos(2*q4)*sin(2*q6)*cos(q3)*cos(q5)*sin(q2))/8 + (3*ddqr2*cos(2*q6)*sin(2*q4)*cos(q2)*cos(q5)*sin(q3))/32 - (3*ddqr2*cos(2*q6)*sin(2*q4)*cos(q3)*cos(q5)*sin(q2))/32 - (3*ddqr3*cos(2*q4)*cos(2*q6)*cos(q2)*sin(q3)*sin(q5))/16 + (3*ddqr3*cos(2*q4)*cos(2*q6)*cos(q3)*sin(q2)*sin(q5))/16 - (3*ddqr3*cos(2*q4)*sin(2*q6)*cos(q2)*cos(q5)*sin(q3))/8 + (3*ddqr3*cos(2*q4)*sin(2*q6)*cos(q3)*cos(q5)*sin(q2))/8 - (3*ddqr3*cos(2*q6)*sin(2*q4)*cos(q2)*cos(q5)*sin(q3))/32 + (3*ddqr3*cos(2*q6)*sin(2*q4)*cos(q3)*cos(q5)*sin(q2))/32 - (3*ddqr2*sin(2*q4)*sin(2*q6)*cos(q2)*sin(q3)*sin(q5))/16 + (3*ddqr2*sin(2*q4)*sin(2*q6)*cos(q3)*sin(q2)*sin(q5))/16 + (3*ddqr3*sin(2*q4)*sin(2*q6)*cos(q2)*sin(q3)*sin(q5))/16 - (3*ddqr3*sin(2*q4)*sin(2*q6)*cos(q3)*sin(q2)*sin(q5))/16 + (3*3^(1/2)*ddqr4*cos(2*q5)*cos(q2)*sin(q3)*sin(q4))/64 + (3*3^(1/2)*ddqr4*sin(2*q5)*cos(q2)*cos(q4)*sin(q3))/32 - (3*3^(1/2)*ddqr4*sin(2*q5)*cos(q3)*cos(q4)*sin(q2))/32 + (9*3^(1/2)*ddqr4*cos(2*q6)*cos(q2)*sin(q3)*sin(q4))/64 - (9*3^(1/2)*ddqr4*cos(2*q6)*cos(q3)*sin(q2)*sin(q4))/64 + (3*3^(1/2)*ddqr5*cos(2*q6)*cos(q2)*sin(q3)*sin(q4))/16 - (3*3^(1/2)*ddqr5*cos(2*q6)*cos(q3)*sin(q2)*sin(q4))/16 - (5*3^(1/2)*ddqr4*cos(2*q5)*cos(2*q6)*cos(q2)*sin(q3)*sin(q4))/64 - (3^(1/2)*ddqr4*cos(2*q5)*sin(2*q6)*cos(q2)*cos(q4)*sin(q3))/8 + (3^(1/2)*ddqr4*cos(2*q5)*sin(2*q6)*cos(q3)*cos(q4)*sin(q2))/8 - (5*3^(1/2)*ddqr4*cos(2*q6)*sin(2*q5)*cos(q2)*cos(q4)*sin(q3))/32 + (5*3^(1/2)*ddqr4*cos(2*q6)*sin(2*q5)*cos(q3)*cos(q4)*sin(q2))/32 + (3^(1/2)*ddqr4*sin(2*q5)*sin(2*q6)*cos(q2)*sin(q3)*sin(q4))/16 - (3^(1/2)*ddqr1*cos(2*q3)*sin(2*q2)*sin(2*q6)*sin(q4)*sin(q5))/8 + (3^(1/2)*ddqr4*cos(2*q6)*cos(q2)*cos(q4)*sin(q3)*sin(q5))/16 - (3^(1/2)*ddqr4*cos(2*q6)*cos(q2)*cos(q5)*sin(q3)*sin(q4))/16 - (3^(1/2)*ddqr4*cos(2*q6)*cos(q3)*cos(q4)*sin(q2)*sin(q5))/16 + (3^(1/2)*ddqr4*sin(2*q6)*cos(q2)*cos(q4)*cos(q5)*sin(q3))/8 - (3^(1/2)*ddqr4*sin(2*q6)*cos(q3)*cos(q4)*cos(q5)*sin(q2))/8 + (3^(1/2)*ddqr5*cos(2*q6)*cos(q2)*cos(q4)*sin(q3)*sin(q5))/8 + (3^(1/2)*ddqr5*cos(2*q6)*cos(q2)*cos(q5)*sin(q3)*sin(q4))/16 - (3^(1/2)*ddqr5*cos(2*q6)*cos(q3)*cos(q4)*sin(q2)*sin(q5))/8 - (3^(1/2)*ddqr5*cos(2*q6)*cos(q3)*cos(q5)*sin(q2)*sin(q4))/16 + (3^(1/2)*ddqr5*sin(2*q6)*cos(q2)*cos(q4)*cos(q5)*sin(q3))/4 - (3^(1/2)*ddqr5*sin(2*q6)*cos(q3)*cos(q4)*cos(q5)*sin(q2))/4 + (3^(1/2)*ddqr4*sin(2*q6)*cos(q2)*sin(q3)*sin(q4)*sin(q5))/8 - (3^(1/2)*ddqr5*sin(2*q6)*cos(q2)*sin(q3)*sin(q4)*sin(q5))/8;
Y1_20_20=(3*ddqr1*cos(q5))/64 + (ddqr1*sin(2*q2)*sin(2*q3))/256 + (3*ddqr1*sin(2*q4)*sin(2*q5))/64 + (3*ddqr1*sin(2*q5)*sin(2*q6))/64 + (3*ddqr1*cos(2*q4)*cos(q5))/64 + (3*ddqr1*cos(2*q6)*cos(q5))/64 - (3*ddqr1*sin(2*q4)*sin(q5))/32 - (3*ddqr1*sin(2*q6)*sin(q5))/32 + (9*ddqr1*sin(2*q2)*sin(2*q3)*cos(q5))/64 - (3*ddqr1*cos(2*q4)*sin(2*q6)*sin(q5))/32 - (3*ddqr1*cos(2*q6)*sin(2*q4)*sin(q5))/32 - (3*ddqr1*sin(2*q4)*sin(2*q6)*cos(q5))/16 - (3*ddqr1*cos(2*q2)*cos(2*q3)*cos(2*q4))/256 + (27*ddqr1*cos(2*q2)*cos(2*q3)*cos(2*q5))/256 + (9*ddqr1*cos(2*q2)*cos(2*q3)*cos(2*q6))/256 - (3*ddqr1*cos(2*q4)*sin(2*q2)*sin(2*q3))/256 + (27*ddqr1*cos(2*q5)*sin(2*q2)*sin(2*q3))/256 + (9*ddqr1*cos(2*q6)*sin(2*q2)*sin(2*q3))/256 - (5*ddqr1*cos(2*q4)*sin(2*q5)*sin(2*q6))/64 - (ddqr1*cos(2*q5)*sin(2*q4)*sin(2*q6))/16 - (5*ddqr1*cos(2*q6)*sin(2*q4)*sin(2*q5))/64 + (9*ddqr1*cos(2*q2)*cos(2*q3)*cos(q5))/64 + (3*ddqr1*cos(2*q4)*cos(2*q6)*cos(q5))/64 - (3*ddqr1*cos(2*q2)*cos(2*q3)*cos(2*q4)*cos(q5))/64 + (9*ddqr1*cos(2*q2)*cos(2*q3)*cos(2*q6)*cos(q5))/64 + (3*ddqr1*cos(2*q2)*cos(2*q3)*sin(2*q4)*sin(q5))/32 - (3*ddqr1*cos(2*q4)*sin(2*q2)*sin(2*q3)*cos(q5))/64 - (9*ddqr1*cos(2*q2)*cos(2*q3)*sin(2*q6)*sin(q5))/32 + (9*ddqr1*cos(2*q6)*sin(2*q2)*sin(2*q3)*cos(q5))/64 + (3*ddqr1*sin(2*q2)*sin(2*q3)*sin(2*q4)*sin(q5))/32 - (9*ddqr1*sin(2*q2)*sin(2*q3)*sin(2*q6)*sin(q5))/32 + (3^(1/2)*ddqr1*cos(2*q2)*sin(2*q3)*sin(q4))/64 - (3^(1/2)*ddqr1*cos(2*q3)*sin(2*q2)*sin(q4))/64 + (15*ddqr1*cos(2*q2)*cos(2*q3)*cos(2*q4)*cos(2*q5))/256 - (27*ddqr1*cos(2*q2)*cos(2*q3)*cos(2*q4)*cos(2*q6))/256 - (45*ddqr1*cos(2*q2)*cos(2*q3)*cos(2*q5)*cos(2*q6))/256 - (3*ddqr4*sin(2*q6)*cos(q2)*cos(q3)*sin(q5))/8 - (3*ddqr5*sin(2*q6)*cos(q2)*cos(q3)*sin(q5))/8 - (3*ddqr1*cos(2*q2)*cos(2*q3)*sin(2*q4)*sin(2*q5))/64 + (15*ddqr1*cos(2*q4)*cos(2*q5)*sin(2*q2)*sin(2*q3))/256 - (27*ddqr1*cos(2*q4)*cos(2*q6)*sin(2*q2)*sin(2*q3))/256 + (9*ddqr1*cos(2*q2)*cos(2*q3)*sin(2*q5)*sin(2*q6))/64 - (45*ddqr1*cos(2*q5)*cos(2*q6)*sin(2*q2)*sin(2*q3))/256 - (3*ddqr1*sin(2*q2)*sin(2*q3)*sin(2*q4)*sin(2*q5))/64 + (9*ddqr1*sin(2*q2)*sin(2*q3)*sin(2*q5)*sin(2*q6))/64 + (5*ddqr1*cos(2*q4)*sin(2*q2)*sin(2*q3)*sin(2*q5)*sin(2*q6))/64 + (ddqr1*cos(2*q5)*sin(2*q2)*sin(2*q3)*sin(2*q4)*sin(2*q6))/16 + (5*ddqr1*cos(2*q6)*sin(2*q2)*sin(2*q3)*sin(2*q4)*sin(2*q5))/64 + (3^(1/2)*ddqr1*cos(2*q2)*sin(2*q3)*cos(q4)*sin(q5))/16 - (3^(1/2)*ddqr1*cos(2*q2)*sin(2*q3)*cos(q5)*sin(q4))/16 - (3^(1/2)*ddqr1*cos(2*q3)*sin(2*q2)*cos(q4)*sin(q5))/16 + (3^(1/2)*ddqr1*cos(2*q3)*sin(2*q2)*cos(q5)*sin(q4))/16 - (3*ddqr1*cos(2*q2)*cos(2*q3)*cos(2*q4)*cos(2*q6)*cos(q5))/64 + (3*ddqr1*cos(2*q2)*cos(2*q3)*cos(2*q4)*sin(2*q6)*sin(q5))/32 + (3*ddqr1*cos(2*q2)*cos(2*q3)*cos(2*q6)*sin(2*q4)*sin(q5))/32 + (3*ddqr1*cos(2*q2)*cos(2*q3)*sin(2*q4)*sin(2*q6)*cos(q5))/16 - (3*ddqr1*cos(2*q4)*cos(2*q6)*sin(2*q2)*sin(2*q3)*cos(q5))/64 + (3^(1/2)*ddqr2*cos(q2)*cos(q3)*sin(q4)*sin(q5))/16 - (3^(1/2)*ddqr3*cos(q2)*cos(q3)*sin(q4)*sin(q5))/16 + (3*ddqr1*cos(2*q4)*sin(2*q2)*sin(2*q3)*sin(2*q6)*sin(q5))/32 + (3*ddqr1*cos(2*q6)*sin(2*q2)*sin(2*q3)*sin(2*q4)*sin(q5))/32 + (3*ddqr1*sin(2*q2)*sin(2*q3)*sin(2*q4)*sin(2*q6)*cos(q5))/16 + (3*3^(1/2)*ddqr1*cos(2*q2)*cos(2*q5)*sin(2*q3)*sin(q4))/64 + (3*3^(1/2)*ddqr1*cos(2*q2)*sin(2*q3)*sin(2*q5)*cos(q4))/32 - (3*3^(1/2)*ddqr1*cos(2*q3)*cos(2*q5)*sin(2*q2)*sin(q4))/64 - (3*3^(1/2)*ddqr1*cos(2*q3)*sin(2*q2)*sin(2*q5)*cos(q4))/32 + (9*3^(1/2)*ddqr1*cos(2*q2)*cos(2*q6)*sin(2*q3)*sin(q4))/64 - (9*3^(1/2)*ddqr1*cos(2*q3)*cos(2*q6)*sin(2*q2)*sin(q4))/64 - (25*ddqr1*cos(2*q2)*cos(2*q3)*cos(2*q4)*cos(2*q5)*cos(2*q6))/256 + (5*ddqr1*cos(2*q2)*cos(2*q3)*cos(2*q4)*sin(2*q5)*sin(2*q6))/64 + (ddqr1*cos(2*q2)*cos(2*q3)*cos(2*q5)*sin(2*q4)*sin(2*q6))/16 + (5*ddqr1*cos(2*q2)*cos(2*q3)*cos(2*q6)*sin(2*q4)*sin(2*q5))/64 - (25*ddqr1*cos(2*q4)*cos(2*q5)*cos(2*q6)*sin(2*q2)*sin(2*q3))/256 + (3*3^(1/2)*ddqr2*sin(2*q5)*cos(q2)*cos(q3)*sin(q4))/32 - (3*3^(1/2)*ddqr3*sin(2*q5)*cos(q2)*cos(q3)*sin(q4))/32 + (3^(1/2)*ddqr1*cos(2*q2)*sin(2*q3)*sin(2*q5)*sin(2*q6)*sin(q4))/16 - (3^(1/2)*ddqr1*cos(2*q3)*sin(2*q2)*sin(2*q5)*sin(2*q6)*sin(q4))/16 - (3^(1/2)*ddqr2*cos(2*q5)*sin(2*q6)*cos(q2)*cos(q3)*sin(q4))/8 - (5*3^(1/2)*ddqr2*cos(2*q6)*sin(2*q5)*cos(q2)*cos(q3)*sin(q4))/32 + (3^(1/2)*ddqr3*cos(2*q5)*sin(2*q6)*cos(q2)*cos(q3)*sin(q4))/8 + (5*3^(1/2)*ddqr3*cos(2*q6)*sin(2*q5)*cos(q2)*cos(q3)*sin(q4))/32 + (3^(1/2)*ddqr1*cos(2*q2)*cos(2*q6)*sin(2*q3)*cos(q4)*sin(q5))/16 - (3^(1/2)*ddqr1*cos(2*q2)*cos(2*q6)*sin(2*q3)*cos(q5)*sin(q4))/16 + (3^(1/2)*ddqr1*cos(2*q2)*sin(2*q3)*sin(2*q6)*cos(q4)*cos(q5))/8 - (3^(1/2)*ddqr1*cos(2*q3)*cos(2*q6)*sin(2*q2)*cos(q4)*sin(q5))/16 + (3^(1/2)*ddqr1*cos(2*q3)*cos(2*q6)*sin(2*q2)*cos(q5)*sin(q4))/16 - (3^(1/2)*ddqr1*cos(2*q3)*sin(2*q2)*sin(2*q6)*cos(q4)*cos(q5))/8 + (3^(1/2)*ddqr1*cos(2*q2)*sin(2*q3)*sin(2*q6)*sin(q4)*sin(q5))/8 + (3^(1/2)*ddqr2*cos(2*q6)*cos(q2)*cos(q3)*sin(q4)*sin(q5))/16 - (3^(1/2)*ddqr2*sin(2*q6)*cos(q2)*cos(q3)*cos(q4)*sin(q5))/8 + (3^(1/2)*ddqr2*sin(2*q6)*cos(q2)*cos(q3)*cos(q5)*sin(q4))/8 - (3^(1/2)*ddqr3*cos(2*q6)*cos(q2)*cos(q3)*sin(q4)*sin(q5))/16 + (3^(1/2)*ddqr3*sin(2*q6)*cos(q2)*cos(q3)*cos(q4)*sin(q5))/8 - (3^(1/2)*ddqr3*sin(2*q6)*cos(q2)*cos(q3)*cos(q5)*sin(q4))/8 - (5*3^(1/2)*ddqr1*cos(2*q2)*cos(2*q5)*cos(2*q6)*sin(2*q3)*sin(q4))/64 - (3^(1/2)*ddqr1*cos(2*q2)*cos(2*q5)*sin(2*q3)*sin(2*q6)*cos(q4))/8 - (5*3^(1/2)*ddqr1*cos(2*q2)*cos(2*q6)*sin(2*q3)*sin(2*q5)*cos(q4))/32 + (5*3^(1/2)*ddqr1*cos(2*q3)*cos(2*q5)*cos(2*q6)*sin(2*q2)*sin(q4))/64 + (3^(1/2)*ddqr1*cos(2*q3)*cos(2*q5)*sin(2*q2)*sin(2*q6)*cos(q4))/8 + (5*3^(1/2)*ddqr1*cos(2*q3)*cos(2*q6)*sin(2*q2)*sin(2*q5)*cos(q4))/32;
Y1_20_21=(171*ddqr1)/256 + (3*ddqr1*cos(2*q4))/256 + (9*ddqr1*cos(2*q5))/256 + (3*ddqr1*cos(2*q6))/256 + (ddqr1*cos(2*q2)*cos(2*q3))/256 - (15*ddqr1*cos(2*q4)*cos(2*q5))/256 + (27*ddqr1*cos(2*q4)*cos(2*q6))/256 - (15*ddqr1*cos(2*q5)*cos(2*q6))/256 + (43*ddqr4*cos(q2)*cos(q3))/64 + (5*ddqr5*cos(q2)*cos(q3))/16 + (ddqr6*cos(q2)*cos(q3))/4 + (3*ddqr4*cos(q2)*cos(q3)*cos(q5))/16 + (3*ddqr5*cos(q2)*cos(q3)*cos(q5))/16 + (3*ddqr6*cos(q2)*cos(q3)*cos(q5))/4 + (25*ddqr1*cos(2*q4)*cos(2*q5)*cos(2*q6))/256 + (9*ddqr4*cos(2*q5)*cos(q2)*cos(q3))/64 + (3*ddqr4*cos(2*q6)*cos(q2)*cos(q3))/64 - (3*ddqr5*cos(2*q6)*cos(q2)*cos(q3))/16 + (3*ddqr4*cos(2*q6)*cos(q2)*cos(q3)*cos(q5))/16 + (3*ddqr5*cos(2*q6)*cos(q2)*cos(q3)*cos(q5))/16 - (3^(1/2)*ddqr2*cos(q2)*cos(q3)*cos(q4))/64 + (3^(1/2)*ddqr3*cos(q2)*cos(q3)*cos(q4))/64 - (15*ddqr4*cos(2*q5)*cos(2*q6)*cos(q2)*cos(q3))/64 + (3*ddqr4*sin(2*q5)*sin(2*q6)*cos(q2)*cos(q3))/16 + (3^(1/2)*ddqr2*cos(q2)*cos(q3)*cos(q4)*cos(q5))/16 - (3^(1/2)*ddqr3*cos(q2)*cos(q3)*cos(q4)*cos(q5))/16 - (3*3^(1/2)*ddqr2*cos(2*q5)*cos(q2)*cos(q3)*cos(q4))/64 - (9*3^(1/2)*ddqr2*cos(2*q6)*cos(q2)*cos(q3)*cos(q4))/64 + (3*3^(1/2)*ddqr3*cos(2*q5)*cos(q2)*cos(q3)*cos(q4))/64 + (9*3^(1/2)*ddqr3*cos(2*q6)*cos(q2)*cos(q3)*cos(q4))/64 + (5*3^(1/2)*ddqr2*cos(2*q5)*cos(2*q6)*cos(q2)*cos(q3)*cos(q4))/64 - (5*3^(1/2)*ddqr3*cos(2*q5)*cos(2*q6)*cos(q2)*cos(q3)*cos(q4))/64 - (3^(1/2)*ddqr2*sin(2*q5)*sin(2*q6)*cos(q2)*cos(q3)*cos(q4))/16 + (3^(1/2)*ddqr3*sin(2*q5)*sin(2*q6)*cos(q2)*cos(q3)*cos(q4))/16 + (3^(1/2)*ddqr2*cos(2*q6)*cos(q2)*cos(q3)*cos(q4)*cos(q5))/16 - (3^(1/2)*ddqr3*cos(2*q6)*cos(q2)*cos(q3)*cos(q4)*cos(q5))/16;
Y2_2_1=(841*ddqr2)/10000 + (29*ddqr1*cos(q2))/62500 - (841*dq1*dqr1*sin(2*q2))/20000;
Y2_3_1=(9925361*ddqr2)/100000000 - (1515361*ddqr3)/100000000 - (203*ddqr1*cos(q2))/100000 - (35699*ddqr2*cos(q3))/500000 + (35699*ddqr3*cos(q3))/1000000 + (35699*dq1*dqr1*sin(q3))/1000000 + (35699*dq2*dqr3*sin(q3))/1000000 + (35699*dq3*dqr2*sin(q3))/1000000 - (35699*dq3*dqr3*sin(q3))/1000000 - (6894639*dq1*dqr1*sin(2*q2))/200000000 - (1515361*dq1*dqr1*sin(2*q3))/200000000 + (8617*ddqr1*cos(q2)*cos(q3))/10000000 + (8617*ddqr1*sin(q2)*sin(q3))/10000000 - (35699*dq1*dqr1*cos(q2)^2*sin(q3))/500000 - (1515361*dq1*dqr1*cos(q2)*cos(q3)^2*sin(q2))/50000000 + (1515361*dq1*dqr1*cos(q2)^2*cos(q3)*sin(q3))/50000000 + (35699*dq1*dqr1*cos(q2)*cos(q3)*sin(q2))/500000;
Y2_4_1=(3012821*ddqr2)/25000000 - (910321*ddqr3)/25000000 - (203*ddqr1*cos(q2))/100000 - (3393*ddqr2*cos(q3))/31250 + (3393*ddqr3*cos(q3))/62500 - (4329*ddqr4*cos(q4))/625000 - (1369*ddqr2*cos(q4)^2)/1000000 + (1369*ddqr3*cos(q4)^2)/1000000 + (3393*dq1*dqr1*sin(q3))/62500 + (4329*dq1*dqr1*sin(q4))/625000 + (3393*dq2*dqr3*sin(q3))/62500 + (3393*dq3*dqr2*sin(q3))/62500 - (3393*dq3*dqr3*sin(q3))/62500 + (4329*dq4*dqr4*sin(q4))/625000 - (1260629*dq1*dqr1*sin(2*q2))/50000000 - (841871*dq1*dqr1*sin(2*q3))/50000000 + (1369*dq2*dqr4*sin(2*q4))/2000000 + (1369*dq4*dqr2*sin(2*q4))/2000000 - (1369*dq3*dqr4*sin(2*q4))/2000000 - (1369*dq4*dqr3*sin(2*q4))/2000000 + (819*ddqr1*cos(q2)*cos(q3))/625000 + (1073*ddqr1*cos(q2)*cos(q4))/100000 + (1073*ddqr4*cos(q3)*cos(q4))/100000 + (819*ddqr1*sin(q2)*sin(q3))/625000 + (1073*ddqr2*sin(q3)*sin(q4))/50000 - (1073*ddqr3*sin(q3)*sin(q4))/100000 - (3393*dq1*dqr1*cos(q2)^2*sin(q3))/31250 - (4329*dq1*dqr1*cos(q2)^2*sin(q4))/312500 - (4329*dq1*dqr1*cos(q3)^2*sin(q4))/312500 - (4329*ddqr1*cos(q2)*cos(q3)*cos(q4))/625000 - (259*ddqr1*cos(q2)*sin(q3)*sin(q4))/1000000 + (259*ddqr1*cos(q3)*sin(q2)*sin(q4))/1000000 - (4329*ddqr1*cos(q4)*sin(q2)*sin(q3))/625000 + (1073*dq1*dqr1*cos(q3)*sin(q4))/100000 - (1369*dq1*dqr4*cos(q2)*sin(q3))/1000000 + (1369*dq1*dqr4*cos(q3)*sin(q2))/1000000 - (1369*dq4*dqr1*cos(q2)*sin(q3))/1000000 + (1369*dq4*dqr1*cos(q3)*sin(q2))/1000000 - (1073*dq1*dqr4*cos(q2)*sin(q4))/100000 - (1073*dq4*dqr1*cos(q2)*sin(q4))/100000 + (1073*dq2*dqr3*cos(q3)*sin(q4))/100000 + (1073*dq3*dqr2*cos(q3)*sin(q4))/100000 + (1073*dq2*dqr4*cos(q4)*sin(q3))/100000 - (1073*dq3*dqr3*cos(q3)*sin(q4))/100000 + (1073*dq4*dqr2*cos(q4)*sin(q3))/100000 - (1073*dq3*dqr4*cos(q4)*sin(q3))/100000 - (1073*dq4*dqr3*cos(q4)*sin(q3))/100000 - (1073*dq4*dqr4*cos(q3)*sin(q4))/100000 - (841871*dq1*dqr1*cos(q2)*cos(q3)^2*sin(q2))/12500000 + (1369*dq1*dqr1*cos(q2)*cos(q4)^2*sin(q2))/1000000 + (841871*dq1*dqr1*cos(q2)^2*cos(q3)*sin(q3))/12500000 - (1073*dq1*dqr1*cos(q2)^2*cos(q3)*sin(q4))/50000 - (1369*dq1*dqr1*cos(q3)*cos(q4)^2*sin(q3))/1000000 + (1369*dq1*dqr4*cos(q2)*cos(q4)^2*sin(q3))/1000000 - (1369*dq1*dqr4*cos(q3)*cos(q4)^2*sin(q2))/1000000 + (1369*dq4*dqr1*cos(q2)*cos(q4)^2*sin(q3))/1000000 - (1369*dq4*dqr1*cos(q3)*cos(q4)^2*sin(q2))/1000000 + (1369*ddqr1*cos(q2)*cos(q4)*sin(q3)*sin(q4))/1000000 - (1369*ddqr1*cos(q3)*cos(q4)*sin(q2)*sin(q4))/1000000 + (4329*dq1*dqr1*cos(q2)^2*cos(q3)^2*sin(q4))/156250 + (3393*dq1*dqr1*cos(q2)*cos(q3)*sin(q2))/31250 + (4329*dq1*dqr4*cos(q2)*cos(q3)*sin(q4))/625000 + (4329*dq4*dqr1*cos(q2)*cos(q3)*sin(q4))/625000 + (4329*dq1*dqr4*sin(q2)*sin(q3)*sin(q4))/625000 + (4329*dq4*dqr1*sin(q2)*sin(q3)*sin(q4))/625000 - (1369*dq1*dqr1*cos(q2)*cos(q3)^2*cos(q4)^2*sin(q2))/500000 + (1369*dq1*dqr1*cos(q2)^2*cos(q3)*cos(q4)^2*sin(q3))/500000 - (1073*dq1*dqr1*cos(q2)*sin(q2)*sin(q3)*sin(q4))/50000 + (4329*dq1*dqr1*cos(q2)*cos(q3)*sin(q2)*sin(q3)*sin(q4))/156250;
Y2_5_1=(25433*dq1*dqr1*sin(q3))/400000 - (25433*dq1*dqr1*cos(q2)^2*sin(q3))/200000 + (1369*dq1*dqr1*cos(q2)*cos(q5)^2*sin(q2))/2000000 - (1369*dq1*dqr1*cos(q3)*cos(q5)^2*sin(q3))/2000000 - (1369*dq4*dqr1*cos(q2)*cos(q5)^2*sin(q3))/4000000 + (1369*dq4*dqr1*cos(q3)*cos(q5)^2*sin(q2))/4000000 - (1369*dq5*dqr1*cos(q2)*cos(q4)^2*sin(q3))/2000000 + (1369*dq5*dqr1*cos(q3)*cos(q4)^2*sin(q2))/2000000 - (1369*dq5*dqr1*cos(q2)*cos(q5)^2*sin(q3))/2000000 + (1369*dq5*dqr1*cos(q3)*cos(q5)^2*sin(q2))/2000000 - dq4*dqr1*cos(q2)*sin(q3)*((23717*3^(1/2))/10000000 + 1780243/400000000) + dq4*dqr1*cos(q3)*sin(q2)*((23717*3^(1/2))/10000000 + 1780243/400000000) + (1073*3^(1/2)*dq1*dqr1*cos(q5)*sin(q3))/200000 - dq1*dqr1*cos(q2)^2*sin(q4)*((562157*3^(1/2))/40000000 + 32449/2000000) + (25433*dq1*dqr1*cos(q2)*cos(q3)*sin(q2))/200000 + (1073*dq4*dqr1*cos(q2)*cos(q5)*sin(q4))/200000 + (1073*dq5*dqr1*cos(q2)*cos(q5)*sin(q4))/100000 - dq4*dqr1*cos(q2)*sin(q4)*((18589*3^(1/2))/2000000 + 1073/100000) - dq1*dqr1*cos(q2)^2*cos(q3)*sin(q4)*((18589*3^(1/2))/1000000 + 1073/50000) - dq1*dqr1*cos(q2)^2*cos(q5)*sin(q4)*((1369*3^(1/2))/1000000 - 45547/10000000) + dq1*dqr1*cos(q2)*cos(q3)^2*sin(q2)*((23717*3^(1/2))/5000000 - 8723991/100000000) - dq1*dqr1*cos(q2)^2*cos(q3)*sin(q3)*((23717*3^(1/2))/5000000 - 8723991/100000000) - (1369*dq1*dqr1*cos(q2)*cos(q3)^2*cos(q5)^2*sin(q2))/1000000 + (1369*dq1*dqr1*cos(q2)*cos(q4)^2*cos(q5)^2*sin(q2))/800000 + (1369*dq1*dqr1*cos(q2)^2*cos(q3)*cos(q5)^2*sin(q3))/1000000 - (1369*dq1*dqr1*cos(q3)*cos(q4)^2*cos(q5)^2*sin(q3))/800000 + (1369*dq4*dqr1*cos(q2)*cos(q4)^2*cos(q5)^2*sin(q3))/800000 - (1369*dq4*dqr1*cos(q3)*cos(q4)^2*cos(q5)^2*sin(q2))/800000 + (1369*dq5*dqr1*cos(q2)*cos(q4)^2*cos(q5)^2*sin(q3))/1000000 - (1369*dq5*dqr1*cos(q3)*cos(q4)^2*cos(q5)^2*sin(q2))/1000000 + dq1*dqr1*cos(q2)*cos(q4)^2*sin(q2)*((23717*3^(1/2))/10000000 + 1232643/400000000) - dq1*dqr1*cos(q3)*cos(q4)^2*sin(q3)*((23717*3^(1/2))/10000000 + 1232643/400000000) + dq4*dqr1*cos(q2)*cos(q4)^2*sin(q3)*((23717*3^(1/2))/10000000 + 1232643/400000000) - dq4*dqr1*cos(q3)*cos(q4)^2*sin(q2)*((23717*3^(1/2))/10000000 + 1232643/400000000) - (1073*3^(1/2)*dq1*dqr1*cos(q2)^2*cos(q5)*sin(q3))/100000 - (32449*dq5*dqr1*cos(q2)*cos(q3)*cos(q5)*sin(q4))/4000000 + dq1*dqr1*cos(q2)^2*cos(q3)^2*sin(q4)*((562157*3^(1/2))/20000000 + 32449/1000000) - (32449*dq4*dqr1*cos(q4)*sin(q2)*sin(q3)*sin(q5))/4000000 - (32449*dq5*dqr1*cos(q4)*sin(q2)*sin(q3)*sin(q5))/8000000 - (32449*dq5*dqr1*cos(q5)*sin(q2)*sin(q3)*sin(q4))/4000000 + (1369*3^(1/2)*dq1*dqr1*cos(q2)^2*cos(q5)^2*sin(q4))/2000000 + (1369*3^(1/2)*dq1*dqr1*cos(q3)^2*cos(q5)^2*sin(q4))/2000000 + dq1*dqr1*cos(q2)*cos(q5)*sin(q2)*((92981*3^(1/2))/10000000 + 1369/1000000) - dq1*dqr1*cos(q3)*cos(q5)*sin(q3)*((92981*3^(1/2))/10000000 + 1369/1000000) + dq4*dqr1*cos(q2)*cos(q5)*sin(q3)*((23717*3^(1/2))/20000000 + 1369/1000000) - dq4*dqr1*cos(q3)*cos(q5)*sin(q2)*((23717*3^(1/2))/20000000 + 1369/1000000) + dq5*dqr1*cos(q2)*cos(q5)*sin(q3)*((23717*3^(1/2))/20000000 + 1369/1000000) - dq5*dqr1*cos(q3)*cos(q5)*sin(q2)*((23717*3^(1/2))/20000000 + 1369/1000000) + dq4*dqr1*cos(q2)*cos(q3)*sin(q4)*((562157*3^(1/2))/80000000 + 32449/4000000) + (1073*dq1*dqr1*cos(q2)^2*cos(q3)*cos(q5)*sin(q4))/100000 + dq4*dqr1*sin(q2)*sin(q3)*sin(q4)*((562157*3^(1/2))/80000000 + 32449/4000000) - (1369*3^(1/2)*dq1*dqr1*cos(q2)^2*cos(q3)^2*cos(q5)^2*sin(q4))/1000000 - dq1*dqr1*cos(q2)*cos(q3)^2*cos(q5)*sin(q2)*((92981*3^(1/2))/5000000 + 1369/500000) + dq1*dqr1*cos(q2)^2*cos(q3)*cos(q5)*sin(q3)*((92981*3^(1/2))/5000000 + 1369/500000) - dq1*dqr1*cos(q2)*cos(q4)^2*cos(q5)*sin(q2)*((23717*3^(1/2))/20000000 + 1369/1000000) + dq1*dqr1*cos(q3)*cos(q4)^2*cos(q5)*sin(q3)*((23717*3^(1/2))/20000000 + 1369/1000000) - dq4*dqr1*cos(q2)*cos(q4)^2*cos(q5)*sin(q3)*((23717*3^(1/2))/20000000 + 1369/1000000) + dq4*dqr1*cos(q3)*cos(q4)^2*cos(q5)*sin(q2)*((23717*3^(1/2))/20000000 + 1369/1000000) - dq5*dqr1*cos(q2)*cos(q4)^2*cos(q5)*sin(q3)*((23717*3^(1/2))/20000000 + 1369/1000000) + dq5*dqr1*cos(q3)*cos(q4)^2*cos(q5)*sin(q2)*((23717*3^(1/2))/20000000 + 1369/1000000) - (1369*3^(1/2)*dq4*dqr1*cos(q2)*cos(q3)*cos(q5)^2*sin(q4))/4000000 - (1369*3^(1/2)*dq5*dqr1*cos(q2)*cos(q3)*cos(q5)^2*sin(q4))/2000000 + dq1*dqr1*cos(q2)^2*cos(q3)^2*cos(q5)*sin(q4)*((1369*3^(1/2))/500000 - 45547/5000000) - (1369*3^(1/2)*dq4*dqr1*cos(q5)^2*sin(q2)*sin(q3)*sin(q4))/4000000 - (1369*3^(1/2)*dq5*dqr1*cos(q5)^2*sin(q2)*sin(q3)*sin(q4))/2000000 - dq1*dqr1*cos(q2)*cos(q3)^2*cos(q4)^2*sin(q2)*((23717*3^(1/2))/5000000 + 1232643/200000000) + dq1*dqr1*cos(q2)^2*cos(q3)*cos(q4)^2*sin(q3)*((23717*3^(1/2))/5000000 + 1232643/200000000) - (1369*dq1*dqr1*cos(q2)*cos(q3)^2*cos(q4)^2*cos(q5)^2*sin(q2))/400000 + (1369*dq1*dqr1*cos(q2)^2*cos(q3)*cos(q4)^2*cos(q5)^2*sin(q3))/400000 + (1073*dq1*dqr1*cos(q2)*cos(q4)*sin(q2)*sin(q3)*sin(q5))/50000 + (1073*dq1*dqr1*cos(q2)*cos(q5)*sin(q2)*sin(q3)*sin(q4))/100000 + dq4*dqr1*cos(q2)*cos(q3)*cos(q5)*sin(q4)*((1369*3^(1/2))/2000000 - 45547/20000000) - dq1*dqr1*cos(q2)*sin(q2)*sin(q3)*sin(q4)*((18589*3^(1/2))/1000000 + 1073/50000) + dq4*dqr1*cos(q5)*sin(q2)*sin(q3)*sin(q4)*((1369*3^(1/2))/2000000 - 45547/20000000) + (1073*3^(1/2)*dq1*dqr1*cos(q2)*cos(q3)*cos(q5)*sin(q2))/100000 + dq1*dqr1*cos(q2)*cos(q3)^2*cos(q4)^2*cos(q5)*sin(q2)*((23717*3^(1/2))/10000000 + 1369/500000) - dq1*dqr1*cos(q2)^2*cos(q3)*cos(q4)^2*cos(q5)*sin(q3)*((23717*3^(1/2))/10000000 + 1369/500000) - (32449*dq1*dqr1*cos(q2)*cos(q3)*cos(q4)*sin(q2)*sin(q3)*sin(q5))/1000000 - (1369*dq1*dqr1*cos(q2)*cos(q4)*cos(q5)*sin(q2)*sin(q4)*sin(q5))/1000000 + (1369*dq1*dqr1*cos(q3)*cos(q4)*cos(q5)*sin(q3)*sin(q4)*sin(q5))/1000000 - (1369*dq4*dqr1*cos(q2)*cos(q4)*cos(q5)*sin(q3)*sin(q4)*sin(q5))/1000000 + (1369*dq4*dqr1*cos(q3)*cos(q4)*cos(q5)*sin(q2)*sin(q4)*sin(q5))/1000000 - (1369*dq5*dqr1*cos(q2)*cos(q4)*cos(q5)*sin(q3)*sin(q4)*sin(q5))/800000 + (1369*dq5*dqr1*cos(q3)*cos(q4)*cos(q5)*sin(q2)*sin(q4)*sin(q5))/800000 + dq1*dqr1*cos(q2)*cos(q4)*sin(q2)*sin(q4)*sin(q5)*((23717*3^(1/2))/10000000 + 1369/500000) - dq1*dqr1*cos(q3)*cos(q4)*sin(q3)*sin(q4)*sin(q5)*((23717*3^(1/2))/10000000 + 1369/500000) + dq4*dqr1*cos(q2)*cos(q4)*sin(q3)*sin(q4)*sin(q5)*((23717*3^(1/2))/10000000 + 1369/500000) - dq4*dqr1*cos(q3)*cos(q4)*sin(q2)*sin(q4)*sin(q5)*((23717*3^(1/2))/10000000 + 1369/500000) + dq1*dqr1*cos(q2)*cos(q3)*sin(q2)*sin(q3)*sin(q4)*((562157*3^(1/2))/20000000 + 32449/1000000) + dq5*dqr1*cos(q2)*cos(q4)*sin(q3)*sin(q4)*sin(q5)*((23717*3^(1/2))/40000000 + 1369/2000000) - dq5*dqr1*cos(q3)*cos(q4)*sin(q2)*sin(q4)*sin(q5)*((23717*3^(1/2))/40000000 + 1369/2000000) - (1369*3^(1/2)*dq4*dqr1*cos(q4)*cos(q5)*sin(q2)*sin(q3)*sin(q5))/2000000 - (1369*3^(1/2)*dq5*dqr1*cos(q4)*cos(q5)*sin(q2)*sin(q3)*sin(q5))/4000000 - (1369*3^(1/2)*dq1*dqr1*cos(q2)*cos(q3)*cos(q5)^2*sin(q2)*sin(q3)*sin(q4))/1000000 + dq1*dqr1*cos(q2)*cos(q3)*cos(q5)*sin(q2)*sin(q3)*sin(q4)*((1369*3^(1/2))/500000 - 45547/5000000) + (1369*dq1*dqr1*cos(q2)*cos(q3)^2*cos(q4)*cos(q5)*sin(q2)*sin(q4)*sin(q5))/500000 - (1369*dq1*dqr1*cos(q2)^2*cos(q3)*cos(q4)*cos(q5)*sin(q3)*sin(q4)*sin(q5))/500000 - dq1*dqr1*cos(q2)*cos(q3)^2*cos(q4)*sin(q2)*sin(q4)*sin(q5)*((23717*3^(1/2))/5000000 + 1369/250000) + dq1*dqr1*cos(q2)^2*cos(q3)*cos(q4)*sin(q3)*sin(q4)*sin(q5)*((23717*3^(1/2))/5000000 + 1369/250000) - (1369*3^(1/2)*dq1*dqr1*cos(q2)*cos(q3)*cos(q4)*cos(q5)*sin(q2)*sin(q3)*sin(q5))/500000;
Y2_5_2=(25433*dq2*dqr3*sin(q3))/400000 + (25433*dq3*dqr2*sin(q3))/400000 - (25433*dq3*dqr3*sin(q3))/400000 - (1369*dq4*dqr2*sin(2*q5))/4000000 - (1369*dq5*dqr2*sin(2*q4))/4000000 + (1369*dq4*dqr3*sin(2*q5))/4000000 - (1369*dq5*dqr2*sin(2*q5))/2000000 + (1369*dq5*dqr3*sin(2*q4))/4000000 + (1369*dq5*dqr3*sin(2*q5))/2000000 - dq5*dqr2*sin(q5)*((4329*3^(1/2))/1250000 - 1369/2000000) + dq5*dqr3*sin(q5)*((4329*3^(1/2))/1250000 - 1369/2000000) + dq4*dqr2*sin(q5)*((23717*3^(1/2))/20000000 + 1369/1000000) - dq4*dqr3*sin(q5)*((23717*3^(1/2))/20000000 + 1369/1000000) + dq1*dqr1*sin(q4)*((562157*3^(1/2))/80000000 + 32449/4000000) - dq1*dqr1*sin(2*q2)*((23717*3^(1/2))/20000000 + 8096009/400000000) + dq1*dqr1*sin(2*q3)*((23717*3^(1/2))/20000000 - 8723991/400000000) + dq4*dqr2*sin(2*q4)*((23717*3^(1/2))/20000000 + 1232643/800000000) - dq4*dqr3*sin(2*q4)*((23717*3^(1/2))/20000000 + 1232643/800000000) - (32449*dq1*dqr1*cos(q4)*sin(q5))/4000000 + dq1*dqr1*cos(q5)*sin(q4)*((1369*3^(1/2))/2000000 - 45547/20000000) + (32449*dq1*dqr1*cos(q2)^2*cos(q4)*sin(q5))/2000000 + (32449*dq1*dqr1*cos(q3)^2*cos(q4)*sin(q5))/2000000 + (1369*dq1*dqr4*cos(q3)*cos(q5)^2*sin(q2))/4000000 + (1369*dq4*dqr2*cos(q4)*cos(q5)^2*sin(q4))/800000 + (1369*dq4*dqr2*cos(q4)^2*cos(q5)*sin(q5))/1000000 - (1369*dq4*dqr3*cos(q4)*cos(q5)^2*sin(q4))/800000 + (1369*dq5*dqr2*cos(q4)*cos(q5)^2*sin(q4))/1000000 - (1369*dq4*dqr3*cos(q4)^2*cos(q5)*sin(q5))/1000000 + (1369*dq5*dqr2*cos(q4)^2*cos(q5)*sin(q5))/800000 - (1369*dq5*dqr3*cos(q4)*cos(q5)^2*sin(q4))/1000000 - (1369*dq5*dqr3*cos(q4)^2*cos(q5)*sin(q5))/800000 + dq1*dqr4*cos(q3)*sin(q2)*((23717*3^(1/2))/10000000 + 1780243/400000000) + (1073*3^(1/2)*dq2*dqr3*cos(q5)*sin(q3))/200000 + (1073*3^(1/2)*dq3*dqr2*cos(q5)*sin(q3))/200000 - (1073*3^(1/2)*dq3*dqr3*cos(q5)*sin(q3))/200000 + (1073*3^(1/2)*dq5*dqr2*cos(q3)*sin(q5))/200000 - (1073*3^(1/2)*dq5*dqr3*cos(q3)*sin(q5))/200000 - dq4*dqr2*cos(q4)^2*sin(q5)*((23717*3^(1/2))/10000000 + 1369/500000) + dq4*dqr3*cos(q4)^2*sin(q5)*((23717*3^(1/2))/10000000 + 1369/500000) - dq5*dqr2*cos(q4)^2*sin(q5)*((23717*3^(1/2))/40000000 + 1369/2000000) + dq5*dqr3*cos(q4)^2*sin(q5)*((23717*3^(1/2))/40000000 + 1369/2000000) - dq1*dqr1*cos(q3)^2*sin(q4)*((562157*3^(1/2))/40000000 + 32449/2000000) - (1369*3^(1/2)*dq1*dqr1*cos(q5)^2*sin(q4))/4000000 - (1073*dq1*dqr1*cos(q3)*cos(q4)*sin(q5))/100000 - (1073*dq1*dqr1*cos(q3)*cos(q5)*sin(q4))/200000 + (1073*dq4*dqr1*cos(q2)*cos(q4)*sin(q5))/100000 - (1073*dq2*dqr3*cos(q3)*cos(q4)*sin(q5))/100000 - (1073*dq2*dqr3*cos(q3)*cos(q5)*sin(q4))/200000 - (1073*dq3*dqr2*cos(q3)*cos(q4)*sin(q5))/100000 - (1073*dq3*dqr2*cos(q3)*cos(q5)*sin(q4))/200000 + (1073*dq5*dqr1*cos(q2)*cos(q4)*sin(q5))/200000 + (1073*dq3*dqr3*cos(q3)*cos(q4)*sin(q5))/100000 + (1073*dq3*dqr3*cos(q3)*cos(q5)*sin(q4))/200000 - (1073*dq4*dqr2*cos(q4)*cos(q5)*sin(q3))/200000 + (1073*dq4*dqr3*cos(q4)*cos(q5)*sin(q3))/200000 - (1073*dq5*dqr2*cos(q4)*cos(q5)*sin(q3))/100000 + (1073*dq5*dqr3*cos(q4)*cos(q5)*sin(q3))/100000 + (1073*dq2*dqr4*sin(q3)*sin(q4)*sin(q5))/100000 + (1073*dq4*dqr2*sin(q3)*sin(q4)*sin(q5))/100000 - (1073*dq3*dqr4*sin(q3)*sin(q4)*sin(q5))/100000 - (1073*dq4*dqr3*sin(q3)*sin(q4)*sin(q5))/100000 + (1073*dq5*dqr2*sin(q3)*sin(q4)*sin(q5))/200000 - (1073*dq5*dqr3*sin(q3)*sin(q4)*sin(q5))/200000 + dq1*dqr1*cos(q3)*sin(q4)*((18589*3^(1/2))/2000000 + 1073/100000) + dq2*dqr3*cos(q3)*sin(q4)*((18589*3^(1/2))/2000000 + 1073/100000) + dq3*dqr2*cos(q3)*sin(q4)*((18589*3^(1/2))/2000000 + 1073/100000) - dq3*dqr3*cos(q3)*sin(q4)*((18589*3^(1/2))/2000000 + 1073/100000) + dq4*dqr2*cos(q4)*sin(q3)*((18589*3^(1/2))/2000000 + 1073/100000) - dq4*dqr3*cos(q4)*sin(q3)*((18589*3^(1/2))/2000000 + 1073/100000) - (1369*3^(1/2)*dq1*dqr1*cos(q4)*cos(q5)*sin(q5))/2000000 - dq1*dqr1*cos(q3)^2*cos(q5)*sin(q4)*((1369*3^(1/2))/1000000 - 45547/10000000) - (32449*dq1*dqr1*cos(q2)^2*cos(q3)^2*cos(q4)*sin(q5))/1000000 + (1369*dq1*dqr4*cos(q2)*cos(q4)^2*cos(q5)^2*sin(q3))/800000 - (1369*dq1*dqr4*cos(q3)*cos(q4)^2*cos(q5)^2*sin(q2))/800000 + dq1*dqr4*cos(q2)*cos(q4)^2*sin(q3)*((23717*3^(1/2))/10000000 + 1232643/400000000) - dq1*dqr4*cos(q3)*cos(q4)^2*sin(q2)*((23717*3^(1/2))/10000000 + 1232643/400000000) - (32449*dq4*dqr1*cos(q2)*cos(q3)*cos(q4)*sin(q5))/4000000 - (32449*dq5*dqr1*cos(q2)*cos(q3)*cos(q4)*sin(q5))/8000000 - (32449*dq1*dqr4*cos(q4)*sin(q2)*sin(q3)*sin(q5))/4000000 - dq1*dqr4*cos(q3)*cos(q5)*sin(q2)*((23717*3^(1/2))/20000000 + 1369/1000000) - dq4*dqr2*cos(q4)*cos(q5)*sin(q4)*((23717*3^(1/2))/20000000 + 1369/1000000) + dq4*dqr3*cos(q4)*cos(q5)*sin(q4)*((23717*3^(1/2))/20000000 + 1369/1000000) - dq5*dqr2*cos(q4)*cos(q5)*sin(q4)*((23717*3^(1/2))/20000000 + 1369/1000000) + dq5*dqr3*cos(q4)*cos(q5)*sin(q4)*((23717*3^(1/2))/20000000 + 1369/1000000) + (1073*dq1*dqr1*cos(q2)^2*cos(q3)*cos(q4)*sin(q5))/50000 + dq1*dqr4*sin(q2)*sin(q3)*sin(q4)*((562157*3^(1/2))/80000000 + 32449/4000000) - dq1*dqr4*cos(q2)*cos(q4)^2*cos(q5)*sin(q3)*((23717*3^(1/2))/20000000 + 1369/1000000) + dq1*dqr4*cos(q3)*cos(q4)^2*cos(q5)*sin(q2)*((23717*3^(1/2))/20000000 + 1369/1000000) + (1369*3^(1/2)*dq1*dqr1*cos(q2)^2*cos(q4)*cos(q5)*sin(q5))/1000000 + (1369*3^(1/2)*dq1*dqr1*cos(q3)^2*cos(q4)*cos(q5)*sin(q5))/1000000 - (1369*3^(1/2)*dq1*dqr4*cos(q5)^2*sin(q2)*sin(q3)*sin(q4))/4000000 + dq1*dqr4*cos(q5)*sin(q2)*sin(q3)*sin(q4)*((1369*3^(1/2))/2000000 - 45547/20000000) - (1369*dq1*dqr4*cos(q2)*cos(q4)*cos(q5)*sin(q3)*sin(q4)*sin(q5))/1000000 + (1369*dq1*dqr4*cos(q3)*cos(q4)*cos(q5)*sin(q2)*sin(q4)*sin(q5))/1000000 - (1369*3^(1/2)*dq1*dqr1*cos(q2)^2*cos(q3)^2*cos(q4)*cos(q5)*sin(q5))/500000 + dq1*dqr4*cos(q2)*cos(q4)*sin(q3)*sin(q4)*sin(q5)*((23717*3^(1/2))/10000000 + 1369/500000) - dq1*dqr4*cos(q3)*cos(q4)*sin(q2)*sin(q4)*sin(q5)*((23717*3^(1/2))/10000000 + 1369/500000) - (1369*3^(1/2)*dq4*dqr1*cos(q2)*cos(q3)*cos(q4)*cos(q5)*sin(q5))/2000000 - (1369*3^(1/2)*dq5*dqr1*cos(q2)*cos(q3)*cos(q4)*cos(q5)*sin(q5))/4000000 - (1369*3^(1/2)*dq1*dqr4*cos(q4)*cos(q5)*sin(q2)*sin(q3)*sin(q5))/2000000;
Y2_5_3=(1369*dq3*dqr4*sin(2*q5))/4000000 - (1369*dq2*dqr5*sin(2*q4))/4000000 - (1369*dq2*dqr5*sin(2*q5))/2000000 - (1369*dq2*dqr4*sin(2*q5))/4000000 + (1369*dq3*dqr5*sin(2*q4))/4000000 + (1369*dq3*dqr5*sin(2*q5))/2000000 - dq2*dqr5*sin(q5)*((4329*3^(1/2))/1250000 - 1369/2000000) + dq3*dqr5*sin(q5)*((4329*3^(1/2))/1250000 - 1369/2000000) + dq2*dqr4*sin(q5)*((23717*3^(1/2))/20000000 + 1369/1000000) - dq3*dqr4*sin(q5)*((23717*3^(1/2))/20000000 + 1369/1000000) + dq4*dqr4*sin(q4)*((562157*3^(1/2))/80000000 + 32449/4000000) + dq2*dqr4*sin(2*q4)*((23717*3^(1/2))/20000000 + 1232643/800000000) - dq3*dqr4*sin(2*q4)*((23717*3^(1/2))/20000000 + 1232643/800000000) - (32449*dq4*dqr4*cos(q4)*sin(q5))/4000000 - (32449*dq4*dqr5*cos(q4)*sin(q5))/8000000 - (32449*dq4*dqr5*cos(q5)*sin(q4))/4000000 - (32449*dq5*dqr4*cos(q4)*sin(q5))/8000000 - (32449*dq5*dqr4*cos(q5)*sin(q4))/4000000 - (32449*dq5*dqr5*cos(q4)*sin(q5))/4000000 - dq5*dqr5*cos(q5)*sin(q4)*((1369*3^(1/2))/2000000 + 58349/10000000) + dq4*dqr4*cos(q5)*sin(q4)*((1369*3^(1/2))/2000000 - 45547/20000000) - (1369*dq1*dqr4*cos(q2)*cos(q5)^2*sin(q3))/4000000 - (1369*dq1*dqr5*cos(q2)*cos(q4)^2*sin(q3))/2000000 + (1369*dq1*dqr5*cos(q3)*cos(q4)^2*sin(q2))/2000000 - (1369*dq1*dqr5*cos(q2)*cos(q5)^2*sin(q3))/2000000 + (1369*dq1*dqr5*cos(q3)*cos(q5)^2*sin(q2))/2000000 + (1369*dq2*dqr4*cos(q4)*cos(q5)^2*sin(q4))/800000 + (1369*dq2*dqr4*cos(q4)^2*cos(q5)*sin(q5))/1000000 + (1369*dq2*dqr5*cos(q4)*cos(q5)^2*sin(q4))/1000000 - (1369*dq3*dqr4*cos(q4)*cos(q5)^2*sin(q4))/800000 + (1369*dq2*dqr5*cos(q4)^2*cos(q5)*sin(q5))/800000 - (1369*dq3*dqr4*cos(q4)^2*cos(q5)*sin(q5))/1000000 - (1369*dq3*dqr5*cos(q4)*cos(q5)^2*sin(q4))/1000000 - (1369*dq3*dqr5*cos(q4)^2*cos(q5)*sin(q5))/800000 - dq1*dqr4*cos(q2)*sin(q3)*((23717*3^(1/2))/10000000 + 1780243/400000000) + (1073*3^(1/2)*dq2*dqr5*cos(q3)*sin(q5))/200000 - (1073*3^(1/2)*dq3*dqr5*cos(q3)*sin(q5))/200000 - (1073*3^(1/2)*dq5*dqr5*cos(q5)*sin(q3))/200000 - (32449*ddqr1*sin(q2)*sin(q3)*sin(q4)*sin(q5))/4000000 - dq2*dqr4*cos(q4)^2*sin(q5)*((23717*3^(1/2))/10000000 + 1369/500000) + dq3*dqr4*cos(q4)^2*sin(q5)*((23717*3^(1/2))/10000000 + 1369/500000) - dq2*dqr5*cos(q4)^2*sin(q5)*((23717*3^(1/2))/40000000 + 1369/2000000) + dq3*dqr5*cos(q4)^2*sin(q5)*((23717*3^(1/2))/40000000 + 1369/2000000) - (1369*3^(1/2)*dq4*dqr4*cos(q5)^2*sin(q4))/4000000 - (1369*3^(1/2)*dq4*dqr5*cos(q5)^2*sin(q4))/2000000 - (1369*3^(1/2)*dq5*dqr4*cos(q5)^2*sin(q4))/2000000 + (1073*dq1*dqr4*cos(q2)*cos(q4)*sin(q5))/100000 + (1073*dq1*dqr4*cos(q2)*cos(q5)*sin(q4))/200000 + (1073*dq1*dqr5*cos(q2)*cos(q4)*sin(q5))/200000 + (1073*dq1*dqr5*cos(q2)*cos(q5)*sin(q4))/100000 - (1073*dq2*dqr4*cos(q4)*cos(q5)*sin(q3))/200000 - (1073*dq2*dqr5*cos(q4)*cos(q5)*sin(q3))/100000 + (1073*dq3*dqr4*cos(q4)*cos(q5)*sin(q3))/200000 + (1073*dq3*dqr5*cos(q4)*cos(q5)*sin(q3))/100000 + (1073*dq4*dqr4*cos(q3)*cos(q4)*sin(q5))/100000 + (1073*dq4*dqr4*cos(q3)*cos(q5)*sin(q4))/200000 + (1073*dq4*dqr5*cos(q3)*cos(q4)*sin(q5))/200000 + (1073*dq4*dqr5*cos(q3)*cos(q5)*sin(q4))/100000 + (1073*dq5*dqr4*cos(q3)*cos(q4)*sin(q5))/200000 + (1073*dq5*dqr4*cos(q3)*cos(q5)*sin(q4))/100000 + (1073*dq5*dqr5*cos(q3)*cos(q4)*sin(q5))/100000 + (1073*dq5*dqr5*cos(q3)*cos(q5)*sin(q4))/200000 + (1073*dq2*dqr5*sin(q3)*sin(q4)*sin(q5))/200000 - (1073*dq3*dqr5*sin(q3)*sin(q4)*sin(q5))/200000 - dq1*dqr4*cos(q2)*sin(q4)*((18589*3^(1/2))/2000000 + 1073/100000) + dq2*dqr4*cos(q4)*sin(q3)*((18589*3^(1/2))/2000000 + 1073/100000) - dq3*dqr4*cos(q4)*sin(q3)*((18589*3^(1/2))/2000000 + 1073/100000) - dq4*dqr4*cos(q3)*sin(q4)*((18589*3^(1/2))/2000000 + 1073/100000) - (1369*3^(1/2)*dq4*dqr4*cos(q4)*cos(q5)*sin(q5))/2000000 - (1369*3^(1/2)*dq4*dqr5*cos(q4)*cos(q5)*sin(q5))/4000000 - (1369*3^(1/2)*dq5*dqr4*cos(q4)*cos(q5)*sin(q5))/4000000 + (1369*dq1*dqr5*cos(q2)*cos(q4)^2*cos(q5)^2*sin(q3))/1000000 - (1369*dq1*dqr5*cos(q3)*cos(q4)^2*cos(q5)^2*sin(q2))/1000000 - (32449*dq1*dqr4*cos(q2)*cos(q3)*cos(q4)*sin(q5))/4000000 - (32449*dq1*dqr5*cos(q2)*cos(q3)*cos(q4)*sin(q5))/8000000 - (32449*dq1*dqr5*cos(q2)*cos(q3)*cos(q5)*sin(q4))/4000000 - (32449*dq1*dqr5*cos(q4)*sin(q2)*sin(q3)*sin(q5))/8000000 - (32449*dq1*dqr5*cos(q5)*sin(q2)*sin(q3)*sin(q4))/4000000 + dq1*dqr4*cos(q2)*cos(q5)*sin(q3)*((23717*3^(1/2))/20000000 + 1369/1000000) + dq1*dqr5*cos(q2)*cos(q5)*sin(q3)*((23717*3^(1/2))/20000000 + 1369/1000000) - dq1*dqr5*cos(q3)*cos(q5)*sin(q2)*((23717*3^(1/2))/20000000 + 1369/1000000) - dq2*dqr4*cos(q4)*cos(q5)*sin(q4)*((23717*3^(1/2))/20000000 + 1369/1000000) - dq2*dqr5*cos(q4)*cos(q5)*sin(q4)*((23717*3^(1/2))/20000000 + 1369/1000000) + dq3*dqr4*cos(q4)*cos(q5)*sin(q4)*((23717*3^(1/2))/20000000 + 1369/1000000) + dq3*dqr5*cos(q4)*cos(q5)*sin(q4)*((23717*3^(1/2))/20000000 + 1369/1000000) + dq1*dqr4*cos(q2)*cos(q3)*sin(q4)*((562157*3^(1/2))/80000000 + 32449/4000000) - dq1*dqr5*cos(q2)*cos(q4)^2*cos(q5)*sin(q3)*((23717*3^(1/2))/20000000 + 1369/1000000) + dq1*dqr5*cos(q3)*cos(q4)^2*cos(q5)*sin(q2)*((23717*3^(1/2))/20000000 + 1369/1000000) - (1369*3^(1/2)*dq1*dqr4*cos(q2)*cos(q3)*cos(q5)^2*sin(q4))/4000000 - (1369*3^(1/2)*dq1*dqr5*cos(q2)*cos(q3)*cos(q5)^2*sin(q4))/2000000 - (1369*3^(1/2)*dq1*dqr5*cos(q5)^2*sin(q2)*sin(q3)*sin(q4))/2000000 - (1369*3^(1/2)*ddqr1*cos(q5)*sin(q2)*sin(q3)*sin(q4)*sin(q5))/2000000 + dq1*dqr4*cos(q2)*cos(q3)*cos(q5)*sin(q4)*((1369*3^(1/2))/2000000 - 45547/20000000) - (1369*dq1*dqr5*cos(q2)*cos(q4)*cos(q5)*sin(q3)*sin(q4)*sin(q5))/800000 + (1369*dq1*dqr5*cos(q3)*cos(q4)*cos(q5)*sin(q2)*sin(q4)*sin(q5))/800000 + dq1*dqr5*cos(q2)*cos(q4)*sin(q3)*sin(q4)*sin(q5)*((23717*3^(1/2))/40000000 + 1369/2000000) - dq1*dqr5*cos(q3)*cos(q4)*sin(q2)*sin(q4)*sin(q5)*((23717*3^(1/2))/40000000 + 1369/2000000) - (1369*3^(1/2)*dq1*dqr4*cos(q2)*cos(q3)*cos(q4)*cos(q5)*sin(q5))/2000000 - (1369*3^(1/2)*dq1*dqr5*cos(q2)*cos(q3)*cos(q4)*cos(q5)*sin(q5))/4000000 - (1369*3^(1/2)*dq1*dqr5*cos(q4)*cos(q5)*sin(q2)*sin(q3)*sin(q5))/4000000;
Y2_5_4=(25433*ddqr3*cos(q3))/400000 - (25433*ddqr2*cos(q3))/200000 - (203*ddqr1*cos(q2))/100000 - ddqr3*((23717*3^(1/2))/10000000 + 5252117/100000000) + ddqr2*((23717*3^(1/2))/10000000 + 13662117/100000000) + (1369*ddqr2*cos(q5)^2)/1000000 - (1369*ddqr3*cos(q5)^2)/1000000 - (1369*ddqr2*cos(q4)^2*cos(q5)^2)/800000 + (1369*ddqr3*cos(q4)^2*cos(q5)^2)/800000 - ddqr2*cos(q4)^2*((23717*3^(1/2))/10000000 + 1232643/400000000) + ddqr3*cos(q4)^2*((23717*3^(1/2))/10000000 + 1232643/400000000) + (6139*ddqr1*cos(q2)*cos(q3))/4000000 + (32449*ddqr5*cos(q4)*cos(q5))/4000000 + (6139*ddqr1*sin(q2)*sin(q3))/4000000 - (32449*ddqr4*sin(q4)*sin(q5))/4000000 + ddqr2*cos(q5)*((4329*3^(1/2))/625000 - 1369/1000000) - ddqr3*cos(q5)*((4329*3^(1/2))/625000 - 1369/1000000) - ddqr4*cos(q4)*((562157*3^(1/2))/80000000 + 32449/4000000) + (1369*3^(1/2)*ddqr5*cos(q4))/2000000 + (1369*3^(1/2)*ddqr4*cos(q4)*cos(q5)^2)/4000000 - (1073*ddqr1*cos(q2)*cos(q4)*cos(q5))/200000 - (1073*ddqr4*cos(q3)*cos(q4)*cos(q5))/200000 - (1073*ddqr5*cos(q3)*cos(q4)*cos(q5))/100000 + (1073*ddqr1*cos(q2)*sin(q4)*sin(q5))/100000 - (1073*ddqr2*cos(q4)*sin(q3)*sin(q5))/50000 - (1073*ddqr2*cos(q5)*sin(q3)*sin(q4))/100000 + (1073*ddqr3*cos(q4)*sin(q3)*sin(q5))/100000 + (1073*ddqr3*cos(q5)*sin(q3)*sin(q4))/200000 + (1073*ddqr4*cos(q3)*sin(q4)*sin(q5))/100000 + (1073*ddqr5*cos(q3)*sin(q4)*sin(q5))/200000 + ddqr1*cos(q2)*cos(q4)*((18589*3^(1/2))/2000000 + 1073/100000) + ddqr4*cos(q3)*cos(q4)*((18589*3^(1/2))/2000000 + 1073/100000) - ddqr4*cos(q4)*cos(q5)*((1369*3^(1/2))/2000000 - 45547/20000000) + ddqr2*sin(q3)*sin(q4)*((18589*3^(1/2))/1000000 + 1073/50000) - ddqr3*sin(q3)*sin(q4)*((18589*3^(1/2))/2000000 + 1073/100000) - ddqr5*sin(q4)*sin(q5)*((1369*3^(1/2))/2000000 + 58349/10000000) - (1073*3^(1/2)*ddqr2*cos(q3)*cos(q5))/100000 + (1073*3^(1/2)*ddqr3*cos(q3)*cos(q5))/200000 + ddqr2*cos(q4)^2*cos(q5)*((23717*3^(1/2))/20000000 + 1369/1000000) - ddqr3*cos(q4)^2*cos(q5)*((23717*3^(1/2))/20000000 + 1369/1000000) - (1073*3^(1/2)*ddqr5*sin(q3)*sin(q5))/200000 - (32449*ddqr1*cos(q2)*cos(q3)*sin(q4)*sin(q5))/4000000 + (259*ddqr1*cos(q2)*cos(q4)*sin(q3)*sin(q5))/1000000 + (259*ddqr1*cos(q2)*cos(q5)*sin(q3)*sin(q4))/2000000 - (259*ddqr1*cos(q3)*cos(q4)*sin(q2)*sin(q5))/1000000 - (259*ddqr1*cos(q3)*cos(q5)*sin(q2)*sin(q4))/2000000 - (1369*ddqr1*cos(q2)*cos(q5)*sin(q3)*sin(q5))/2000000 + (1369*ddqr1*cos(q3)*cos(q5)*sin(q2)*sin(q5))/2000000 + (1369*ddqr2*cos(q4)*cos(q5)*sin(q4)*sin(q5))/1000000 - (1369*ddqr3*cos(q4)*cos(q5)*sin(q4)*sin(q5))/1000000 - ddqr1*cos(q2)*cos(q3)*cos(q4)*((562157*3^(1/2))/80000000 + 32449/4000000) - ddqr2*cos(q4)*sin(q4)*sin(q5)*((23717*3^(1/2))/10000000 + 1369/500000) + ddqr3*cos(q4)*sin(q4)*sin(q5)*((23717*3^(1/2))/10000000 + 1369/500000) - ddqr1*cos(q2)*sin(q3)*sin(q4)*((4487*3^(1/2))/20000000 + 259/1000000) + ddqr1*cos(q3)*sin(q2)*sin(q4)*((4487*3^(1/2))/20000000 + 259/1000000) + ddqr1*cos(q2)*sin(q3)*sin(q5)*((23717*3^(1/2))/20000000 + 1369/1000000) - ddqr1*cos(q3)*sin(q2)*sin(q5)*((23717*3^(1/2))/20000000 + 1369/1000000) - ddqr1*cos(q4)*sin(q2)*sin(q3)*((562157*3^(1/2))/80000000 + 32449/4000000) + (259*3^(1/2)*ddqr1*cos(q2)*cos(q3)*cos(q5))/2000000 + (259*3^(1/2)*ddqr1*cos(q5)*sin(q2)*sin(q3))/2000000 - (1369*3^(1/2)*ddqr4*cos(q5)*sin(q4)*sin(q5))/2000000 - ddqr1*cos(q2)*cos(q3)*cos(q4)*cos(q5)*((1369*3^(1/2))/2000000 - 45547/20000000) - ddqr1*cos(q4)*cos(q5)*sin(q2)*sin(q3)*((1369*3^(1/2))/2000000 - 45547/20000000) + (1369*ddqr1*cos(q2)*cos(q4)*cos(q5)^2*sin(q3)*sin(q4))/800000 - (1369*ddqr1*cos(q3)*cos(q4)*cos(q5)^2*sin(q2)*sin(q4))/800000 + (1369*ddqr1*cos(q2)*cos(q4)^2*cos(q5)*sin(q3)*sin(q5))/1000000 - (1369*ddqr1*cos(q3)*cos(q4)^2*cos(q5)*sin(q2)*sin(q5))/1000000 + ddqr1*cos(q2)*cos(q4)*sin(q3)*sin(q4)*((23717*3^(1/2))/10000000 + 1232643/400000000) - ddqr1*cos(q3)*cos(q4)*sin(q2)*sin(q4)*((23717*3^(1/2))/10000000 + 1232643/400000000) - ddqr1*cos(q2)*cos(q4)^2*sin(q3)*sin(q5)*((23717*3^(1/2))/10000000 + 1369/500000) + ddqr1*cos(q3)*cos(q4)^2*sin(q2)*sin(q5)*((23717*3^(1/2))/10000000 + 1369/500000) + (1369*3^(1/2)*ddqr1*cos(q2)*cos(q3)*cos(q4)*cos(q5)^2)/4000000 + (1369*3^(1/2)*ddqr1*cos(q4)*cos(q5)^2*sin(q2)*sin(q3))/4000000 - ddqr1*cos(q2)*cos(q4)*cos(q5)*sin(q3)*sin(q4)*((23717*3^(1/2))/20000000 + 1369/1000000) + ddqr1*cos(q3)*cos(q4)*cos(q5)*sin(q2)*sin(q4)*((23717*3^(1/2))/20000000 + 1369/1000000) - (1369*3^(1/2)*ddqr1*cos(q2)*cos(q3)*cos(q5)*sin(q4)*sin(q5))/2000000;
Y2_6_1=-(ddqr1*cos(q2))/625;
Y2_7_1=(29*ddqr3*cos(q3))/100 - (29*ddqr2*cos(q3))/50 + (29*dq1*dqr1*sin(q3))/100 + (29*dq2*dqr3*sin(q3))/100 + (29*dq3*dqr2*sin(q3))/100 - (29*dq3*dqr3*sin(q3))/100 - (ddqr1*cos(q2)*cos(q3))/625 - (ddqr1*sin(q2)*sin(q3))/625 - (29*dq1*dqr1*cos(q2)^2*sin(q3))/50 + (29*dq1*dqr1*cos(q2)*cos(q3)*sin(q2))/50;
Y2_8_1=(1231*ddqr4*cos(q4))/10000 - (1231*dq1*dqr1*sin(q4))/10000 - (1231*dq4*dqr4*sin(q4))/10000 - (29*ddqr1*cos(q2)*cos(q4))/100 - (29*ddqr4*cos(q3)*cos(q4))/100 - (29*ddqr2*sin(q3)*sin(q4))/50 + (29*ddqr3*sin(q3)*sin(q4))/100 + (1231*dq1*dqr1*cos(q2)^2*sin(q4))/5000 + (1231*dq1*dqr1*cos(q3)^2*sin(q4))/5000 + (1231*ddqr1*cos(q2)*cos(q3)*cos(q4))/10000 + (7*ddqr1*cos(q2)*sin(q3)*sin(q4))/1000 - (7*ddqr1*cos(q3)*sin(q2)*sin(q4))/1000 + (1231*ddqr1*cos(q4)*sin(q2)*sin(q3))/10000 - (29*dq1*dqr1*cos(q3)*sin(q4))/100 + (29*dq1*dqr4*cos(q2)*sin(q4))/100 + (29*dq4*dqr1*cos(q2)*sin(q4))/100 - (29*dq2*dqr3*cos(q3)*sin(q4))/100 - (29*dq3*dqr2*cos(q3)*sin(q4))/100 - (29*dq2*dqr4*cos(q4)*sin(q3))/100 + (29*dq3*dqr3*cos(q3)*sin(q4))/100 - (29*dq4*dqr2*cos(q4)*sin(q3))/100 + (29*dq3*dqr4*cos(q4)*sin(q3))/100 + (29*dq4*dqr3*cos(q4)*sin(q3))/100 + (29*dq4*dqr4*cos(q3)*sin(q4))/100 + (29*dq1*dqr1*cos(q2)^2*cos(q3)*sin(q4))/50 - (1231*dq1*dqr1*cos(q2)^2*cos(q3)^2*sin(q4))/2500 - (1231*dq1*dqr4*cos(q2)*cos(q3)*sin(q4))/10000 - (1231*dq4*dqr1*cos(q2)*cos(q3)*sin(q4))/10000 - (1231*dq1*dqr4*sin(q2)*sin(q3)*sin(q4))/10000 - (1231*dq4*dqr1*sin(q2)*sin(q3)*sin(q4))/10000 + (29*dq1*dqr1*cos(q2)*sin(q2)*sin(q3)*sin(q4))/50 - (1231*dq1*dqr1*cos(q2)*cos(q3)*sin(q2)*sin(q3)*sin(q4))/2500;
